simulink model "KUKA_LBR_Simulink_model_flatness_based_control"  (R2017a)
settings: Solver=VariableStepAuto  StartTime=0.0  StopTime=T  RelTol=1e-3
InitFcn:
  | main
values from neighbouring files (symbols this model uses):
  elbowAngle = elbowAngle * pi/180    (= 0)    [KUKA_LBR_init.m]    (also in Untitled2.m)
  KAnaJacNum = [k_ind 0 0 0 0 0 ;                 0  k_ind 0 0 0 0 ;                    0 0 k_ind 0 0 0 ;                      0 0 0 k_ind 0 0 ;                        0 0 0 0 k_ind 0 ;                          0 0 0 0 0 k_ind ;                            ]    [KUKA_LBR_init.m]
  Kuka_LBR_param_simu = Simulink.Parameter(Kuka_LBR_param_simu)    [KUKA_LBR_init.m]
  KUKA_LBR_x0 = [x1_0 x2_0 x3_0 x4_0 x5_0 x6_0 x7_0 x8_0 x9_0 x10_0 x11_0 x12_0 x13_0 x14_0]    [KUKA_LBR_init.m]
  rpyDes = rpyDes * pi/180    [KUKA_LBR_init.m]    (also in Untitled2.m)
  T = 0.5    [KUKA_LBR_init.m]
  vecGlobalConfig = [1; 1; 1]    [KUKA_LBR_init.m]    (also in Untitled2.m = [1, 1, 1])
undefined symbols (not defined in the file or in its folder): Kuka_LBR_param
(part 2 of 19)

== matlab function KUKA_LBR_Simulink_model_flatness_based_control/KUKUA_LBR_inverse_differentiell_kinematic ==
  data: vecJointPosDes_ input; rpyDes_ input; vecPosDes_ input; vecVelDes_ input; vecAccDes_ input; vecJointVelReal_ input; vecPosReal_ input; Kuka_LBR_param_ input; vecJointPos output; vecJointVel output; vecJointAcc output; KAnaJacP_ input; KAnaJacD_ input
function [vecJointPos,vecJointVel,vecJointAcc] = KUKUA_LBR_inverse_differentiell_kinematic(vecJointPosDes_,rpyDes_,vecPosDes_, vecVelDes_, vecAccDes_,vecJointVelReal_,vecPosReal_,Kuka_LBR_param_,KAnaJacP_,KAnaJacD_)

 
q1 = vecJointPosDes_(1,1) * pi/180;
q2 = vecJointPosDes_(1,2) * pi/180;
q3 = vecJointPosDes_(1,3) * pi/180;
q4 = vecJointPosDes_(1,4) * pi/180;
q5 = vecJointPosDes_(1,5) * pi/180;
q6 = vecJointPosDes_(1,6) * pi/180;
q7 = vecJointPosDes_(1,7) * pi/180;


Jxe11 = (-1).*Kuka_LBR_param_.dblLink23Len.*sin(q1).*sin(q2)+Kuka_LBR_param_.dblLink45Len.*((-1).*cos(q4).*sin(q1).*sin(q2)+(-1) ...
  .*((-1).*cos(q2).*cos(q3).*sin(q1)+(-1).*cos(q1).*sin(q3)).*sin(q4))+ ...
  Kuka_LBR_param_.dblLink67Len.*((-1).*cos(q6).*(cos(q4).*sin(q1).*sin(q2)+((-1).*cos(q2).*cos(q3) ...
  .*sin(q1)+(-1).*cos(q1).*sin(q3)).*sin(q4))+(cos(q5).*(cos(q4).*((-1).* ...
  cos(q2).*cos(q3).*sin(q1)+(-1).*cos(q1).*sin(q3))+(-1).*sin(q1).*sin(q2) ...
  .*sin(q4))+((-1).*cos(q1).*cos(q3)+cos(q2).*sin(q1).*sin(q3)).*sin(q5)) ...
  .*sin(q6));
  
Jxe12 =  Kuka_LBR_param_.dblLink23Len.*cos(q1).*cos(q2)+Kuka_LBR_param_.dblLink45Len.*(cos(q1).*cos(q2).*cos(q4)+cos(q1) ...
  .*cos(q3).*sin(q2).*sin(q4))+Kuka_LBR_param_.dblLink67Len.*((-1).*cos(q6).*((-1).*cos(q1).*cos( ...
  q2).*cos(q4)+(-1).*cos(q1).*cos(q3).*sin(q2).*sin(q4))+(cos(q5).*((-1).* ...
  cos(q1).*cos(q3).*cos(q4).*sin(q2)+cos(q1).*cos(q2).*sin(q4))+cos(q1).* ...
  sin(q2).*sin(q3).*sin(q5)).*sin(q6));
  
Jxe13 = (-1).*Kuka_LBR_param_.dblLink45Len.*((-1).*cos(q3).*sin(q1)+ ...
  (-1).*cos(q1).*cos(q2).*sin(q3)).*sin(q4)+Kuka_LBR_param_.dblLink67Len.*((-1).*cos(q6).*((-1).* ...
  cos(q3).*sin(q1)+(-1).*cos(q1).*cos(q2).*sin(q3)).*sin(q4)+(cos(q4).* ...
  cos(q5).*((-1).*cos(q3).*sin(q1)+(-1).*cos(q1).*cos(q2).*sin(q3))+((-1) ...
  .*cos(q1).*cos(q2).*cos(q3)+sin(q1).*sin(q3)).*sin(q5)).*sin(q6));
  
Jxe14 = Kuka_LBR_param_.dblLink45Len.*( ...
  (-1).*cos(q4).*(cos(q1).*cos(q2).*cos(q3)+(-1).*sin(q1).*sin(q3))+(-1).* ...
  cos(q1).*sin(q2).*sin(q4))+Kuka_LBR_param_.dblLink67Len.*((-1).*cos(q6).*(cos(q4).*(cos(q1).*cos( ...
  q2).*cos(q3)+(-1).*sin(q1).*sin(q3))+cos(q1).*sin(q2).*sin(q4))+cos(q5) ...
  .*(cos(q1).*cos(q4).*sin(q2)+(-1).*(cos(q1).*cos(q2).*cos(q3)+(-1).*sin( ...
  q1).*sin(q3)).*sin(q4)).*sin(q6));
  
Jxe15 = Kuka_LBR_param_.dblLink67Len.*(cos(q5).*((-1).*cos(q3).*sin(q1) ...
  +(-1).*cos(q1).*cos(q2).*sin(q3))+(-1).*(cos(q4).*(cos(q1).*cos(q2).* ...
  cos(q3)+(-1).*sin(q1).*sin(q3))+cos(q1).*sin(q2).*sin(q4)).*sin(q5)).* ...
  sin(q6);
  
Jxe16 = Kuka_LBR_param_.dblLink67Len.*(cos(q6).*(cos(q5).*(cos(q4).*(cos(q1).*cos(q2).*cos(q3)+( ...
  -1).*sin(q1).*sin(q3))+cos(q1).*sin(q2).*sin(q4))+((-1).*cos(q3).*sin( ...
  q1)+(-1).*cos(q1).*cos(q2).*sin(q3)).*sin(q5))+((-1).*cos(q1).*cos(q4).* ...
  sin(q2)+(cos(q1).*cos(q2).*cos(q3)+(-1).*sin(q1).*sin(q3)).*sin(q4)).* ...
  sin(q6));
  
 Jxe17= 0;
  
 Jxe21 = Kuka_LBR_param_.dblLink23Len.*cos(q1).*sin(q2)+Kuka_LBR_param_.dblLink45Len.*(cos(q1).*cos(q4).*sin(q2)+(-1).*( ...
  cos(q1).*cos(q2).*cos(q3)+(-1).*sin(q1).*sin(q3)).*sin(q4))+Kuka_LBR_param_.dblLink67Len.*((-1).* ...
  cos(q6).*((-1).*cos(q1).*cos(q4).*sin(q2)+(cos(q1).*cos(q2).*cos(q3)+( ...
  -1).*sin(q1).*sin(q3)).*sin(q4))+(cos(q5).*(cos(q4).*(cos(q1).*cos(q2).* ...
  cos(q3)+(-1).*sin(q1).*sin(q3))+cos(q1).*sin(q2).*sin(q4))+((-1).*cos( ...
  q3).*sin(q1)+(-1).*cos(q1).*cos(q2).*sin(q3)).*sin(q5)).*sin(q6));
  
  Jxe22 = Kuka_LBR_param_.dblLink23Len.* ...
  cos(q2).*sin(q1)+Kuka_LBR_param_.dblLink45Len.*(cos(q2).*cos(q4).*sin(q1)+cos(q3).*sin(q1).*sin( ...
  q2).*sin(q4))+Kuka_LBR_param_.dblLink67Len.*((-1).*cos(q6).*((-1).*cos(q2).*cos(q4).*sin(q1)+(-1) ...
  .*cos(q3).*sin(q1).*sin(q2).*sin(q4))+(cos(q5).*((-1).*cos(q3).*cos(q4) ...
  .*sin(q1).*sin(q2)+cos(q2).*sin(q1).*sin(q4))+sin(q1).*sin(q2).*sin(q3) ...
  .*sin(q5)).*sin(q6));
  
  Jxe23 = (-1).*Kuka_LBR_param_.dblLink45Len.*(cos(q1).*cos(q3)+(-1).*cos(q2).*sin(q1) ...
  .*sin(q3)).*sin(q4)+Kuka_LBR_param_.dblLink67Len.*((-1).*cos(q6).*(cos(q1).*cos(q3)+(-1).*cos(q2) ...
  .*sin(q1).*sin(q3)).*sin(q4)+(cos(q4).*cos(q5).*(cos(q1).*cos(q3)+(-1).* ...
  cos(q2).*sin(q1).*sin(q3))+((-1).*cos(q2).*cos(q3).*sin(q1)+(-1).*cos( ...
  q1).*sin(q3)).*sin(q5)).*sin(q6));
  
  Jxe24 = Kuka_LBR_param_.dblLink45Len.*((-1).*cos(q4).*(cos(q2).*cos(q3) ...
  .*sin(q1)+cos(q1).*sin(q3))+(-1).*sin(q1).*sin(q2).*sin(q4))+Kuka_LBR_param_.dblLink67Len.*((-1) ...
  .*cos(q6).*(cos(q4).*(cos(q2).*cos(q3).*sin(q1)+cos(q1).*sin(q3))+sin( ...
  q1).*sin(q2).*sin(q4))+cos(q5).*(cos(q4).*sin(q1).*sin(q2)+(-1).*(cos( ...
  q2).*cos(q3).*sin(q1)+cos(q1).*sin(q3)).*sin(q4)).*sin(q6));
  
  Jxe25 = Kuka_LBR_param_.dblLink67Len.*(cos( ...
  q5).*(cos(q1).*cos(q3)+(-1).*cos(q2).*sin(q1).*sin(q3))+(-1).*(cos(q4).* ...
  (cos(q2).*cos(q3).*sin(q1)+cos(q1).*sin(q3))+sin(q1).*sin(q2).*sin(q4)) ...
  .*sin(q5)).*sin(q6);
  
  Jxe26 = Kuka_LBR_param_.dblLink67Len.*(cos(q6).*(cos(q5).*(cos(q4).*(cos(q2).*cos(q3) ...
  .*sin(q1)+cos(q1).*sin(q3))+sin(q1).*sin(q2).*sin(q4))+(cos(q1).*cos(q3) ...
  +(-1).*cos(q2).*sin(q1).*sin(q3)).*sin(q5))+((-1).*cos(q4).*sin(q1).* ...
  sin(q2)+(cos(q2).*cos(q3).*sin(q1)+cos(q1).*sin(q3)).*sin(q4)).*sin(q6)); ...
  
  Jxe27 = 0;
  
  Jxe31 = 0;
  
  Jxe32 = (-1).*Kuka_LBR_param_.dblLink23Len.*sin(q2)+Kuka_LBR_param_.dblLink45Len.*((-1).*cos(q4).*sin(q2)+cos(q2).*cos(q3).* ...
  sin(q4))+Kuka_LBR_param_.dblLink67Len.*((-1).*cos(q6).*(cos(q4).*sin(q2)+(-1).*cos(q2).*cos(q3).* ...
  sin(q4))+(cos(q5).*((-1).*cos(q2).*cos(q3).*cos(q4)+(-1).*sin(q2).*sin( ...
  q4))+cos(q2).*sin(q3).*sin(q5)).*sin(q6));
  
  Jxe33 = (-1).*Kuka_LBR_param_.dblLink45Len.*sin(q2).*sin(q3).* ...
  sin(q4)+Kuka_LBR_param_.dblLink67Len.*((-1).*cos(q6).*sin(q2).*sin(q3).*sin(q4)+(cos(q4).*cos(q5) ...
  .*sin(q2).*sin(q3)+cos(q3).*sin(q2).*sin(q5)).*sin(q6));
  
  Jxe34 = Kuka_LBR_param_.dblLink45Len.*(cos(q3).* ...
  cos(q4).*sin(q2)+(-1).*cos(q2).*sin(q4))+Kuka_LBR_param_.dblLink67Len.*((-1).*cos(q6).*((-1).* ...
  cos(q3).*cos(q4).*sin(q2)+cos(q2).*sin(q4))+cos(q5).*(cos(q2).*cos(q4)+ ...
  cos(q3).*sin(q2).*sin(q4)).*sin(q6));
  
  Jxe35 = Kuka_LBR_param_.dblLink67Len.*(cos(q5).*sin(q2).*sin(q3)+( ...
  -1).*((-1).*cos(q3).*cos(q4).*sin(q2)+cos(q2).*sin(q4)).*sin(q5)).*sin( ...
  q6);
  
  Jxe36 = Kuka_LBR_param_.dblLink67Len.*(cos(q6).*(cos(q5).*((-1).*cos(q3).*cos(q4).*sin(q2)+cos(q2).* ...
  sin(q4))+sin(q2).*sin(q3).*sin(q5))+((-1).*cos(q2).*cos(q4)+(-1).*cos( ...
  q3).*sin(q2).*sin(q4)).*sin(q6));
  
  Jxe37 = 0;
  
  Jxe41 = (1+(-1).*(cos(q7).*(cos(q6).*(cos(q5) ...
  .*(cos(q4).*(cos(q1).*cos(q2).*cos(q3)+(-1).*sin(q1).*sin(q3))+cos(q1).* ...
  sin(q2).*sin(q4))+((-1).*cos(q3).*sin(q1)+(-1).*cos(q1).*cos(q2).*sin( ...
  q3)).*sin(q5))+((-1).*cos(q1).*cos(q4).*sin(q2)+(cos(q1).*cos(q2).*cos( ...
  q3)+(-1).*sin(q1).*sin(q3)).*sin(q4)).*sin(q6))+(cos(q5).*((-1).*cos(q3) ...
  .*sin(q1)+(-1).*cos(q1).*cos(q2).*sin(q3))+(-1).*(cos(q4).*(cos(q1).* ...
  cos(q2).*cos(q3)+(-1).*sin(q1).*sin(q3))+cos(q1).*sin(q2).*sin(q4)).* ...
  sin(q5)).*sin(q7)).^(-2).*(cos(q7).*(cos(q6).*(cos(q5).*(cos(q4).*((-1) ...
  .*cos(q2).*cos(q3).*sin(q1)+(-1).*cos(q1).*sin(q3))+(-1).*sin(q1).*sin( ...
  q2).*sin(q4))+((-1).*cos(q1).*cos(q3)+cos(q2).*sin(q1).*sin(q3)).*sin( ...
  q5))+(cos(q4).*sin(q1).*sin(q2)+((-1).*cos(q2).*cos(q3).*sin(q1)+(-1).* ...
  cos(q1).*sin(q3)).*sin(q4)).*sin(q6))+(cos(q5).*((-1).*cos(q1).*cos(q3)+ ...
  cos(q2).*sin(q1).*sin(q3))+(-1).*(cos(q4).*((-1).*cos(q2).*cos(q3).*sin( ...
  q1)+(-1).*cos(q1).*sin(q3))+(-1).*sin(q1).*sin(q2).*sin(q4)).*sin(q5)).* ...
  sin(q7)).*(cos(q7).*(cos(q6).*(cos(q5).*(cos(q4).*(cos(q2).*cos(q3).* ...
  sin(q1)+cos(q1).*sin(q3))+sin(q1).*sin(q2).*sin(q4))+(cos(q1).*cos(q3)+( ...
  -1).*cos(q2).*sin(q1).*sin(q3)).*sin(q5))+((-1).*cos(q4).*sin(q1).*sin( ...
  q2)+(cos(q2).*cos(q3).*sin(q1)+cos(q1).*sin(q3)).*sin(q4)).*sin(q6))+( ...
  cos(q5).*(cos(q1).*cos(q3)+(-1).*cos(q2).*sin(q1).*sin(q3))+(-1).*(cos( ...
  q4).*(cos(q2).*cos(q3).*sin(q1)+cos(q1).*sin(q3))+sin(q1).*sin(q2).*sin( ...
  q4)).*sin(q5)).*sin(q7)))*(1+(cos(q7).*(cos(q6).*(cos(q5).*(cos(q4).*( ...
  cos(q1).*cos(q2).*cos(q3)+(-1).*sin(q1).*sin(q3))+cos(q1).*sin(q2).*sin( ...
  q4))+((-1).*cos(q3).*sin(q1)+(-1).*cos(q1).*cos(q2).*sin(q3)).*sin(q5))+ ...
  ((-1).*cos(q1).*cos(q4).*sin(q2)+(cos(q1).*cos(q2).*cos(q3)+(-1).*sin( ...
  q1).*sin(q3)).*sin(q4)).*sin(q6))+(cos(q5).*((-1).*cos(q3).*sin(q1)+(-1) ...
  .*cos(q1).*cos(q2).*sin(q3))+(-1).*(cos(q4).*(cos(q1).*cos(q2).*cos(q3)+ ...
  (-1).*sin(q1).*sin(q3))+cos(q1).*sin(q2).*sin(q4)).*sin(q5)).*sin(q7)) ...
  .^(-2).*(cos(q7).*(cos(q6).*(cos(q5).*(cos(q4).*(cos(q2).*cos(q3).*sin( ...
  q1)+cos(q1).*sin(q3))+sin(q1).*sin(q2).*sin(q4))+(cos(q1).*cos(q3)+(-1) ...
  .*cos(q2).*sin(q1).*sin(q3)).*sin(q5))+((-1).*cos(q4).*sin(q1).*sin(q2)+ ...
  (cos(q2).*cos(q3).*sin(q1)+cos(q1).*sin(q3)).*sin(q4)).*sin(q6))+(cos( ...
  q5).*(cos(q1).*cos(q3)+(-1).*cos(q2).*sin(q1).*sin(q3))+(-1).*(cos(q4).* ...
  (cos(q2).*cos(q3).*sin(q1)+cos(q1).*sin(q3))+sin(q1).*sin(q2).*sin(q4)) ...
  .*sin(q5)).*sin(q7)).^2).^(-1);
  
  Jxe42 = ((cos(q7).*(cos(q6).*(cos(q5).*((-1).* ...
  cos(q3).*cos(q4).*sin(q1).*sin(q2)+cos(q2).*sin(q1).*sin(q4))+sin(q1).* ...
  sin(q2).*sin(q3).*sin(q5))+((-1).*cos(q2).*cos(q4).*sin(q1)+(-1).*cos( ...
  q3).*sin(q1).*sin(q2).*sin(q4)).*sin(q6))+(cos(q5).*sin(q1).*sin(q2).* ...
  sin(q3)+(-1).*((-1).*cos(q3).*cos(q4).*sin(q1).*sin(q2)+cos(q2).*sin(q1) ...
  .*sin(q4)).*sin(q5)).*sin(q7)).*(cos(q7).*(cos(q6).*(cos(q5).*(cos(q4).* ...
  (cos(q1).*cos(q2).*cos(q3)+(-1).*sin(q1).*sin(q3))+cos(q1).*sin(q2).* ...
  sin(q4))+((-1).*cos(q3).*sin(q1)+(-1).*cos(q1).*cos(q2).*sin(q3)).*sin( ...
  q5))+((-1).*cos(q1).*cos(q4).*sin(q2)+(cos(q1).*cos(q2).*cos(q3)+(-1).* ...
  sin(q1).*sin(q3)).*sin(q4)).*sin(q6))+(cos(q5).*((-1).*cos(q3).*sin(q1)+ ...
  (-1).*cos(q1).*cos(q2).*sin(q3))+(-1).*(cos(q4).*(cos(q1).*cos(q2).*cos( ...
  q3)+(-1).*sin(q1).*sin(q3))+cos(q1).*sin(q2).*sin(q4)).*sin(q5)).*sin( ...
  q7)).^(-1)+(-1).*(cos(q7).*(cos(q6).*(cos(q5).*((-1).*cos(q1).*cos(q3).* ...
  cos(q4).*sin(q2)+cos(q1).*cos(q2).*sin(q4))+cos(q1).*sin(q2).*sin(q3).* ...
  sin(q5))+((-1).*cos(q1).*cos(q2).*cos(q4)+(-1).*cos(q1).*cos(q3).*sin( ...
  q2).*sin(q4)).*sin(q6))+(cos(q1).*cos(q5).*sin(q2).*sin(q3)+(-1).*((-1) ...
  .*cos(q1).*cos(q3).*cos(q4).*sin(q2)+cos(q1).*cos(q2).*sin(q4)).*sin(q5) ...
  ).*sin(q7)).*(cos(q7).*(cos(q6).*(cos(q5).*(cos(q4).*(cos(q1).*cos(q2).* ...
  cos(q3)+(-1).*sin(q1).*sin(q3))+cos(q1).*sin(q2).*sin(q4))+((-1).*cos( ...
  q3).*sin(q1)+(-1).*cos(q1).*cos(q2).*sin(q3)).*sin(q5))+((-1).*cos(q1).* ...
  cos(q4).*sin(q2)+(cos(q1).*cos(q2).*cos(q3)+(-1).*sin(q1).*sin(q3)).* ...
  sin(q4)).*sin(q6))+(cos(q5).*((-1).*cos(q3).*sin(q1)+(-1).*cos(q1).*cos( ...
  q2).*sin(q3))+(-1).*(cos(q4).*(cos(q1).*cos(q2).*cos(q3)+(-1).*sin(q1).* ...
  sin(q3))+cos(q1).*sin(q2).*sin(q4)).*sin(q5)).*sin(q7)).^(-2).*(cos(q7) ...
  .*(cos(q6).*(cos(q5).*(cos(q4).*(cos(q2).*cos(q3).*sin(q1)+cos(q1).*sin( ...
  q3))+sin(q1).*sin(q2).*sin(q4))+(cos(q1).*cos(q3)+(-1).*cos(q2).*sin(q1) ...
  .*sin(q3)).*sin(q5))+((-1).*cos(q4).*sin(q1).*sin(q2)+(cos(q2).*cos(q3) ...
  .*sin(q1)+cos(q1).*sin(q3)).*sin(q4)).*sin(q6))+(cos(q5).*(cos(q1).*cos( ...
  q3)+(-1).*cos(q2).*sin(q1).*sin(q3))+(-1).*(cos(q4).*(cos(q2).*cos(q3).* ...
  sin(q1)+cos(q1).*sin(q3))+sin(q1).*sin(q2).*sin(q4)).*sin(q5)).*sin(q7)) ...
  ).*(1+(cos(q7).*(cos(q6).*(cos(q5).*(cos(q4).*(cos(q1).*cos(q2).*cos(q3) ...
  +(-1).*sin(q1).*sin(q3))+cos(q1).*sin(q2).*sin(q4))+((-1).*cos(q3).*sin( ...
  q1)+(-1).*cos(q1).*cos(q2).*sin(q3)).*sin(q5))+((-1).*cos(q1).*cos(q4).* ...
  sin(q2)+(cos(q1).*cos(q2).*cos(q3)+(-1).*sin(q1).*sin(q3)).*sin(q4)).* ...
  sin(q6))+(cos(q5).*((-1).*cos(q3).*sin(q1)+(-1).*cos(q1).*cos(q2).*sin( ...
  q3))+(-1).*(cos(q4).*(cos(q1).*cos(q2).*cos(q3)+(-1).*sin(q1).*sin(q3))+ ...
  cos(q1).*sin(q2).*sin(q4)).*sin(q5)).*sin(q7)).^(-2).*(cos(q7).*(cos(q6) ...
  .*(cos(q5).*(cos(q4).*(cos(q2).*cos(q3).*sin(q1)+cos(q1).*sin(q3))+sin( ...
  q1).*sin(q2).*sin(q4))+(cos(q1).*cos(q3)+(-1).*cos(q2).*sin(q1).*sin(q3) ...
  ).*sin(q5))+((-1).*cos(q4).*sin(q1).*sin(q2)+(cos(q2).*cos(q3).*sin(q1)+ ...
  cos(q1).*sin(q3)).*sin(q4)).*sin(q6))+(cos(q5).*(cos(q1).*cos(q3)+(-1).* ...
  cos(q2).*sin(q1).*sin(q3))+(-1).*(cos(q4).*(cos(q2).*cos(q3).*sin(q1)+ ...
  cos(q1).*sin(q3))+sin(q1).*sin(q2).*sin(q4)).*sin(q5)).*sin(q7)).^2).^( ...
  -1);
  
  Jxe43 = ((cos(q7).*(cos(q6).*(cos(q4).*cos(q5).*(cos(q1).*cos(q3)+(-1).*cos( ...
  q2).*sin(q1).*sin(q3))+((-1).*cos(q2).*cos(q3).*sin(q1)+(-1).*cos(q1).* ...
  sin(q3)).*sin(q5))+(cos(q1).*cos(q3)+(-1).*cos(q2).*sin(q1).*sin(q3)).* ...
  sin(q4).*sin(q6))+(cos(q5).*((-1).*cos(q2).*cos(q3).*sin(q1)+(-1).*cos( ...
  q1).*sin(q3))+(-1).*cos(q4).*(cos(q1).*cos(q3)+(-1).*cos(q2).*sin(q1).* ...
  sin(q3)).*sin(q5)).*sin(q7)).*(cos(q7).*(cos(q6).*(cos(q5).*(cos(q4).*( ...
  cos(q1).*cos(q2).*cos(q3)+(-1).*sin(q1).*sin(q3))+cos(q1).*sin(q2).*sin( ...
  q4))+((-1).*cos(q3).*sin(q1)+(-1).*cos(q1).*cos(q2).*sin(q3)).*sin(q5))+ ...
  ((-1).*cos(q1).*cos(q4).*sin(q2)+(cos(q1).*cos(q2).*cos(q3)+(-1).*sin( ...
  q1).*sin(q3)).*sin(q4)).*sin(q6))+(cos(q5).*((-1).*cos(q3).*sin(q1)+(-1) ...
  .*cos(q1).*cos(q2).*sin(q3))+(-1).*(cos(q4).*(cos(q1).*cos(q2).*cos(q3)+ ...
  (-1).*sin(q1).*sin(q3))+cos(q1).*sin(q2).*sin(q4)).*sin(q5)).*sin(q7)) ...
  .^(-1)+(-1).*(cos(q7).*(cos(q6).*(cos(q4).*cos(q5).*((-1).*cos(q3).*sin( ...
  q1)+(-1).*cos(q1).*cos(q2).*sin(q3))+((-1).*cos(q1).*cos(q2).*cos(q3)+ ...
  sin(q1).*sin(q3)).*sin(q5))+((-1).*cos(q3).*sin(q1)+(-1).*cos(q1).*cos( ...
  q2).*sin(q3)).*sin(q4).*sin(q6))+(cos(q5).*((-1).*cos(q1).*cos(q2).*cos( ...
  q3)+sin(q1).*sin(q3))+(-1).*cos(q4).*((-1).*cos(q3).*sin(q1)+(-1).*cos( ...
  q1).*cos(q2).*sin(q3)).*sin(q5)).*sin(q7)).*(cos(q7).*(cos(q6).*(cos(q5) ...
  .*(cos(q4).*(cos(q1).*cos(q2).*cos(q3)+(-1).*sin(q1).*sin(q3))+cos(q1).* ...
  sin(q2).*sin(q4))+((-1).*cos(q3).*sin(q1)+(-1).*cos(q1).*cos(q2).*sin( ...
  q3)).*sin(q5))+((-1).*cos(q1).*cos(q4).*sin(q2)+(cos(q1).*cos(q2).*cos( ...
  q3)+(-1).*sin(q1).*sin(q3)).*sin(q4)).*sin(q6))+(cos(q5).*((-1).*cos(q3) ...
  .*sin(q1)+(-1).*cos(q1).*cos(q2).*sin(q3))+(-1).*(cos(q4).*(cos(q1).* ...
  cos(q2).*cos(q3)+(-1).*sin(q1).*sin(q3))+cos(q1).*sin(q2).*sin(q4)).* ...
  sin(q5)).*sin(q7)).^(-2).*(cos(q7).*(cos(q6).*(cos(q5).*(cos(q4).*(cos( ...
  q2).*cos(q3).*sin(q1)+cos(q1).*sin(q3))+sin(q1).*sin(q2).*sin(q4))+(cos( ...
  q1).*cos(q3)+(-1).*cos(q2).*sin(q1).*sin(q3)).*sin(q5))+((-1).*cos(q4).* ...
  sin(q1).*sin(q2)+(cos(q2).*cos(q3).*sin(q1)+cos(q1).*sin(q3)).*sin(q4)) ...
  .*sin(q6))+(cos(q5).*(cos(q1).*cos(q3)+(-1).*cos(q2).*sin(q1).*sin(q3))+ ...
  (-1).*(cos(q4).*(cos(q2).*cos(q3).*sin(q1)+cos(q1).*sin(q3))+sin(q1).* ...
  sin(q2).*sin(q4)).*sin(q5)).*sin(q7))).*(1+(cos(q7).*(cos(q6).*(cos(q5) ...
  .*(cos(q4).*(cos(q1).*cos(q2).*cos(q3)+(-1).*sin(q1).*sin(q3))+cos(q1).* ...
  sin(q2).*sin(q4))+((-1).*cos(q3).*sin(q1)+(-1).*cos(q1).*cos(q2).*sin( ...
  q3)).*sin(q5))+((-1).*cos(q1).*cos(q4).*sin(q2)+(cos(q1).*cos(q2).*cos( ...
  q3)+(-1).*sin(q1).*sin(q3)).*sin(q4)).*sin(q6))+(cos(q5).*((-1).*cos(q3) ...
  .*sin(q1)+(-1).*cos(q1).*cos(q2).*sin(q3))+(-1).*(cos(q4).*(cos(q1).* ...
  cos(q2).*cos(q3)+(-1).*sin(q1).*sin(q3))+cos(q1).*sin(q2).*sin(q4)).* ...
  sin(q5)).*sin(q7)).^(-2).*(cos(q7).*(cos(q6).*(cos(q5).*(cos(q4).*(cos( ...
  q2).*cos(q3).*sin(q1)+cos(q1).*sin(q3))+sin(q1).*sin(q2).*sin(q4))+(cos( ...
  q1).*cos(q3)+(-1).*cos(q2).*sin(q1).*sin(q3)).*sin(q5))+((-1).*cos(q4).* ...
  sin(q1).*sin(q2)+(cos(q2).*cos(q3).*sin(q1)+cos(q1).*sin(q3)).*sin(q4)) ...
  .*sin(q6))+(cos(q5).*(cos(q1).*cos(q3)+(-1).*cos(q2).*sin(q1).*sin(q3))+ ...
  (-1).*(cos(q4).*(cos(q2).*cos(q3).*sin(q1)+cos(q1).*sin(q3))+sin(q1).* ...
  sin(q2).*sin(q4)).*sin(q5)).*sin(q7)).^2).^(-1);
  
  Jxe44 = ((cos(q7).*(cos(q5).* ...
  cos(q6).*(cos(q4).*sin(q1).*sin(q2)+(-1).*(cos(q2).*cos(q3).*sin(q1)+ ...
  cos(q1).*sin(q3)).*sin(q4))+(cos(q4).*(cos(q2).*cos(q3).*sin(q1)+cos(q1) ...
  .*sin(q3))+sin(q1).*sin(q2).*sin(q4)).*sin(q6))+(-1).*(cos(q4).*sin(q1) ...
  .*sin(q2)+(-1).*(cos(q2).*cos(q3).*sin(q1)+cos(q1).*sin(q3)).*sin(q4)).* ...
  sin(q5).*sin(q7)).*(cos(q7).*(cos(q6).*(cos(q5).*(cos(q4).*(cos(q1).* ...
  cos(q2).*cos(q3)+(-1).*sin(q1).*sin(q3))+cos(q1).*sin(q2).*sin(q4))+(( ...
  -1).*cos(q3).*sin(q1)+(-1).*cos(q1).*cos(q2).*sin(q3)).*sin(q5))+((-1).* ...
  cos(q1).*cos(q4).*sin(q2)+(cos(q1).*cos(q2).*cos(q3)+(-1).*sin(q1).*sin( ...
  q3)).*sin(q4)).*sin(q6))+(cos(q5).*((-1).*cos(q3).*sin(q1)+(-1).*cos(q1) ...
  .*cos(q2).*sin(q3))+(-1).*(cos(q4).*(cos(q1).*cos(q2).*cos(q3)+(-1).* ...
  sin(q1).*sin(q3))+cos(q1).*sin(q2).*sin(q4)).*sin(q5)).*sin(q7)).^(-1)+( ...
  -1).*(cos(q7).*(cos(q5).*cos(q6).*(cos(q1).*cos(q4).*sin(q2)+(-1).*(cos( ...
  q1).*cos(q2).*cos(q3)+(-1).*sin(q1).*sin(q3)).*sin(q4))+(cos(q4).*(cos( ...
  q1).*cos(q2).*cos(q3)+(-1).*sin(q1).*sin(q3))+cos(q1).*sin(q2).*sin(q4)) ...
  .*sin(q6))+(-1).*(cos(q1).*cos(q4).*sin(q2)+(-1).*(cos(q1).*cos(q2).* ...
  cos(q3)+(-1).*sin(q1).*sin(q3)).*sin(q4)).*sin(q5).*sin(q7)).*(cos(q7).* ...
  (cos(q6).*(cos(q5).*(cos(q4).*(cos(q1).*cos(q2).*cos(q3)+(-1).*sin(q1).* ...
  sin(q3))+cos(q1).*sin(q2).*sin(q4))+((-1).*cos(q3).*sin(q1)+(-1).*cos( ...
  q1).*cos(q2).*sin(q3)).*sin(q5))+((-1).*cos(q1).*cos(q4).*sin(q2)+(cos( ...
  q1).*cos(q2).*cos(q3)+(-1).*sin(q1).*sin(q3)).*sin(q4)).*sin(q6))+(cos( ...
  q5).*((-1).*cos(q3).*sin(q1)+(-1).*cos(q1).*cos(q2).*sin(q3))+(-1).*( ...
  cos(q4).*(cos(q1).*cos(q2).*cos(q3)+(-1).*sin(q1).*sin(q3))+cos(q1).* ...
  sin(q2).*sin(q4)).*sin(q5)).*sin(q7)).^(-2).*(cos(q7).*(cos(q6).*(cos( ...
  q5).*(cos(q4).*(cos(q2).*cos(q3).*sin(q1)+cos(q1).*sin(q3))+sin(q1).* ...
  sin(q2).*sin(q4))+(cos(q1).*cos(q3)+(-1).*cos(q2).*sin(q1).*sin(q3)).* ...
  sin(q5))+((-1).*cos(q4).*sin(q1).*sin(q2)+(cos(q2).*cos(q3).*sin(q1)+ ...
  cos(q1).*sin(q3)).*sin(q4)).*sin(q6))+(cos(q5).*(cos(q1).*cos(q3)+(-1).* ...
  cos(q2).*sin(q1).*sin(q3))+(-1).*(cos(q4).*(cos(q2).*cos(q3).*sin(q1)+ ...
  cos(q1).*sin(q3))+sin(q1).*sin(q2).*sin(q4)).*sin(q5)).*sin(q7))).*(1+( ...
  cos(q7).*(cos(q6).*(cos(q5).*(cos(q4).*(cos(q1).*cos(q2).*cos(q3)+(-1).* ...
  sin(q1).*sin(q3))+cos(q1).*sin(q2).*sin(q4))+((-1).*cos(q3).*sin(q1)+( ...
  -1).*cos(q1).*cos(q2).*sin(q3)).*sin(q5))+((-1).*cos(q1).*cos(q4).*sin( ...
  q2)+(cos(q1).*cos(q2).*cos(q3)+(-1).*sin(q1).*sin(q3)).*sin(q4)).*sin( ...
  q6))+(cos(q5).*((-1).*cos(q3).*sin(q1)+(-1).*cos(q1).*cos(q2).*sin(q3))+ ...
  (-1).*(cos(q4).*(cos(q1).*cos(q2).*cos(q3)+(-1).*sin(q1).*sin(q3))+cos( ...
  q1).*sin(q2).*sin(q4)).*sin(q5)).*sin(q7)).^(-2).*(cos(q7).*(cos(q6).*( ...
  cos(q5).*(cos(q4).*(cos(q2).*cos(q3).*sin(q1)+cos(q1).*sin(q3))+sin(q1) ...
  .*sin(q2).*sin(q4))+(cos(q1).*cos(q3)+(-1).*cos(q2).*sin(q1).*sin(q3)).* ...
  sin(q5))+((-1).*cos(q4).*sin(q1).*sin(q2)+(cos(q2).*cos(q3).*sin(q1)+ ...
  cos(q1).*sin(q3)).*sin(q4)).*sin(q6))+(cos(q5).*(cos(q1).*cos(q3)+(-1).* ...
  cos(q2).*sin(q1).*sin(q3))+(-1).*(cos(q4).*(cos(q2).*cos(q3).*sin(q1)+ ...
  cos(q1).*sin(q3))+sin(q1).*sin(q2).*sin(q4)).*sin(q5)).*sin(q7)).^2).^( ...
  -1);
  
  Jxe45 = ((cos(q6).*cos(q7).*(cos(q5).*(cos(q1).*cos(q3)+(-1).*cos(q2).*sin( ...
  q1).*sin(q3))+(-1).*(cos(q4).*(cos(q2).*cos(q3).*sin(q1)+cos(q1).*sin( ...
  q3))+sin(q1).*sin(q2).*sin(q4)).*sin(q5))+((-1).*cos(q5).*(cos(q4).*( ...
  cos(q2).*cos(q3).*sin(q1)+cos(q1).*sin(q3))+sin(q1).*sin(q2).*sin(q4))+( ...
  -1).*(cos(q1).*cos(q3)+(-1).*cos(q2).*sin(q1).*sin(q3)).*sin(q5)).*sin( ...
  q7)).*(cos(q7).*(cos(q6).*(cos(q5).*(cos(q4).*(cos(q1).*cos(q2).*cos(q3) ...
  +(-1).*sin(q1).*sin(q3))+cos(q1).*sin(q2).*sin(q4))+((-1).*cos(q3).*sin( ...
  q1)+(-1).*cos(q1).*cos(q2).*sin(q3)).*sin(q5))+((-1).*cos(q1).*cos(q4).* ...
  sin(q2)+(cos(q1).*cos(q2).*cos(q3)+(-1).*sin(q1).*sin(q3)).*sin(q4)).* ...
  sin(q6))+(cos(q5).*((-1).*cos(q3).*sin(q1)+(-1).*cos(q1).*cos(q2).*sin( ...
  q3))+(-1).*(cos(q4).*(cos(q1).*cos(q2).*cos(q3)+(-1).*sin(q1).*sin(q3))+ ...
  cos(q1).*sin(q2).*sin(q4)).*sin(q5)).*sin(q7)).^(-1)+(-1).*(cos(q6).* ...
  cos(q7).*(cos(q5).*((-1).*cos(q3).*sin(q1)+(-1).*cos(q1).*cos(q2).*sin( ...
  q3))+(-1).*(cos(q4).*(cos(q1).*cos(q2).*cos(q3)+(-1).*sin(q1).*sin(q3))+ ...
  cos(q1).*sin(q2).*sin(q4)).*sin(q5))+((-1).*cos(q5).*(cos(q4).*(cos(q1) ...
  .*cos(q2).*cos(q3)+(-1).*sin(q1).*sin(q3))+cos(q1).*sin(q2).*sin(q4))+( ...
  -1).*((-1).*cos(q3).*sin(q1)+(-1).*cos(q1).*cos(q2).*sin(q3)).*sin(q5)) ...
  .*sin(q7)).*(cos(q7).*(cos(q6).*(cos(q5).*(cos(q4).*(cos(q1).*cos(q2).* ...
  cos(q3)+(-1).*sin(q1).*sin(q3))+cos(q1).*sin(q2).*sin(q4))+((-1).*cos( ...
  q3).*sin(q1)+(-1).*cos(q1).*cos(q2).*sin(q3)).*sin(q5))+((-1).*cos(q1).* ...
  cos(q4).*sin(q2)+(cos(q1).*cos(q2).*cos(q3)+(-1).*sin(q1).*sin(q3)).* ...
  sin(q4)).*sin(q6))+(cos(q5).*((-1).*cos(q3).*sin(q1)+(-1).*cos(q1).*cos( ...
  q2).*sin(q3))+(-1).*(cos(q4).*(cos(q1).*cos(q2).*cos(q3)+(-1).*sin(q1).* ...
  sin(q3))+cos(q1).*sin(q2).*sin(q4)).*sin(q5)).*sin(q7)).^(-2).*(cos(q7) ...
  .*(cos(q6).*(cos(q5).*(cos(q4).*(cos(q2).*cos(q3).*sin(q1)+cos(q1).*sin( ...
  q3))+sin(q1).*sin(q2).*sin(q4))+(cos(q1).*cos(q3)+(-1).*cos(q2).*sin(q1) ...
  .*sin(q3)).*sin(q5))+((-1).*cos(q4).*sin(q1).*sin(q2)+(cos(q2).*cos(q3) ...
  .*sin(q1)+cos(q1).*sin(q3)).*sin(q4)).*sin(q6))+(cos(q5).*(cos(q1).*cos( ...
  q3)+(-1).*cos(q2).*sin(q1).*sin(q3))+(-1).*(cos(q4).*(cos(q2).*cos(q3).* ...
  sin(q1)+cos(q1).*sin(q3))+sin(q1).*sin(q2).*sin(q4)).*sin(q5)).*sin(q7)) ...
  )*(1+(cos(q7).*(cos(q6).*(cos(q5).*(cos(q4).*(cos(q1).*cos(q2).*cos(q3) ...
  +(-1).*sin(q1).*sin(q3))+cos(q1).*sin(q2).*sin(q4))+((-1).*cos(q3).*sin( ...
  q1)+(-1).*cos(q1).*cos(q2).*sin(q3)).*sin(q5))+((-1).*cos(q1).*cos(q4).* ...
  sin(q2)+(cos(q1).*cos(q2).*cos(q3)+(-1).*sin(q1).*sin(q3)).*sin(q4)).* ...
  sin(q6))+(cos(q5).*((-1).*cos(q3).*sin(q1)+(-1).*cos(q1).*cos(q2).*sin( ...
  q3))+(-1).*(cos(q4).*(cos(q1).*cos(q2).*cos(q3)+(-1).*sin(q1).*sin(q3))+ ...
  cos(q1).*sin(q2).*sin(q4)).*sin(q5)).*sin(q7)).^(-2).*(cos(q7).*(cos(q6) ...
  .*(cos(q5).*(cos(q4).*(cos(q2).*cos(q3).*sin(q1)+cos(q1).*sin(q3))+sin( ...
  q1).*sin(q2).*sin(q4))+(cos(q1).*cos(q3)+(-1).*cos(q2).*sin(q1).*sin(q3) ...
  ).*sin(q5))+((-1).*cos(q4).*sin(q1).*sin(q2)+(cos(q2).*cos(q3).*sin(q1)+ ...
  cos(q1).*sin(q3)).*sin(q4)).*sin(q6))+(cos(q5).*(cos(q1).*cos(q3)+(-1).* ...
  cos(q2).*sin(q1).*sin(q3))+(-1).*(cos(q4).*(cos(q2).*cos(q3).*sin(q1)+ ...
  cos(q1).*sin(q3))+sin(q1).*sin(q2).*sin(q4)).*sin(q5)).*sin(q7)).^2).^( ...
  -1);
  
  Jxe46 = (cos(q7).*(cos(q6).*((-1).*cos(q4).*sin(q1).*sin(q2)+(cos(q2).*cos( ...
  q3).*sin(q1)+cos(q1).*sin(q3)).*sin(q4))+(-1).*(cos(q5).*(cos(q4).*(cos( ...
  q2).*cos(q3).*sin(q1)+cos(q1).*sin(q3))+sin(q1).*sin(q2).*sin(q4))+(cos( ...
  q1).*cos(q3)+(-1).*cos(q2).*sin(q1).*sin(q3)).*sin(q5)).*sin(q6)).*(cos( ...
  q7).*(cos(q6).*(cos(q5).*(cos(q4).*(cos(q1).*cos(q2).*cos(q3)+(-1).*sin( ...
  q1).*sin(q3))+cos(q1).*sin(q2).*sin(q4))+((-1).*cos(q3).*sin(q1)+(-1).* ...
  cos(q1).*cos(q2).*sin(q3)).*sin(q5))+((-1).*cos(q1).*cos(q4).*sin(q2)+( ...
  cos(q1).*cos(q2).*cos(q3)+(-1).*sin(q1).*sin(q3)).*sin(q4)).*sin(q6))+( ...
  cos(q5).*((-1).*cos(q3).*sin(q1)+(-1).*cos(q1).*cos(q2).*sin(q3))+(-1).* ...
  (cos(q4).*(cos(q1).*cos(q2).*cos(q3)+(-1).*sin(q1).*sin(q3))+cos(q1).* ...
  sin(q2).*sin(q4)).*sin(q5)).*sin(q7)).^(-1)+(-1).*cos(q7).*(cos(q6).*(( ...
  -1).*cos(q1).*cos(q4).*sin(q2)+(cos(q1).*cos(q2).*cos(q3)+(-1).*sin(q1) ...
  .*sin(q3)).*sin(q4))+(-1).*(cos(q5).*(cos(q4).*(cos(q1).*cos(q2).*cos( ...
  q3)+(-1).*sin(q1).*sin(q3))+cos(q1).*sin(q2).*sin(q4))+((-1).*cos(q3).* ...
  sin(q1)+(-1).*cos(q1).*cos(q2).*sin(q3)).*sin(q5)).*sin(q6)).*(cos(q7).* ...
  (cos(q6).*(cos(q5).*(cos(q4).*(cos(q1).*cos(q2).*cos(q3)+(-1).*sin(q1).* ...
  sin(q3))+cos(q1).*sin(q2).*sin(q4))+((-1).*cos(q3).*sin(q1)+(-1).*cos( ...
  q1).*cos(q2).*sin(q3)).*sin(q5))+((-1).*cos(q1).*cos(q4).*sin(q2)+(cos( ...
  q1).*cos(q2).*cos(q3)+(-1).*sin(q1).*sin(q3)).*sin(q4)).*sin(q6))+(cos( ...
  q5).*((-1).*cos(q3).*sin(q1)+(-1).*cos(q1).*cos(q2).*sin(q3))+(-1).*( ...
  cos(q4).*(cos(q1).*cos(q2).*cos(q3)+(-1).*sin(q1).*sin(q3))+cos(q1).* ...
  sin(q2).*sin(q4)).*sin(q5)).*sin(q7)).^(-2).*(cos(q7).*(cos(q6).*(cos( ...
  q5).*(cos(q4).*(cos(q2).*cos(q3).*sin(q1)+cos(q1).*sin(q3))+sin(q1).* ...
  sin(q2).*sin(q4))+(cos(q1).*cos(q3)+(-1).*cos(q2).*sin(q1).*sin(q3)).* ...
  sin(q5))+((-1).*cos(q4).*sin(q1).*sin(q2)+(cos(q2).*cos(q3).*sin(q1)+ ...
  cos(q1).*sin(q3)).*sin(q4)).*sin(q6))+(cos(q5).*(cos(q1).*cos(q3)+(-1).* ...
  cos(q2).*sin(q1).*sin(q3))+(-1).*(cos(q4).*(cos(q2).*cos(q3).*sin(q1)+ ...
  cos(q1).*sin(q3))+sin(q1).*sin(q2).*sin(q4)).*sin(q5)).*sin(q7))).*(1+( ...
  cos(q7).*(cos(q6).*(cos(q5).*(cos(q4).*(cos(q1).*cos(q2).*cos(q3)+(-1).* ...
  sin(q1).*sin(q3))+cos(q1).*sin(q2).*sin(q4))+((-1).*cos(q3).*sin(q1)+( ...
  -1).*cos(q1).*cos(q2).*sin(q3)).*sin(q5))+((-1).*cos(q1).*cos(q4).*sin( ...
  q2)+(cos(q1).*cos(q2).*cos(q3)+(-1).*sin(q1).*sin(q3)).*sin(q4)).*sin( ...
  q6))+(cos(q5).*((-1).*cos(q3).*sin(q1)+(-1).*cos(q1).*cos(q2).*sin(q3))+ ...
  (-1).*(cos(q4).*(cos(q1).*cos(q2).*cos(q3)+(-1).*sin(q1).*sin(q3))+cos( ...
  q1).*sin(q2).*sin(q4)).*sin(q5)).*sin(q7)).^(-2).*(cos(q7).*(cos(q6).*( ...
  cos(q5).*(cos(q4).*(cos(q2).*cos(q3).*sin(q1)+cos(q1).*sin(q3))+sin(q1) ...
  .*sin(q2).*sin(q4))+(cos(q1).*cos(q3)+(-1).*cos(q2).*sin(q1).*sin(q3)).* ...
  sin(q5))+((-1).*cos(q4).*sin(q1).*sin(q2)+(cos(q2).*cos(q3).*sin(q1)+ ...
  cos(q1).*sin(q3)).*sin(q4)).*sin(q6))+(cos(q5).*(cos(q1).*cos(q3)+(-1).* ...
  cos(q2).*sin(q1).*sin(q3))+(-1).*(cos(q4).*(cos(q2).*cos(q3).*sin(q1)+ ...
  cos(q1).*sin(q3))+sin(q1).*sin(q2).*sin(q4)).*sin(q5)).*sin(q7)).^2).^( ...
  -1);
  
  Jxe47 = (1+(cos(q7).*(cos(q6).*(cos(q5).*(cos(q4).*(cos(q1).*cos(q2).*cos( ...
  q3)+(-1).*sin(q1).*sin(q3))+cos(q1).*sin(q2).*sin(q4))+((-1).*cos(q3).* ...
  sin(q1)+(-1).*cos(q1).*cos(q2).*sin(q3)).*sin(q5))+((-1).*cos(q1).*cos( ...
  q4).*sin(q2)+(cos(q1).*cos(q2).*cos(q3)+(-1).*sin(q1).*sin(q3)).*sin(q4) ...
  ).*sin(q6))+(cos(q5).*((-1).*cos(q3).*sin(q1)+(-1).*cos(q1).*cos(q2).* ...
  sin(q3))+(-1).*(cos(q4).*(cos(q1).*cos(q2).*cos(q3)+(-1).*sin(q1).*sin( ...
  q3))+cos(q1).*sin(q2).*sin(q4)).*sin(q5)).*sin(q7)).^(-2).*(cos(q7).*( ...
  cos(q6).*(cos(q5).*(cos(q4).*(cos(q2).*cos(q3).*sin(q1)+cos(q1).*sin(q3) ...
  )+sin(q1).*sin(q2).*sin(q4))+(cos(q1).*cos(q3)+(-1).*cos(q2).*sin(q1).* ...
  sin(q3)).*sin(q5))+((-1).*cos(q4).*sin(q1).*sin(q2)+(cos(q2).*cos(q3).* ...
  sin(q1)+cos(q1).*sin(q3)).*sin(q4)).*sin(q6))+(cos(q5).*(cos(q1).*cos( ...
  q3)+(-1).*cos(q2).*sin(q1).*sin(q3))+(-1).*(cos(q4).*(cos(q2).*cos(q3).* ...
  sin(q1)+cos(q1).*sin(q3))+sin(q1).*sin(q2).*sin(q4)).*sin(q5)).*sin(q7)) ...
  .^2).^(-1).*((cos(q7).*(cos(q6).*(cos(q5).*(cos(q4).*(cos(q1).*cos(q2).* ...
  cos(q3)+(-1).*sin(q1).*sin(q3))+cos(q1).*sin(q2).*sin(q4))+((-1).*cos( ...
  q3).*sin(q1)+(-1).*cos(q1).*cos(q2).*sin(q3)).*sin(q5))+((-1).*cos(q1).* ...
  cos(q4).*sin(q2)+(cos(q1).*cos(q2).*cos(q3)+(-1).*sin(q1).*sin(q3)).* ...
  sin(q4)).*sin(q6))+(cos(q5).*((-1).*cos(q3).*sin(q1)+(-1).*cos(q1).*cos( ...
  q2).*sin(q3))+(-1).*(cos(q4).*(cos(q1).*cos(q2).*cos(q3)+(-1).*sin(q1).* ...
  sin(q3))+cos(q1).*sin(q2).*sin(q4)).*sin(q5)).*sin(q7)).^(-1).*(cos(q7) ...
  .*(cos(q5).*(cos(q1).*cos(q3)+(-1).*cos(q2).*sin(q1).*sin(q3))+(-1).*( ...
  cos(q4).*(cos(q2).*cos(q3).*sin(q1)+cos(q1).*sin(q3))+sin(q1).*sin(q2).* ...
  sin(q4)).*sin(q5))+(-1).*(cos(q6).*(cos(q5).*(cos(q4).*(cos(q2).*cos(q3) ...
  .*sin(q1)+cos(q1).*sin(q3))+sin(q1).*sin(q2).*sin(q4))+(cos(q1).*cos(q3) ...
  +(-1).*cos(q2).*sin(q1).*sin(q3)).*sin(q5))+((-1).*cos(q4).*sin(q1).* ...
  sin(q2)+(cos(q2).*cos(q3).*sin(q1)+cos(q1).*sin(q3)).*sin(q4)).*sin(q6)) ...
  .*sin(q7))+(-1).*(cos(q7).*(cos(q6).*(cos(q5).*(cos(q4).*(cos(q1).*cos( ...
  q2).*cos(q3)+(-1).*sin(q1).*sin(q3))+cos(q1).*sin(q2).*sin(q4))+((-1).* ...
  cos(q3).*sin(q1)+(-1).*cos(q1).*cos(q2).*sin(q3)).*sin(q5))+((-1).*cos( ...
  q1).*cos(q4).*sin(q2)+(cos(q1).*cos(q2).*cos(q3)+(-1).*sin(q1).*sin(q3)) ...
  .*sin(q4)).*sin(q6))+(cos(q5).*((-1).*cos(q3).*sin(q1)+(-1).*cos(q1).* ...
  cos(q2).*sin(q3))+(-1).*(cos(q4).*(cos(q1).*cos(q2).*cos(q3)+(-1).*sin( ...
  q1).*sin(q3))+cos(q1).*sin(q2).*sin(q4)).*sin(q5)).*sin(q7)).^(-2).*( ...
  cos(q7).*(cos(q6).*(cos(q5).*(cos(q4).*(cos(q2).*cos(q3).*sin(q1)+cos( ...
  q1).*sin(q3))+sin(q1).*sin(q2).*sin(q4))+(cos(q1).*cos(q3)+(-1).*cos(q2) ...
  .*sin(q1).*sin(q3)).*sin(q5))+((-1).*cos(q4).*sin(q1).*sin(q2)+(cos(q2) ...
  .*cos(q3).*sin(q1)+cos(q1).*sin(q3)).*sin(q4)).*sin(q6))+(cos(q5).*(cos( ...
  q1).*cos(q3)+(-1).*cos(q2).*sin(q1).*sin(q3))+(-1).*(cos(q4).*(cos(q2).* ...
  cos(q3).*sin(q1)+cos(q1).*sin(q3))+sin(q1).*sin(q2).*sin(q4)).*sin(q5)) ...
  .*sin(q7)).*(cos(q7).*(cos(q5).*((-1).*cos(q3).*sin(q1)+(-1).*cos(q1).* ...
  cos(q2).*sin(q3))+(-1).*(cos(q4).*(cos(q1).*cos(q2).*cos(q3)+(-1).*sin( ...
  q1).*sin(q3))+cos(q1).*sin(q2).*sin(q4)).*sin(q5))+(-1).*(cos(q6).*(cos( ...
  q5).*(cos(q4).*(cos(q1).*cos(q2).*cos(q3)+(-1).*sin(q1).*sin(q3))+cos( ...
  q1).*sin(q2).*sin(q4))+((-1).*cos(q3).*sin(q1)+(-1).*cos(q1).*cos(q2).* ...
  sin(q3)).*sin(q5))+((-1).*cos(q1).*cos(q4).*sin(q2)+(cos(q1).*cos(q2).* ...
  cos(q3)+(-1).*sin(q1).*sin(q3)).*sin(q4)).*sin(q6)).*sin(q7)));
  
  Jxe51 = 0;
  
 Jxe52 = (1+( ...
  cos(q7).*(cos(q6).*(cos(q5).*((-1).*cos(q3).*cos(q4).*sin(q2)+cos(q2).* ...
  sin(q4))+sin(q2).*sin(q3).*sin(q5))+((-1).*cos(q2).*cos(q4)+(-1).*cos( ...
  q3).*sin(q2).*sin(q4)).*sin(q6))+(cos(q5).*sin(q2).*sin(q3)+(-1).*((-1) ...
  .*cos(q3).*cos(q4).*sin(q2)+cos(q2).*sin(q4)).*sin(q5)).*sin(q7)).^2.*(( ...
  (-1).*cos(q6).*((-1).*cos(q2).*cos(q4)+(-1).*cos(q3).*sin(q2).*sin(q4))+ ...
  (cos(q5).*((-1).*cos(q3).*cos(q4).*sin(q2)+cos(q2).*sin(q4))+sin(q2).* ...
  sin(q3).*sin(q5)).*sin(q6)).^2+(cos(q7).*(cos(q5).*sin(q2).*sin(q3)+(-1) ...
  .*((-1).*cos(q3).*cos(q4).*sin(q2)+cos(q2).*sin(q4)).*sin(q5))+(-1).*( ...
  cos(q6).*(cos(q5).*((-1).*cos(q3).*cos(q4).*sin(q2)+cos(q2).*sin(q4))+ ...
  sin(q2).*sin(q3).*sin(q5))+((-1).*cos(q2).*cos(q4)+(-1).*cos(q3).*sin( ...
  q2).*sin(q4)).*sin(q6)).*sin(q7)).^2).^(-1)).^(-1).*((-1/2).*(cos(q7).*( ...
  cos(q6).*(cos(q5).*((-1).*cos(q3).*cos(q4).*sin(q2)+cos(q2).*sin(q4))+ ...
  sin(q2).*sin(q3).*sin(q5))+((-1).*cos(q2).*cos(q4)+(-1).*cos(q3).*sin( ...
  q2).*sin(q4)).*sin(q6))+(cos(q5).*sin(q2).*sin(q3)+(-1).*((-1).*cos(q3) ...
  .*cos(q4).*sin(q2)+cos(q2).*sin(q4)).*sin(q5)).*sin(q7)).*(2.*((-1).* ...
  cos(q6).*(cos(q4).*sin(q2)+(-1).*cos(q2).*cos(q3).*sin(q4))+(cos(q5).*(( ...
  -1).*cos(q2).*cos(q3).*cos(q4)+(-1).*sin(q2).*sin(q4))+cos(q2).*sin(q3) ...
  .*sin(q5)).*sin(q6)).*((-1).*cos(q6).*((-1).*cos(q2).*cos(q4)+(-1).*cos( ...
  q3).*sin(q2).*sin(q4))+(cos(q5).*((-1).*cos(q3).*cos(q4).*sin(q2)+cos( ...
  q2).*sin(q4))+sin(q2).*sin(q3).*sin(q5)).*sin(q6))+2.*(cos(q7).*(cos(q2) ...
  .*cos(q5).*sin(q3)+(-1).*((-1).*cos(q2).*cos(q3).*cos(q4)+(-1).*sin(q2) ...
  .*sin(q4)).*sin(q5))+(-1).*(cos(q6).*(cos(q5).*((-1).*cos(q2).*cos(q3).* ...
  cos(q4)+(-1).*sin(q2).*sin(q4))+cos(q2).*sin(q3).*sin(q5))+(cos(q4).* ...
  sin(q2)+(-1).*cos(q2).*cos(q3).*sin(q4)).*sin(q6)).*sin(q7)).*(cos(q7).* ...
  (cos(q5).*sin(q2).*sin(q3)+(-1).*((-1).*cos(q3).*cos(q4).*sin(q2)+cos( ...
  q2).*sin(q4)).*sin(q5))+(-1).*(cos(q6).*(cos(q5).*((-1).*cos(q3).*cos( ...
  q4).*sin(q2)+cos(q2).*sin(q4))+sin(q2).*sin(q3).*sin(q5))+((-1).*cos(q2) ...
  .*cos(q4)+(-1).*cos(q3).*sin(q2).*sin(q4)).*sin(q6)).*sin(q7))).*(((-1) ...
  .*cos(q6).*((-1).*cos(q2).*cos(q4)+(-1).*cos(q3).*sin(q2).*sin(q4))+( ...
  cos(q5).*((-1).*cos(q3).*cos(q4).*sin(q2)+cos(q2).*sin(q4))+sin(q2).* ...
  sin(q3).*sin(q5)).*sin(q6)).^2+(cos(q7).*(cos(q5).*sin(q2).*sin(q3)+(-1) ...
  .*((-1).*cos(q3).*cos(q4).*sin(q2)+cos(q2).*sin(q4)).*sin(q5))+(-1).*( ...
  cos(q6).*(cos(q5).*((-1).*cos(q3).*cos(q4).*sin(q2)+cos(q2).*sin(q4))+ ...
  sin(q2).*sin(q3).*sin(q5))+((-1).*cos(q2).*cos(q4)+(-1).*cos(q3).*sin( ...
  q2).*sin(q4)).*sin(q6)).*sin(q7)).^2).^(-3/2)+(cos(q7).*(cos(q6).*(cos( ...
  q5).*((-1).*cos(q2).*cos(q3).*cos(q4)+(-1).*sin(q2).*sin(q4))+cos(q2).* ...
  sin(q3).*sin(q5))+(cos(q4).*sin(q2)+(-1).*cos(q2).*cos(q3).*sin(q4)).* ...
  sin(q6))+(cos(q2).*cos(q5).*sin(q3)+(-1).*((-1).*cos(q2).*cos(q3).*cos( ...
  q4)+(-1).*sin(q2).*sin(q4)).*sin(q5)).*sin(q7)).*(((-1).*cos(q6).*((-1) ...
  .*cos(q2).*cos(q4)+(-1).*cos(q3).*sin(q2).*sin(q4))+(cos(q5).*((-1).* ...
  cos(q3).*cos(q4).*sin(q2)+cos(q2).*sin(q4))+sin(q2).*sin(q3).*sin(q5)).* ...
  sin(q6)).^2+(cos(q7).*(cos(q5).*sin(q2).*sin(q3)+(-1).*((-1).*cos(q3).* ...
  cos(q4).*sin(q2)+cos(q2).*sin(q4)).*sin(q5))+(-1).*(cos(q6).*(cos(q5).*( ...
  (-1).*cos(q3).*cos(q4).*sin(q2)+cos(q2).*sin(q4))+sin(q2).*sin(q3).*sin( ...
  q5))+((-1).*cos(q2).*cos(q4)+(-1).*cos(q3).*sin(q2).*sin(q4)).*sin(q6)) ...
  .*sin(q7)).^2).^(-1/2));
  
  Jxe53 = (1+(cos(q7).*(cos(q6).*(cos(q5).*((-1).*cos(q3) ...
  .*cos(q4).*sin(q2)+cos(q2).*sin(q4))+sin(q2).*sin(q3).*sin(q5))+((-1).* ...
  cos(q2).*cos(q4)+(-1).*cos(q3).*sin(q2).*sin(q4)).*sin(q6))+(cos(q5).* ...
  sin(q2).*sin(q3)+(-1).*((-1).*cos(q3).*cos(q4).*sin(q2)+cos(q2).*sin(q4) ...
  ).*sin(q5)).*sin(q7)).^2.*(((-1).*cos(q6).*((-1).*cos(q2).*cos(q4)+(-1) ...
  .*cos(q3).*sin(q2).*sin(q4))+(cos(q5).*((-1).*cos(q3).*cos(q4).*sin(q2)+ ...
  cos(q2).*sin(q4))+sin(q2).*sin(q3).*sin(q5)).*sin(q6)).^2+(cos(q7).*( ...
  cos(q5).*sin(q2).*sin(q3)+(-1).*((-1).*cos(q3).*cos(q4).*sin(q2)+cos(q2) ...
  .*sin(q4)).*sin(q5))+(-1).*(cos(q6).*(cos(q5).*((-1).*cos(q3).*cos(q4).* ...
  sin(q2)+cos(q2).*sin(q4))+sin(q2).*sin(q3).*sin(q5))+((-1).*cos(q2).* ...
  cos(q4)+(-1).*cos(q3).*sin(q2).*sin(q4)).*sin(q6)).*sin(q7)).^2).^(-1)) ...
  .^(-1).*((-1/2).*(cos(q7).*(cos(q6).*(cos(q5).*((-1).*cos(q3).*cos(q4).* ...
  sin(q2)+cos(q2).*sin(q4))+sin(q2).*sin(q3).*sin(q5))+((-1).*cos(q2).* ...
  cos(q4)+(-1).*cos(q3).*sin(q2).*sin(q4)).*sin(q6))+(cos(q5).*sin(q2).* ...
  sin(q3)+(-1).*((-1).*cos(q3).*cos(q4).*sin(q2)+cos(q2).*sin(q4)).*sin( ...
  q5)).*sin(q7)).*(2.*((-1).*cos(q6).*sin(q2).*sin(q3).*sin(q4)+(cos(q4).* ...
  cos(q5).*sin(q2).*sin(q3)+cos(q3).*sin(q2).*sin(q5)).*sin(q6)).*((-1).* ...
  cos(q6).*((-1).*cos(q2).*cos(q4)+(-1).*cos(q3).*sin(q2).*sin(q4))+(cos( ...
  q5).*((-1).*cos(q3).*cos(q4).*sin(q2)+cos(q2).*sin(q4))+sin(q2).*sin(q3) ...
  .*sin(q5)).*sin(q6))+2.*(cos(q7).*(cos(q3).*cos(q5).*sin(q2)+(-1).*cos( ...
  q4).*sin(q2).*sin(q3).*sin(q5))+(-1).*(cos(q6).*(cos(q4).*cos(q5).*sin( ...
  q2).*sin(q3)+cos(q3).*sin(q2).*sin(q5))+sin(q2).*sin(q3).*sin(q4).*sin( ...
  q6)).*sin(q7)).*(cos(q7).*(cos(q5).*sin(q2).*sin(q3)+(-1).*((-1).*cos( ...
  q3).*cos(q4).*sin(q2)+cos(q2).*sin(q4)).*sin(q5))+(-1).*(cos(q6).*(cos( ...
  q5).*((-1).*cos(q3).*cos(q4).*sin(q2)+cos(q2).*sin(q4))+sin(q2).*sin(q3) ...
  .*sin(q5))+((-1).*cos(q2).*cos(q4)+(-1).*cos(q3).*sin(q2).*sin(q4)).* ...
  sin(q6)).*sin(q7))).*(((-1).*cos(q6).*((-1).*cos(q2).*cos(q4)+(-1).*cos( ...
  q3).*sin(q2).*sin(q4))+(cos(q5).*((-1).*cos(q3).*cos(q4).*sin(q2)+cos( ...
  q2).*sin(q4))+sin(q2).*sin(q3).*sin(q5)).*sin(q6)).^2+(cos(q7).*(cos(q5) ...
  .*sin(q2).*sin(q3)+(-1).*((-1).*cos(q3).*cos(q4).*sin(q2)+cos(q2).*sin( ...
  q4)).*sin(q5))+(-1).*(cos(q6).*(cos(q5).*((-1).*cos(q3).*cos(q4).*sin( ...
  q2)+cos(q2).*sin(q4))+sin(q2).*sin(q3).*sin(q5))+((-1).*cos(q2).*cos(q4) ...
  +(-1).*cos(q3).*sin(q2).*sin(q4)).*sin(q6)).*sin(q7)).^2).^(-3/2)+(cos( ...
  q7).*(cos(q6).*(cos(q4).*cos(q5).*sin(q2).*sin(q3)+cos(q3).*sin(q2).* ...
  sin(q5))+sin(q2).*sin(q3).*sin(q4).*sin(q6))+(cos(q3).*cos(q5).*sin(q2)+ ...
  (-1).*cos(q4).*sin(q2).*sin(q3).*sin(q5)).*sin(q7)).*(((-1).*cos(q6).*(( ...
  -1).*cos(q2).*cos(q4)+(-1).*cos(q3).*sin(q2).*sin(q4))+(cos(q5).*((-1).* ...
  cos(q3).*cos(q4).*sin(q2)+cos(q2).*sin(q4))+sin(q2).*sin(q3).*sin(q5)).* ...
  sin(q6)).^2+(cos(q7).*(cos(q5).*sin(q2).*sin(q3)+(-1).*((-1).*cos(q3).* ...
  cos(q4).*sin(q2)+cos(q2).*sin(q4)).*sin(q5))+(-1).*(cos(q6).*(cos(q5).*( ...
  (-1).*cos(q3).*cos(q4).*sin(q2)+cos(q2).*sin(q4))+sin(q2).*sin(q3).*sin( ...
  q5))+((-1).*cos(q2).*cos(q4)+(-1).*cos(q3).*sin(q2).*sin(q4)).*sin(q6)) ...
  .*sin(q7)).^2).^(-1/2));
  
  Jxe54 = (1+(cos(q7).*(cos(q6).*(cos(q5).*((-1).*cos(q3) ...
  .*cos(q4).*sin(q2)+cos(q2).*sin(q4))+sin(q2).*sin(q3).*sin(q5))+((-1).* ...
  cos(q2).*cos(q4)+(-1).*cos(q3).*sin(q2).*sin(q4)).*sin(q6))+(cos(q5).* ...
  sin(q2).*sin(q3)+(-1).*((-1).*cos(q3).*cos(q4).*sin(q2)+cos(q2).*sin(q4) ...
  ).*sin(q5)).*sin(q7)).^2.*(((-1).*cos(q6).*((-1).*cos(q2).*cos(q4)+(-1) ...
  .*cos(q3).*sin(q2).*sin(q4))+(cos(q5).*((-1).*cos(q3).*cos(q4).*sin(q2)+ ...
  cos(q2).*sin(q4))+sin(q2).*sin(q3).*sin(q5)).*sin(q6)).^2+(cos(q7).*( ...
  cos(q5).*sin(q2).*sin(q3)+(-1).*((-1).*cos(q3).*cos(q4).*sin(q2)+cos(q2) ...
  .*sin(q4)).*sin(q5))+(-1).*(cos(q6).*(cos(q5).*((-1).*cos(q3).*cos(q4).* ...
  sin(q2)+cos(q2).*sin(q4))+sin(q2).*sin(q3).*sin(q5))+((-1).*cos(q2).* ...
  cos(q4)+(-1).*cos(q3).*sin(q2).*sin(q4)).*sin(q6)).*sin(q7)).^2).^(-1)) ...
  .^(-1).*((-1/2).*(cos(q7).*(cos(q6).*(cos(q5).*((-1).*cos(q3).*cos(q4).* ...
  sin(q2)+cos(q2).*sin(q4))+sin(q2).*sin(q3).*sin(q5))+((-1).*cos(q2).* ...
  cos(q4)+(-1).*cos(q3).*sin(q2).*sin(q4)).*sin(q6))+(cos(q5).*sin(q2).* ...
  sin(q3)+(-1).*((-1).*cos(q3).*cos(q4).*sin(q2)+cos(q2).*sin(q4)).*sin( ...
  q5)).*sin(q7)).*(2.*((-1).*cos(q6).*((-1).*cos(q3).*cos(q4).*sin(q2)+ ...
  cos(q2).*sin(q4))+cos(q5).*(cos(q2).*cos(q4)+cos(q3).*sin(q2).*sin(q4)) ...
  .*sin(q6)).*((-1).*cos(q6).*((-1).*cos(q2).*cos(q4)+(-1).*cos(q3).*sin( ...
  q2).*sin(q4))+(cos(q5).*((-1).*cos(q3).*cos(q4).*sin(q2)+cos(q2).*sin( ...
  q4))+sin(q2).*sin(q3).*sin(q5)).*sin(q6))+2.*((-1).*cos(q7).*(cos(q2).* ...
  cos(q4)+cos(q3).*sin(q2).*sin(q4)).*sin(q5)+(-1).*(cos(q5).*cos(q6).*( ...
  cos(q2).*cos(q4)+cos(q3).*sin(q2).*sin(q4))+((-1).*cos(q3).*cos(q4).* ...
  sin(q2)+cos(q2).*sin(q4)).*sin(q6)).*sin(q7)).*(cos(q7).*(cos(q5).*sin( ...
  q2).*sin(q3)+(-1).*((-1).*cos(q3).*cos(q4).*sin(q2)+cos(q2).*sin(q4)).* ...
  sin(q5))+(-1).*(cos(q6).*(cos(q5).*((-1).*cos(q3).*cos(q4).*sin(q2)+cos( ...
  q2).*sin(q4))+sin(q2).*sin(q3).*sin(q5))+((-1).*cos(q2).*cos(q4)+(-1).* ...
  cos(q3).*sin(q2).*sin(q4)).*sin(q6)).*sin(q7))).*(((-1).*cos(q6).*((-1) ...
  .*cos(q2).*cos(q4)+(-1).*cos(q3).*sin(q2).*sin(q4))+(cos(q5).*((-1).* ...
  cos(q3).*cos(q4).*sin(q2)+cos(q2).*sin(q4))+sin(q2).*sin(q3).*sin(q5)).* ...
  sin(q6)).^2+(cos(q7).*(cos(q5).*sin(q2).*sin(q3)+(-1).*((-1).*cos(q3).* ...
  cos(q4).*sin(q2)+cos(q2).*sin(q4)).*sin(q5))+(-1).*(cos(q6).*(cos(q5).*( ...
  (-1).*cos(q3).*cos(q4).*sin(q2)+cos(q2).*sin(q4))+sin(q2).*sin(q3).*sin( ...
  q5))+((-1).*cos(q2).*cos(q4)+(-1).*cos(q3).*sin(q2).*sin(q4)).*sin(q6)) ...
  .*sin(q7)).^2).^(-3/2)+(cos(q7).*(cos(q5).*cos(q6).*(cos(q2).*cos(q4)+ ...
  cos(q3).*sin(q2).*sin(q4))+((-1).*cos(q3).*cos(q4).*sin(q2)+cos(q2).* ...
  sin(q4)).*sin(q6))+(-1).*(cos(q2).*cos(q4)+cos(q3).*sin(q2).*sin(q4)).* ...
  sin(q5).*sin(q7)).*(((-1).*cos(q6).*((-1).*cos(q2).*cos(q4)+(-1).*cos( ...
  q3).*sin(q2).*sin(q4))+(cos(q5).*((-1).*cos(q3).*cos(q4).*sin(q2)+cos( ...
  q2).*sin(q4))+sin(q2).*sin(q3).*sin(q5)).*sin(q6)).^2+(cos(q7).*(cos(q5) ...
  .*sin(q2).*sin(q3)+(-1).*((-1).*cos(q3).*cos(q4).*sin(q2)+cos(q2).*sin( ...
  q4)).*sin(q5))+(-1).*(cos(q6).*(cos(q5).*((-1).*cos(q3).*cos(q4).*sin( ...
  q2)+cos(q2).*sin(q4))+sin(q2).*sin(q3).*sin(q5))+((-1).*cos(q2).*cos(q4) ...
  +(-1).*cos(q3).*sin(q2).*sin(q4)).*sin(q6)).*sin(q7)).^2).^(-1/2));
  
  Jxe55 = (1+( ...
  cos(q7).*(cos(q6).*(cos(q5).*((-1).*cos(q3).*cos(q4).*sin(q2)+cos(q2).* ...
  sin(q4))+sin(q2).*sin(q3).*sin(q5))+((-1).*cos(q2).*cos(q4)+(-1).*cos( ...
  q3).*sin(q2).*sin(q4)).*sin(q6))+(cos(q5).*sin(q2).*sin(q3)+(-1).*((-1) ...
  .*cos(q3).*cos(q4).*sin(q2)+cos(q2).*sin(q4)).*sin(q5)).*sin(q7)).^2.*(( ...
  (-1).*cos(q6).*((-1).*cos(q2).*cos(q4)+(-1).*cos(q3).*sin(q2).*sin(q4))+ ...
  (cos(q5).*((-1).*cos(q3).*cos(q4).*sin(q2)+cos(q2).*sin(q4))+sin(q2).* ...
  sin(q3).*sin(q5)).*sin(q6)).^2+(cos(q7).*(cos(q5).*sin(q2).*sin(q3)+(-1) ...
  .*((-1).*cos(q3).*cos(q4).*sin(q2)+cos(q2).*sin(q4)).*sin(q5))+(-1).*( ...
  cos(q6).*(cos(q5).*((-1).*cos(q3).*cos(q4).*sin(q2)+cos(q2).*sin(q4))+ ...
  sin(q2).*sin(q3).*sin(q5))+((-1).*cos(q2).*cos(q4)+(-1).*cos(q3).*sin( ...
  q2).*sin(q4)).*sin(q6)).*sin(q7)).^2).^(-1)).^(-1).*((-1/2).*(cos(q7).*( ...
  cos(q6).*(cos(q5).*((-1).*cos(q3).*cos(q4).*sin(q2)+cos(q2).*sin(q4))+ ...
  sin(q2).*sin(q3).*sin(q5))+((-1).*cos(q2).*cos(q4)+(-1).*cos(q3).*sin( ...
  q2).*sin(q4)).*sin(q6))+(cos(q5).*sin(q2).*sin(q3)+(-1).*((-1).*cos(q3) ...
  .*cos(q4).*sin(q2)+cos(q2).*sin(q4)).*sin(q5)).*sin(q7)).*(2.*(cos(q5).* ...
  sin(q2).*sin(q3)+(-1).*((-1).*cos(q3).*cos(q4).*sin(q2)+cos(q2).*sin(q4) ...
  ).*sin(q5)).*sin(q6).*((-1).*cos(q6).*((-1).*cos(q2).*cos(q4)+(-1).*cos( ...
  q3).*sin(q2).*sin(q4))+(cos(q5).*((-1).*cos(q3).*cos(q4).*sin(q2)+cos( ...
  q2).*sin(q4))+sin(q2).*sin(q3).*sin(q5)).*sin(q6))+2.*(cos(q7).*((-1).* ...
  cos(q5).*((-1).*cos(q3).*cos(q4).*sin(q2)+cos(q2).*sin(q4))+(-1).*sin( ...
  q2).*sin(q3).*sin(q5))+(-1).*cos(q6).*(cos(q5).*sin(q2).*sin(q3)+(-1).*( ...
  (-1).*cos(q3).*cos(q4).*sin(q2)+cos(q2).*sin(q4)).*sin(q5)).*sin(q7)).*( ...
  cos(q7).*(cos(q5).*sin(q2).*sin(q3)+(-1).*((-1).*cos(q3).*cos(q4).*sin( ...
  q2)+cos(q2).*sin(q4)).*sin(q5))+(-1).*(cos(q6).*(cos(q5).*((-1).*cos(q3) ...
  .*cos(q4).*sin(q2)+cos(q2).*sin(q4))+sin(q2).*sin(q3).*sin(q5))+((-1).* ...
  cos(q2).*cos(q4)+(-1).*cos(q3).*sin(q2).*sin(q4)).*sin(q6)).*sin(q7))).* ...
  (((-1).*cos(q6).*((-1).*cos(q2).*cos(q4)+(-1).*cos(q3).*sin(q2).*sin(q4) ...
  )+(cos(q5).*((-1).*cos(q3).*cos(q4).*sin(q2)+cos(q2).*sin(q4))+sin(q2).* ...
  sin(q3).*sin(q5)).*sin(q6)).^2+(cos(q7).*(cos(q5).*sin(q2).*sin(q3)+(-1) ...
  .*((-1).*cos(q3).*cos(q4).*sin(q2)+cos(q2).*sin(q4)).*sin(q5))+(-1).*( ...
  cos(q6).*(cos(q5).*((-1).*cos(q3).*cos(q4).*sin(q2)+cos(q2).*sin(q4))+ ...
  sin(q2).*sin(q3).*sin(q5))+((-1).*cos(q2).*cos(q4)+(-1).*cos(q3).*sin( ...
  q2).*sin(q4)).*sin(q6)).*sin(q7)).^2).^(-3/2)+(cos(q6).*cos(q7).*(cos( ...
  q5).*sin(q2).*sin(q3)+(-1).*((-1).*cos(q3).*cos(q4).*sin(q2)+cos(q2).* ...
  sin(q4)).*sin(q5))+((-1).*cos(q5).*((-1).*cos(q3).*cos(q4).*sin(q2)+cos( ...
  q2).*sin(q4))+(-1).*sin(q2).*sin(q3).*sin(q5)).*sin(q7)).*(((-1).*cos( ...
  q6).*((-1).*cos(q2).*cos(q4)+(-1).*cos(q3).*sin(q2).*sin(q4))+(cos(q5).* ...
  ((-1).*cos(q3).*cos(q4).*sin(q2)+cos(q2).*sin(q4))+sin(q2).*sin(q3).* ...
  sin(q5)).*sin(q6)).^2+(cos(q7).*(cos(q5).*sin(q2).*sin(q3)+(-1).*((-1).* ...
  cos(q3).*cos(q4).*sin(q2)+cos(q2).*sin(q4)).*sin(q5))+(-1).*(cos(q6).*( ...
  cos(q5).*((-1).*cos(q3).*cos(q4).*sin(q2)+cos(q2).*sin(q4))+sin(q2).* ...
  sin(q3).*sin(q5))+((-1).*cos(q2).*cos(q4)+(-1).*cos(q3).*sin(q2).*sin( ...
  q4)).*sin(q6)).*sin(q7)).^2).^(-1/2));
  
  Jxe56 = (1+(cos(q7).*(cos(q6).*(cos(q5).*( ...
  (-1).*cos(q3).*cos(q4).*sin(q2)+cos(q2).*sin(q4))+sin(q2).*sin(q3).*sin( ...
  q5))+((-1).*cos(q2).*cos(q4)+(-1).*cos(q3).*sin(q2).*sin(q4)).*sin(q6))+ ...
  (cos(q5).*sin(q2).*sin(q3)+(-1).*((-1).*cos(q3).*cos(q4).*sin(q2)+cos( ...
  q2).*sin(q4)).*sin(q5)).*sin(q7)).^2.*(((-1).*cos(q6).*((-1).*cos(q2).* ...
  cos(q4)+(-1).*cos(q3).*sin(q2).*sin(q4))+(cos(q5).*((-1).*cos(q3).*cos( ...
  q4).*sin(q2)+cos(q2).*sin(q4))+sin(q2).*sin(q3).*sin(q5)).*sin(q6)).^2+( ...
  cos(q7).*(cos(q5).*sin(q2).*sin(q3)+(-1).*((-1).*cos(q3).*cos(q4).*sin( ...
  q2)+cos(q2).*sin(q4)).*sin(q5))+(-1).*(cos(q6).*(cos(q5).*((-1).*cos(q3) ...
  .*cos(q4).*sin(q2)+cos(q2).*sin(q4))+sin(q2).*sin(q3).*sin(q5))+((-1).* ...
  cos(q2).*cos(q4)+(-1).*cos(q3).*sin(q2).*sin(q4)).*sin(q6)).*sin(q7)) ...
  .^2).^(-1)).^(-1).*((-1/2).*(cos(q7).*(cos(q6).*(cos(q5).*((-1).*cos(q3) ...
  .*cos(q4).*sin(q2)+cos(q2).*sin(q4))+sin(q2).*sin(q3).*sin(q5))+((-1).* ...
  cos(q2).*cos(q4)+(-1).*cos(q3).*sin(q2).*sin(q4)).*sin(q6))+(cos(q5).* ...
  sin(q2).*sin(q3)+(-1).*((-1).*cos(q3).*cos(q4).*sin(q2)+cos(q2).*sin(q4) ...
  ).*sin(q5)).*sin(q7)).*(2.*(cos(q6).*(cos(q5).*((-1).*cos(q3).*cos(q4).* ...
  sin(q2)+cos(q2).*sin(q4))+sin(q2).*sin(q3).*sin(q5))+((-1).*cos(q2).* ...
  cos(q4)+(-1).*cos(q3).*sin(q2).*sin(q4)).*sin(q6)).*((-1).*cos(q6).*(( ...
  -1).*cos(q2).*cos(q4)+(-1).*cos(q3).*sin(q2).*sin(q4))+(cos(q5).*((-1).* ...
  cos(q3).*cos(q4).*sin(q2)+cos(q2).*sin(q4))+sin(q2).*sin(q3).*sin(q5)).* ...
  sin(q6))+(-2).*(cos(q6).*((-1).*cos(q2).*cos(q4)+(-1).*cos(q3).*sin(q2) ...
  .*sin(q4))+(-1).*(cos(q5).*((-1).*cos(q3).*cos(q4).*sin(q2)+cos(q2).* ...
  sin(q4))+sin(q2).*sin(q3).*sin(q5)).*sin(q6)).*sin(q7).*(cos(q7).*(cos( ...
  q5).*sin(q2).*sin(q3)+(-1).*((-1).*cos(q3).*cos(q4).*sin(q2)+cos(q2).* ...
  sin(q4)).*sin(q5))+(-1).*(cos(q6).*(cos(q5).*((-1).*cos(q3).*cos(q4).* ...
  sin(q2)+cos(q2).*sin(q4))+sin(q2).*sin(q3).*sin(q5))+((-1).*cos(q2).* ...
  cos(q4)+(-1).*cos(q3).*sin(q2).*sin(q4)).*sin(q6)).*sin(q7))).*(((-1).* ...
  cos(q6).*((-1).*cos(q2).*cos(q4)+(-1).*cos(q3).*sin(q2).*sin(q4))+(cos( ...
  q5).*((-1).*cos(q3).*cos(q4).*sin(q2)+cos(q2).*sin(q4))+sin(q2).*sin(q3) ...
  .*sin(q5)).*sin(q6)).^2+(cos(q7).*(cos(q5).*sin(q2).*sin(q3)+(-1).*((-1) ...
  .*cos(q3).*cos(q4).*sin(q2)+cos(q2).*sin(q4)).*sin(q5))+(-1).*(cos(q6).* ...
  (cos(q5).*((-1).*cos(q3).*cos(q4).*sin(q2)+cos(q2).*sin(q4))+sin(q2).* ...
  sin(q3).*sin(q5))+((-1).*cos(q2).*cos(q4)+(-1).*cos(q3).*sin(q2).*sin( ...
  q4)).*sin(q6)).*sin(q7)).^2).^(-3/2)+cos(q7).*(cos(q6).*((-1).*cos(q2).* ...
  cos(q4)+(-1).*cos(q3).*sin(q2).*sin(q4))+(-1).*(cos(q5).*((-1).*cos(q3) ...
  .*cos(q4).*sin(q2)+cos(q2).*sin(q4))+sin(q2).*sin(q3).*sin(q5)).*sin(q6) ...
  ).*(((-1).*cos(q6).*((-1).*cos(q2).*cos(q4)+(-1).*cos(q3).*sin(q2).*sin( ...
  q4))+(cos(q5).*((-1).*cos(q3).*cos(q4).*sin(q2)+cos(q2).*sin(q4))+sin( ...
  q2).*sin(q3).*sin(q5)).*sin(q6)).^2+(cos(q7).*(cos(q5).*sin(q2).*sin(q3) ...
  +(-1).*((-1).*cos(q3).*cos(q4).*sin(q2)+cos(q2).*sin(q4)).*sin(q5))+(-1) ...
  .*(cos(q6).*(cos(q5).*((-1).*cos(q3).*cos(q4).*sin(q2)+cos(q2).*sin(q4)) ...
  +sin(q2).*sin(q3).*sin(q5))+((-1).*cos(q2).*cos(q4)+(-1).*cos(q3).*sin( ...
  q2).*sin(q4)).*sin(q6)).*sin(q7)).^2).^(-1/2));
  
  Jxe57 = (1+(cos(q7).*(cos(q6).*( ...
  cos(q5).*((-1).*cos(q3).*cos(q4).*sin(q2)+cos(q2).*sin(q4))+sin(q2).* ...
  sin(q3).*sin(q5))+((-1).*cos(q2).*cos(q4)+(-1).*cos(q3).*sin(q2).*sin( ...
  q4)).*sin(q6))+(cos(q5).*sin(q2).*sin(q3)+(-1).*((-1).*cos(q3).*cos(q4) ...
  .*sin(q2)+cos(q2).*sin(q4)).*sin(q5)).*sin(q7)).^2.*(((-1).*cos(q6).*(( ...
  -1).*cos(q2).*cos(q4)+(-1).*cos(q3).*sin(q2).*sin(q4))+(cos(q5).*((-1).* ...
  cos(q3).*cos(q4).*sin(q2)+cos(q2).*sin(q4))+sin(q2).*sin(q3).*sin(q5)).* ...
  sin(q6)).^2+(cos(q7).*(cos(q5).*sin(q2).*sin(q3)+(-1).*((-1).*cos(q3).* ...
  cos(q4).*sin(q2)+cos(q2).*sin(q4)).*sin(q5))+(-1).*(cos(q6).*(cos(q5).*( ...
  (-1).*cos(q3).*cos(q4).*sin(q2)+cos(q2).*sin(q4))+sin(q2).*sin(q3).*sin( ...
  q5))+((-1).*cos(q2).*cos(q4)+(-1).*cos(q3).*sin(q2).*sin(q4)).*sin(q6)) ...
  .*sin(q7)).^2).^(-1)).^(-1).*((-1).*((-1).*cos(q7).*(cos(q6).*(cos(q5).* ...
  ((-1).*cos(q3).*cos(q4).*sin(q2)+cos(q2).*sin(q4))+sin(q2).*sin(q3).* ...
  sin(q5))+((-1).*cos(q2).*cos(q4)+(-1).*cos(q3).*sin(q2).*sin(q4)).*sin( ...
  q6))+(-1).*(cos(q5).*sin(q2).*sin(q3)+(-1).*((-1).*cos(q3).*cos(q4).* ...
  sin(q2)+cos(q2).*sin(q4)).*sin(q5)).*sin(q7)).*(cos(q7).*(cos(q6).*(cos( ...
  q5).*((-1).*cos(q3).*cos(q4).*sin(q2)+cos(q2).*sin(q4))+sin(q2).*sin(q3) ...
  .*sin(q5))+((-1).*cos(q2).*cos(q4)+(-1).*cos(q3).*sin(q2).*sin(q4)).* ...
  sin(q6))+(cos(q5).*sin(q2).*sin(q3)+(-1).*((-1).*cos(q3).*cos(q4).*sin( ...
  q2)+cos(q2).*sin(q4)).*sin(q5)).*sin(q7)).*(cos(q7).*(cos(q5).*sin(q2).* ...
  sin(q3)+(-1).*((-1).*cos(q3).*cos(q4).*sin(q2)+cos(q2).*sin(q4)).*sin( ...
  q5))+(-1).*(cos(q6).*(cos(q5).*((-1).*cos(q3).*cos(q4).*sin(q2)+cos(q2) ...
  .*sin(q4))+sin(q2).*sin(q3).*sin(q5))+((-1).*cos(q2).*cos(q4)+(-1).*cos( ...
  q3).*sin(q2).*sin(q4)).*sin(q6)).*sin(q7)).*(((-1).*cos(q6).*((-1).*cos( ...
  q2).*cos(q4)+(-1).*cos(q3).*sin(q2).*sin(q4))+(cos(q5).*((-1).*cos(q3).* ...
  cos(q4).*sin(q2)+cos(q2).*sin(q4))+sin(q2).*sin(q3).*sin(q5)).*sin(q6)) ...
  .^2+(cos(q7).*(cos(q5).*sin(q2).*sin(q3)+(-1).*((-1).*cos(q3).*cos(q4).* ...
  sin(q2)+cos(q2).*sin(q4)).*sin(q5))+(-1).*(cos(q6).*(cos(q5).*((-1).* ...
  cos(q3).*cos(q4).*sin(q2)+cos(q2).*sin(q4))+sin(q2).*sin(q3).*sin(q5))+( ...
  (-1).*cos(q2).*cos(q4)+(-1).*cos(q3).*sin(q2).*sin(q4)).*sin(q6)).*sin( ...
  q7)).^2).^(-3/2)+(cos(q7).*(cos(q5).*sin(q2).*sin(q3)+(-1).*((-1).*cos( ...
  q3).*cos(q4).*sin(q2)+cos(q2).*sin(q4)).*sin(q5))+(-1).*(cos(q6).*(cos( ...
  q5).*((-1).*cos(q3).*cos(q4).*sin(q2)+cos(q2).*sin(q4))+sin(q2).*sin(q3) ...
  .*sin(q5))+((-1).*cos(q2).*cos(q4)+(-1).*cos(q3).*sin(q2).*sin(q4)).* ...
  sin(q6)).*sin(q7)).*(((-1).*cos(q6).*((-1).*cos(q2).*cos(q4)+(-1).*cos( ...
  q3).*sin(q2).*sin(q4))+(cos(q5).*((-1).*cos(q3).*cos(q4).*sin(q2)+cos( ...
  q2).*sin(q4))+sin(q2).*sin(q3).*sin(q5)).*sin(q6)).^2+(cos(q7).*(cos(q5) ...
  .*sin(q2).*sin(q3)+(-1).*((-1).*cos(q3).*cos(q4).*sin(q2)+cos(q2).*sin( ...
  q4)).*sin(q5))+(-1).*(cos(q6).*(cos(q5).*((-1).*cos(q3).*cos(q4).*sin( ...
  q2)+cos(q2).*sin(q4))+sin(q2).*sin(q3).*sin(q5))+((-1).*cos(q2).*cos(q4) ...
  +(-1).*cos(q3).*sin(q2).*sin(q4)).*sin(q6)).*sin(q7)).^2).^(-1/2));
  
  
  Jxe61 = 0;
  
  Jxe62 = (( ...
  -1).*cos(q6).*((-1).*cos(q2).*cos(q4)+(-1).*cos(q3).*sin(q2).*sin(q4))+( ...
  cos(q5).*((-1).*cos(q3).*cos(q4).*sin(q2)+cos(q2).*sin(q4))+sin(q2).* ...
  sin(q3).*sin(q5)).*sin(q6)).^(-1).*(cos(q7).*(cos(q2).*cos(q5).*sin(q3)+ ...
  (-1).*((-1).*cos(q2).*cos(q3).*cos(q4)+(-1).*sin(q2).*sin(q4)).*sin(q5)) ...
  +(-1).*(cos(q6).*(cos(q5).*((-1).*cos(q2).*cos(q3).*cos(q4)+(-1).*sin( ...
  q2).*sin(q4))+cos(q2).*sin(q3).*sin(q5))+(cos(q4).*sin(q2)+(-1).*cos(q2) ...
  .*cos(q3).*sin(q4)).*sin(q6)).*sin(q7))+(-1).*((-1).*cos(q6).*(cos(q4).* ...
  sin(q2)+(-1).*cos(q2).*cos(q3).*sin(q4))+(cos(q5).*((-1).*cos(q2).*cos( ...
  q3).*cos(q4)+(-1).*sin(q2).*sin(q4))+cos(q2).*sin(q3).*sin(q5)).*sin(q6) ...
  ).*((-1).*cos(q6).*((-1).*cos(q2).*cos(q4)+(-1).*cos(q3).*sin(q2).*sin( ...
  q4))+(cos(q5).*((-1).*cos(q3).*cos(q4).*sin(q2)+cos(q2).*sin(q4))+sin( ...
  q2).*sin(q3).*sin(q5)).*sin(q6)).^(-2).*(cos(q7).*(cos(q5).*sin(q2).* ...
  sin(q3)+(-1).*((-1).*cos(q3).*cos(q4).*sin(q2)+cos(q2).*sin(q4)).*sin( ...
  q5))+(-1).*(cos(q6).*(cos(q5).*((-1).*cos(q3).*cos(q4).*sin(q2)+cos(q2) ...
  .*sin(q4))+sin(q2).*sin(q3).*sin(q5))+((-1).*cos(q2).*cos(q4)+(-1).*cos( ...
  q3).*sin(q2).*sin(q4)).*sin(q6)).*sin(q7));
  
  Jxe63 = ((-1).*cos(q6).*((-1).*cos( ...
  q2).*cos(q4)+(-1).*cos(q3).*sin(q2).*sin(q4))+(cos(q5).*((-1).*cos(q3).* ...
  cos(q4).*sin(q2)+cos(q2).*sin(q4))+sin(q2).*sin(q3).*sin(q5)).*sin(q6)) ...
  .^(-1).*(cos(q7).*(cos(q3).*cos(q5).*sin(q2)+(-1).*cos(q4).*sin(q2).* ...
  sin(q3).*sin(q5))+(-1).*(cos(q6).*(cos(q4).*cos(q5).*sin(q2).*sin(q3)+ ...
  cos(q3).*sin(q2).*sin(q5))+sin(q2).*sin(q3).*sin(q4).*sin(q6)).*sin(q7)) ...
  +(-1).*((-1).*cos(q6).*sin(q2).*sin(q3).*sin(q4)+(cos(q4).*cos(q5).*sin( ...
  q2).*sin(q3)+cos(q3).*sin(q2).*sin(q5)).*sin(q6)).*((-1).*cos(q6).*((-1) ...
  .*cos(q2).*cos(q4)+(-1).*cos(q3).*sin(q2).*sin(q4))+(cos(q5).*((-1).* ...
  cos(q3).*cos(q4).*sin(q2)+cos(q2).*sin(q4))+sin(q2).*sin(q3).*sin(q5)).* ...
  sin(q6)).^(-2).*(cos(q7).*(cos(q5).*sin(q2).*sin(q3)+(-1).*((-1).*cos( ...
  q3).*cos(q4).*sin(q2)+cos(q2).*sin(q4)).*sin(q5))+(-1).*(cos(q6).*(cos( ...
  q5).*((-1).*cos(q3).*cos(q4).*sin(q2)+cos(q2).*sin(q4))+sin(q2).*sin(q3) ...
  .*sin(q5))+((-1).*cos(q2).*cos(q4)+(-1).*cos(q3).*sin(q2).*sin(q4)).* ...
  sin(q6)).*sin(q7));
  
  Jxe64 = ((-1).*cos(q6).*((-1).*cos(q2).*cos(q4)+(-1).*cos(q3) ...
  .*sin(q2).*sin(q4))+(cos(q5).*((-1).*cos(q3).*cos(q4).*sin(q2)+cos(q2).* ...
  sin(q4))+sin(q2).*sin(q3).*sin(q5)).*sin(q6)).^(-1).*((-1).*cos(q7).*( ...
  cos(q2).*cos(q4)+cos(q3).*sin(q2).*sin(q4)).*sin(q5)+(-1).*(cos(q5).* ...
  cos(q6).*(cos(q2).*cos(q4)+cos(q3).*sin(q2).*sin(q4))+((-1).*cos(q3).* ...
  cos(q4).*sin(q2)+cos(q2).*sin(q4)).*sin(q6)).*sin(q7))+(-1).*((-1).*cos( ...
  q6).*((-1).*cos(q3).*cos(q4).*sin(q2)+cos(q2).*sin(q4))+cos(q5).*(cos( ...
  q2).*cos(q4)+cos(q3).*sin(q2).*sin(q4)).*sin(q6)).*((-1).*cos(q6).*((-1) ...
  .*cos(q2).*cos(q4)+(-1).*cos(q3).*sin(q2).*sin(q4))+(cos(q5).*((-1).* ...
  cos(q3).*cos(q4).*sin(q2)+cos(q2).*sin(q4))+sin(q2).*sin(q3).*sin(q5)).* ...
  sin(q6)).^(-2).*(cos(q7).*(cos(q5).*sin(q2).*sin(q3)+(-1).*((-1).*cos( ...
  q3).*cos(q4).*sin(q2)+cos(q2).*sin(q4)).*sin(q5))+(-1).*(cos(q6).*(cos( ...
  q5).*((-1).*cos(q3).*cos(q4).*sin(q2)+cos(q2).*sin(q4))+sin(q2).*sin(q3) ...
  .*sin(q5))+((-1).*cos(q2).*cos(q4)+(-1).*cos(q3).*sin(q2).*sin(q4)).* ...
  sin(q6)).*sin(q7));
  
  Jxe65 = ((-1).*cos(q6).*((-1).*cos(q2).*cos(q4)+(-1).*cos(q3) ...
  .*sin(q2).*sin(q4))+(cos(q5).*((-1).*cos(q3).*cos(q4).*sin(q2)+cos(q2).* ...
  sin(q4))+sin(q2).*sin(q3).*sin(q5)).*sin(q6)).^(-1).*(cos(q7).*((-1).* ...
  cos(q5).*((-1).*cos(q3).*cos(q4).*sin(q2)+cos(q2).*sin(q4))+(-1).*sin( ...
  q2).*sin(q3).*sin(q5))+(-1).*cos(q6).*(cos(q5).*sin(q2).*sin(q3)+(-1).*( ...
  (-1).*cos(q3).*cos(q4).*sin(q2)+cos(q2).*sin(q4)).*sin(q5)).*sin(q7))+( ...
  -1).*(cos(q5).*sin(q2).*sin(q3)+(-1).*((-1).*cos(q3).*cos(q4).*sin(q2)+ ...
  cos(q2).*sin(q4)).*sin(q5)).*sin(q6).*((-1).*cos(q6).*((-1).*cos(q2).* ...
  cos(q4)+(-1).*cos(q3).*sin(q2).*sin(q4))+(cos(q5).*((-1).*cos(q3).*cos( ...
  q4).*sin(q2)+cos(q2).*sin(q4))+sin(q2).*sin(q3).*sin(q5)).*sin(q6)).^( ...
  -2).*(cos(q7).*(cos(q5).*sin(q2).*sin(q3)+(-1).*((-1).*cos(q3).*cos(q4) ...
  .*sin(q2)+cos(q2).*sin(q4)).*sin(q5))+(-1).*(cos(q6).*(cos(q5).*((-1).* ...
  cos(q3).*cos(q4).*sin(q2)+cos(q2).*sin(q4))+sin(q2).*sin(q3).*sin(q5))+( ...
  (-1).*cos(q2).*cos(q4)+(-1).*cos(q3).*sin(q2).*sin(q4)).*sin(q6)).*sin( ...
  q7));
  
  Jxe66 = (-1).*(cos(q6).*((-1).*cos(q2).*cos(q4)+(-1).*cos(q3).*sin(q2).* ...
  sin(q4))+(-1).*(cos(q5).*((-1).*cos(q3).*cos(q4).*sin(q2)+cos(q2).*sin( ...
  q4))+sin(q2).*sin(q3).*sin(q5)).*sin(q6)).*((-1).*cos(q6).*((-1).*cos( ...
  q2).*cos(q4)+(-1).*cos(q3).*sin(q2).*sin(q4))+(cos(q5).*((-1).*cos(q3).* ...
  cos(q4).*sin(q2)+cos(q2).*sin(q4))+sin(q2).*sin(q3).*sin(q5)).*sin(q6)) ...
  .^(-1).*sin(q7)+(-1).*(cos(q6).*(cos(q5).*((-1).*cos(q3).*cos(q4).*sin( ...
  q2)+cos(q2).*sin(q4))+sin(q2).*sin(q3).*sin(q5))+((-1).*cos(q2).*cos(q4) ...
  +(-1).*cos(q3).*sin(q2).*sin(q4)).*sin(q6)).*((-1).*cos(q6).*((-1).*cos( ...
  q2).*cos(q4)+(-1).*cos(q3).*sin(q2).*sin(q4))+(cos(q5).*((-1).*cos(q3).* ...
  cos(q4).*sin(q2)+cos(q2).*sin(q4))+sin(q2).*sin(q3).*sin(q5)).*sin(q6)) ...
  .^(-2).*(cos(q7).*(cos(q5).*sin(q2).*sin(q3)+(-1).*((-1).*cos(q3).*cos( ...
  q4).*sin(q2)+cos(q2).*sin(q4)).*sin(q5))+(-1).*(cos(q6).*(cos(q5).*((-1) ...
  .*cos(q3).*cos(q4).*sin(q2)+cos(q2).*sin(q4))+sin(q2).*sin(q3).*sin(q5)) ...
  +((-1).*cos(q2).*cos(q4)+(-1).*cos(q3).*sin(q2).*sin(q4)).*sin(q6)).* ...
  sin(q7));
  
  Jxe67 = ((-1).*cos(q6).*((-1).*cos(q2).*cos(q4)+(-1).*cos(q3).*sin(q2) ...
  .*sin(q4))+(cos(q5).*((-1).*cos(q3).*cos(q4).*sin(q2)+cos(q2).*sin(q4))+ ...
  sin(q2).*sin(q3).*sin(q5)).*sin(q6)).^(-1).*((-1).*cos(q7).*(cos(q6).*( ...
  cos(q5).*((-1).*cos(q3).*cos(q4).*sin(q2)+cos(q2).*sin(q4))+sin(q2).* ...
  sin(q3).*sin(q5))+((-1).*cos(q2).*cos(q4)+(-1).*cos(q3).*sin(q2).*sin( ...
  q4)).*sin(q6))+(-1).*(cos(q5).*sin(q2).*sin(q3)+(-1).*((-1).*cos(q3).* ...
  cos(q4).*sin(q2)+cos(q2).*sin(q4)).*sin(q5)).*sin(q7));




Jxe = [Jxe11, Jxe12, Jxe13, Jxe14, Jxe15, Jxe16, Jxe17;
       Jxe21, Jxe22, Jxe23, Jxe24, Jxe25, Jxe26, Jxe27;
       Jxe31, Jxe32, Jxe33, Jxe34, Jxe35, Jxe36, Jxe37;
       Jxe41, Jxe42, Jxe43, Jxe44, Jxe45, Jxe46, Jxe47;
       Jxe51, Jxe52, Jxe53, Jxe54, Jxe55, Jxe56, Jxe57;
       Jxe61, Jxe62, Jxe63, Jxe64, Jxe65, Jxe66, Jxe67];



   
   
   
   

Jxe211 = (-1).*Kuka_LBR_param_.dblLink23Len.*cos(q1).*sin(q2)+Kuka_LBR_param_.dblLink45Len.*((-1).*cos(q1).*cos(q4).*sin(q2)+(cos( ...
  q1).*cos(q2).*cos(q3)+(-1).*sin(q1).*sin(q3)).*sin(q4))+Kuka_LBR_param_.dblLink67Len.*((-1).*cos( ...
  q6).*(cos(q1).*cos(q4).*sin(q2)+((-1).*cos(q1).*cos(q2).*cos(q3)+sin(q1) ...
  .*sin(q3)).*sin(q4))+(cos(q5).*(cos(q4).*((-1).*cos(q1).*cos(q2).*cos( ...
  q3)+sin(q1).*sin(q3))+(-1).*cos(q1).*sin(q2).*sin(q4))+(cos(q3).*sin(q1) ...
  +cos(q1).*cos(q2).*sin(q3)).*sin(q5)).*sin(q6));

Jxe212 = (-1).*Kuka_LBR_param_.dblLink23Len.*cos(q1).*sin( ...
  q2)+Kuka_LBR_param_.dblLink45Len.*((-1).*cos(q1).*cos(q4).*sin(q2)+cos(q1).*cos(q2).*cos(q3).* ...
  sin(q4))+Kuka_LBR_param_.dblLink67Len.*((-1).*cos(q6).*(cos(q1).*cos(q4).*sin(q2)+(-1).*cos(q1).* ...
  cos(q2).*cos(q3).*sin(q4))+(cos(q5).*((-1).*cos(q1).*cos(q2).*cos(q3).* ...
  cos(q4)+(-1).*cos(q1).*sin(q2).*sin(q4))+cos(q1).*cos(q2).*sin(q3).*sin( ...
  q5)).*sin(q6));

Jxe213 = Kuka_LBR_param_.dblLink45Len.*(cos(q1).*cos(q2).*cos(q3)+(-1).*sin(q1).*sin(q3)).* ...
  sin(q4)+Kuka_LBR_param_.dblLink67Len.*((-1).*cos(q6).*((-1).*cos(q1).*cos(q2).*cos(q3)+sin(q1).* ...
  sin(q3)).*sin(q4)+(cos(q4).*cos(q5).*((-1).*cos(q1).*cos(q2).*cos(q3)+ ...
  sin(q1).*sin(q3))+(cos(q3).*sin(q1)+cos(q1).*cos(q2).*sin(q3)).*sin(q5)) ...
  .*sin(q6));

Jxe214 = Kuka_LBR_param_.dblLink45Len.*((-1).*cos(q1).*cos(q4).*sin(q2)+(cos(q1).*cos(q2).*cos( ...
  q3)+(-1).*sin(q1).*sin(q3)).*sin(q4))+Kuka_LBR_param_.dblLink67Len.*((-1).*cos(q6).*(cos(q1).* ...
  cos(q4).*sin(q2)+(-1).*(cos(q1).*cos(q2).*cos(q3)+(-1).*sin(q1).*sin(q3) ...
  ).*sin(q4))+cos(q5).*((-1).*cos(q4).*(cos(q1).*cos(q2).*cos(q3)+(-1).* ...
  sin(q1).*sin(q3))+(-1).*cos(q1).*sin(q2).*sin(q4)).*sin(q6));

Jxe215 = Kuka_LBR_param_.dblLink67Len.*((-1) ...
  .*cos(q5).*(cos(q4).*(cos(q1).*cos(q2).*cos(q3)+(-1).*sin(q1).*sin(q3))+ ...
  cos(q1).*sin(q2).*sin(q4))+(-1).*((-1).*cos(q3).*sin(q1)+(-1).*cos(q1).* ...
  cos(q2).*sin(q3)).*sin(q5)).*sin(q6);

Jxe216 = Kuka_LBR_param_.dblLink67Len.*(cos(q6).*((-1).*cos(q1).*cos( ...
  q4).*sin(q2)+(cos(q1).*cos(q2).*cos(q3)+(-1).*sin(q1).*sin(q3)).*sin(q4) ...
  )+(-1).*(cos(q5).*(cos(q4).*(cos(q1).*cos(q2).*cos(q3)+(-1).*sin(q1).* ...
  sin(q3))+cos(q1).*sin(q2).*sin(q4))+((-1).*cos(q3).*sin(q1)+(-1).*cos( ...
  q1).*cos(q2).*sin(q3)).*sin(q5)).*sin(q6));

Jxe217 = 0;

Jxe221 = (-1).*Kuka_LBR_param_.dblLink23Len.*sin(q1).*sin(q2) ...
  +Kuka_LBR_param_.dblLink45Len.*((-1).*cos(q4).*sin(q1).*sin(q2)+(cos(q2).*cos(q3).*sin(q1)+cos( ...
  q1).*sin(q3)).*sin(q4))+Kuka_LBR_param_.dblLink67Len.*((-1).*cos(q6).*(cos(q4).*sin(q1).*sin(q2)+ ...
  ((-1).*cos(q2).*cos(q3).*sin(q1)+(-1).*cos(q1).*sin(q3)).*sin(q4))+(cos( ...
  q5).*(cos(q4).*((-1).*cos(q2).*cos(q3).*sin(q1)+(-1).*cos(q1).*sin(q3))+ ...
  (-1).*sin(q1).*sin(q2).*sin(q4))+((-1).*cos(q1).*cos(q3)+cos(q2).*sin( ...
  q1).*sin(q3)).*sin(q5)).*sin(q6));

Jxe222 = (-1).*Kuka_LBR_param_.dblLink23Len.*sin(q1).*sin(q2)+Kuka_LBR_param_.dblLink45Len.*((-1) ...
  .*cos(q4).*sin(q1).*sin(q2)+cos(q2).*cos(q3).*sin(q1).*sin(q4))+Kuka_LBR_param_.dblLink67Len.*(( ...
  -1).*cos(q6).*(cos(q4).*sin(q1).*sin(q2)+(-1).*cos(q2).*cos(q3).*sin(q1) ...
  .*sin(q4))+(cos(q5).*((-1).*cos(q2).*cos(q3).*cos(q4).*sin(q1)+(-1).* ...
  sin(q1).*sin(q2).*sin(q4))+cos(q2).*sin(q1).*sin(q3).*sin(q5)).*sin(q6)) ...
  ;

Jxe223 = Kuka_LBR_param_.dblLink45Len.*(cos(q2).*cos(q3).*sin(q1)+cos(q1).*sin(q3)).*sin(q4)+Kuka_LBR_param_.dblLink67Len.*((-1).* ...
  cos(q6).*((-1).*cos(q2).*cos(q3).*sin(q1)+(-1).*cos(q1).*sin(q3)).*sin( ...
  q4)+(cos(q4).*cos(q5).*((-1).*cos(q2).*cos(q3).*sin(q1)+(-1).*cos(q1).* ...
  sin(q3))+((-1).*cos(q1).*cos(q3)+cos(q2).*sin(q1).*sin(q3)).*sin(q5)).* ...
  sin(q6));

Jxe224 = Kuka_LBR_param_.dblLink45Len.*((-1).*cos(q4).*sin(q1).*sin(q2)+(cos(q2).*cos(q3).*sin( ...
  q1)+cos(q1).*sin(q3)).*sin(q4))+Kuka_LBR_param_.dblLink67Len.*((-1).*cos(q6).*(cos(q4).*sin(q1).* ...
  sin(q2)+(-1).*(cos(q2).*cos(q3).*sin(q1)+cos(q1).*sin(q3)).*sin(q4))+ ...
  cos(q5).*((-1).*cos(q4).*(cos(q2).*cos(q3).*sin(q1)+cos(q1).*sin(q3))+( ...
  -1).*sin(q1).*sin(q2).*sin(q4)).*sin(q6));

Jxe225 = Kuka_LBR_param_.dblLink67Len.*((-1).*cos(q5).*(cos(q4) ...
  .*(cos(q2).*cos(q3).*sin(q1)+cos(q1).*sin(q3))+sin(q1).*sin(q2).*sin(q4) ...
  )+(-1).*(cos(q1).*cos(q3)+(-1).*cos(q2).*sin(q1).*sin(q3)).*sin(q5)).* ...
  sin(q6);

Jxe226 = Kuka_LBR_param_.dblLink67Len.*(cos(q6).*((-1).*cos(q4).*sin(q1).*sin(q2)+(cos(q2).*cos( ...
  q3).*sin(q1)+cos(q1).*sin(q3)).*sin(q4))+(-1).*(cos(q5).*(cos(q4).*(cos( ...
  q2).*cos(q3).*sin(q1)+cos(q1).*sin(q3))+sin(q1).*sin(q2).*sin(q4))+(cos( ...
  q1).*cos(q3)+(-1).*cos(q2).*sin(q1).*sin(q3)).*sin(q5)).*sin(q6));

Jxe227 = 0;

Jxe231 = 0;

Jxe232 = ( ...
  -1).*Kuka_LBR_param_.dblLink23Len.*cos(q2)+Kuka_LBR_param_.dblLink45Len.*((-1).*cos(q2).*cos(q4)+(-1).*cos(q3).*sin(q2).* ...
  sin(q4))+Kuka_LBR_param_.dblLink67Len.*((-1).*cos(q6).*(cos(q2).*cos(q4)+cos(q3).*sin(q2).*sin( ...
  q4))+(cos(q5).*(cos(q3).*cos(q4).*sin(q2)+(-1).*cos(q2).*sin(q4))+(-1).* ...
  sin(q2).*sin(q3).*sin(q5)).*sin(q6));

Jxe233 = (-1).*Kuka_LBR_param_.dblLink45Len.*cos(q3).*sin(q2).*sin( ...
  q4)+Kuka_LBR_param_.dblLink67Len.*((-1).*cos(q3).*cos(q6).*sin(q2).*sin(q4)+(cos(q3).*cos(q4).* ...
  cos(q5).*sin(q2)+(-1).*sin(q2).*sin(q3).*sin(q5)).*sin(q6));

Jxe234 = Kuka_LBR_param_.dblLink45Len.*((-1).* ...
  cos(q2).*cos(q4)+(-1).*cos(q3).*sin(q2).*sin(q4))+Kuka_LBR_param_.dblLink67Len.*((-1).*cos(q6).*( ...
  cos(q2).*cos(q4)+cos(q3).*sin(q2).*sin(q4))+cos(q5).*(cos(q3).*cos(q4).* ...
  sin(q2)+(-1).*cos(q2).*sin(q4)).*sin(q6));

Jxe235 = Kuka_LBR_param_.dblLink67Len.*((-1).*cos(q5).*((-1).* ...
  cos(q3).*cos(q4).*sin(q2)+cos(q2).*sin(q4))+(-1).*sin(q2).*sin(q3).*sin( ...
  q5)).*sin(q6);

Jxe236 = Kuka_LBR_param_.dblLink67Len.*(cos(q6).*((-1).*cos(q2).*cos(q4)+(-1).*cos(q3).*sin( ...
  q2).*sin(q4))+(-1).*(cos(q5).*((-1).*cos(q3).*cos(q4).*sin(q2)+cos(q2).* ...
  sin(q4))+sin(q2).*sin(q3).*sin(q5)).*sin(q6));

Jxe237 = 0;

Jxe241 = ((-1).*(cos(q7).*(cos( ...
  q6).*(cos(q5).*(cos(q4).*(cos(q1).*cos(q2).*cos(q3)+(-1).*sin(q1).*sin( ...
  q3))+cos(q1).*sin(q2).*sin(q4))+((-1).*cos(q3).*sin(q1)+(-1).*cos(q1).* ...
  cos(q2).*sin(q3)).*sin(q5))+((-1).*cos(q1).*cos(q4).*sin(q2)+(cos(q1).* ...
  cos(q2).*cos(q3)+(-1).*sin(q1).*sin(q3)).*sin(q4)).*sin(q6))+(cos(q5).*( ...
  (-1).*cos(q3).*sin(q1)+(-1).*cos(q1).*cos(q2).*sin(q3))+(-1).*(cos(q4).* ...
  (cos(q1).*cos(q2).*cos(q3)+(-1).*sin(q1).*sin(q3))+cos(q1).*sin(q2).* ...
  sin(q4)).*sin(q5)).*sin(q7)).^(-1).*(cos(q7).*(cos(q6).*(cos(q5).*(cos( ...
  q4).*((-1).*cos(q2).*cos(q3).*sin(q1)+(-1).*cos(q1).*sin(q3))+(-1).*sin( ...
  q1).*sin(q2).*sin(q4))+((-1).*cos(q1).*cos(q3)+cos(q2).*sin(q1).*sin(q3) ...
  ).*sin(q5))+(cos(q4).*sin(q1).*sin(q2)+((-1).*cos(q2).*cos(q3).*sin(q1)+ ...
  (-1).*cos(q1).*sin(q3)).*sin(q4)).*sin(q6))+(cos(q5).*((-1).*cos(q1).* ...
  cos(q3)+cos(q2).*sin(q1).*sin(q3))+(-1).*(cos(q4).*((-1).*cos(q2).*cos( ...
  q3).*sin(q1)+(-1).*cos(q1).*sin(q3))+(-1).*sin(q1).*sin(q2).*sin(q4)).* ...
  sin(q5)).*sin(q7))+(-1).*(cos(q7).*(cos(q6).*(cos(q5).*(cos(q4).*((-1).* ...
  cos(q1).*cos(q2).*cos(q3)+sin(q1).*sin(q3))+(-1).*cos(q1).*sin(q2).*sin( ...
  q4))+(cos(q3).*sin(q1)+cos(q1).*cos(q2).*sin(q3)).*sin(q5))+(cos(q1).* ...
  cos(q4).*sin(q2)+((-1).*cos(q1).*cos(q2).*cos(q3)+sin(q1).*sin(q3)).* ...
  sin(q4)).*sin(q6))+(cos(q5).*(cos(q3).*sin(q1)+cos(q1).*cos(q2).*sin(q3) ...
  )+(-1).*(cos(q4).*((-1).*cos(q1).*cos(q2).*cos(q3)+sin(q1).*sin(q3))+( ...
  -1).*cos(q1).*sin(q2).*sin(q4)).*sin(q5)).*sin(q7)).*(cos(q7).*(cos(q6) ...
  .*(cos(q5).*(cos(q4).*(cos(q1).*cos(q2).*cos(q3)+(-1).*sin(q1).*sin(q3)) ...
  +cos(q1).*sin(q2).*sin(q4))+((-1).*cos(q3).*sin(q1)+(-1).*cos(q1).*cos( ...
  q2).*sin(q3)).*sin(q5))+((-1).*cos(q1).*cos(q4).*sin(q2)+(cos(q1).*cos( ...
  q2).*cos(q3)+(-1).*sin(q1).*sin(q3)).*sin(q4)).*sin(q6))+(cos(q5).*((-1) ...
  .*cos(q3).*sin(q1)+(-1).*cos(q1).*cos(q2).*sin(q3))+(-1).*(cos(q4).*( ...
  cos(q1).*cos(q2).*cos(q3)+(-1).*sin(q1).*sin(q3))+cos(q1).*sin(q2).*sin( ...
  q4)).*sin(q5)).*sin(q7)).^(-2).*(cos(q7).*(cos(q6).*(cos(q5).*(cos(q4).* ...
  (cos(q2).*cos(q3).*sin(q1)+cos(q1).*sin(q3))+sin(q1).*sin(q2).*sin(q4))+ ...
  (cos(q1).*cos(q3)+(-1).*cos(q2).*sin(q1).*sin(q3)).*sin(q5))+((-1).*cos( ...
  q4).*sin(q1).*sin(q2)+(cos(q2).*cos(q3).*sin(q1)+cos(q1).*sin(q3)).*sin( ...
  q4)).*sin(q6))+(cos(q5).*(cos(q1).*cos(q3)+(-1).*cos(q2).*sin(q1).*sin( ...
  q3))+(-1).*(cos(q4).*(cos(q2).*cos(q3).*sin(q1)+cos(q1).*sin(q3))+sin( ...
  q1).*sin(q2).*sin(q4)).*sin(q5)).*sin(q7))+2.*(cos(q7).*(cos(q6).*(cos( ...
  q5).*(cos(q4).*(cos(q1).*cos(q2).*cos(q3)+(-1).*sin(q1).*sin(q3))+cos( ...
  q1).*sin(q2).*sin(q4))+((-1).*cos(q3).*sin(q1)+(-1).*cos(q1).*cos(q2).* ...
  sin(q3)).*sin(q5))+((-1).*cos(q1).*cos(q4).*sin(q2)+(cos(q1).*cos(q2).* ...
  cos(q3)+(-1).*sin(q1).*sin(q3)).*sin(q4)).*sin(q6))+(cos(q5).*((-1).* ...
  cos(q3).*sin(q1)+(-1).*cos(q1).*cos(q2).*sin(q3))+(-1).*(cos(q4).*(cos( ...
  q1).*cos(q2).*cos(q3)+(-1).*sin(q1).*sin(q3))+cos(q1).*sin(q2).*sin(q4)) ...
  .*sin(q5)).*sin(q7)).^(-3).*(cos(q7).*(cos(q6).*(cos(q5).*(cos(q4).*(( ...
  -1).*cos(q2).*cos(q3).*sin(q1)+(-1).*cos(q1).*sin(q3))+(-1).*sin(q1).* ...
  sin(q2).*sin(q4))+((-1).*cos(q1).*cos(q3)+cos(q2).*sin(q1).*sin(q3)).* ...
  sin(q5))+(cos(q4).*sin(q1).*sin(q2)+((-1).*cos(q2).*cos(q3).*sin(q1)+( ...
  -1).*cos(q1).*sin(q3)).*sin(q4)).*sin(q6))+(cos(q5).*((-1).*cos(q1).* ...
  cos(q3)+cos(q2).*sin(q1).*sin(q3))+(-1).*(cos(q4).*((-1).*cos(q2).*cos( ...
  q3).*sin(q1)+(-1).*cos(q1).*sin(q3))+(-1).*sin(q1).*sin(q2).*sin(q4)).* ...
  sin(q5)).*sin(q7)).^2.*(cos(q7).*(cos(q6).*(cos(q5).*(cos(q4).*(cos(q2) ...
  .*cos(q3).*sin(q1)+cos(q1).*sin(q3))+sin(q1).*sin(q2).*sin(q4))+(cos(q1) ...
  .*cos(q3)+(-1).*cos(q2).*sin(q1).*sin(q3)).*sin(q5))+((-1).*cos(q4).* ...
  sin(q1).*sin(q2)+(cos(q2).*cos(q3).*sin(q1)+cos(q1).*sin(q3)).*sin(q4)) ...
  .*sin(q6))+(cos(q5).*(cos(q1).*cos(q3)+(-1).*cos(q2).*sin(q1).*sin(q3))+ ...
  (-1).*(cos(q4).*(cos(q2).*cos(q3).*sin(q1)+cos(q1).*sin(q3))+sin(q1).* ...
  sin(q2).*sin(q4)).*sin(q5)).*sin(q7))).*(1+(cos(q7).*(cos(q6).*(cos(q5) ...
  .*(cos(q4).*(cos(q1).*cos(q2).*cos(q3)+(-1).*sin(q1).*sin(q3))+cos(q1).* ...
  sin(q2).*sin(q4))+((-1).*cos(q3).*sin(q1)+(-1).*cos(q1).*cos(q2).*sin( ...
  q3)).*sin(q5))+((-1).*cos(q1).*cos(q4).*sin(q2)+(cos(q1).*cos(q2).*cos( ...
  q3)+(-1).*sin(q1).*sin(q3)).*sin(q4)).*sin(q6))+(cos(q5).*((-1).*cos(q3) ...
  .*sin(q1)+(-1).*cos(q1).*cos(q2).*sin(q3))+(-1).*(cos(q4).*(cos(q1).* ...
  cos(q2).*cos(q3)+(-1).*sin(q1).*sin(q3))+cos(q1).*sin(q2).*sin(q4)).* ...
  sin(q5)).*sin(q7)).^(-2).*(cos(q7).*(cos(q6).*(cos(q5).*(cos(q4).*(cos( ...
  q2).*cos(q3).*sin(q1)+cos(q1).*sin(q3))+sin(q1).*sin(q2).*sin(q4))+(cos( ...
  q1).*cos(q3)+(-1).*cos(q2).*sin(q1).*sin(q3)).*sin(q5))+((-1).*cos(q4).* ...
  sin(q1).*sin(q2)+(cos(q2).*cos(q3).*sin(q1)+cos(q1).*sin(q3)).*sin(q4)) ...
  .*sin(q6))+(cos(q5).*(cos(q1).*cos(q3)+(-1).*cos(q2).*sin(q1).*sin(q3))+ ...
  (-1).*(cos(q4).*(cos(q2).*cos(q3).*sin(q1)+cos(q1).*sin(q3))+sin(q1).* ...
  sin(q2).*sin(q4)).*sin(q5)).*sin(q7)).^2).^(-1)+(-1).*(1+(-1).*(cos(q7) ...
  .*(cos(q6).*(cos(q5).*(cos(q4).*(cos(q1).*cos(q2).*cos(q3)+(-1).*sin(q1) ...
  .*sin(q3))+cos(q1).*sin(q2).*sin(q4))+((-1).*cos(q3).*sin(q1)+(-1).*cos( ...
  q1).*cos(q2).*sin(q3)).*sin(q5))+((-1).*cos(q1).*cos(q4).*sin(q2)+(cos( ...
  q1).*cos(q2).*cos(q3)+(-1).*sin(q1).*sin(q3)).*sin(q4)).*sin(q6))+(cos( ...
  q5).*((-1).*cos(q3).*sin(q1)+(-1).*cos(q1).*cos(q2).*sin(q3))+(-1).*( ...
  cos(q4).*(cos(q1).*cos(q2).*cos(q3)+(-1).*sin(q1).*sin(q3))+cos(q1).* ...
  sin(q2).*sin(q4)).*sin(q5)).*sin(q7)).^(-2).*(cos(q7).*(cos(q6).*(cos( ...
  q5).*(cos(q4).*((-1).*cos(q2).*cos(q3).*sin(q1)+(-1).*cos(q1).*sin(q3))+ ...
  (-1).*sin(q1).*sin(q2).*sin(q4))+((-1).*cos(q1).*cos(q3)+cos(q2).*sin( ...
  q1).*sin(q3)).*sin(q5))+(cos(q4).*sin(q1).*sin(q2)+((-1).*cos(q2).*cos( ...
  q3).*sin(q1)+(-1).*cos(q1).*sin(q3)).*sin(q4)).*sin(q6))+(cos(q5).*((-1) ...
  .*cos(q1).*cos(q3)+cos(q2).*sin(q1).*sin(q3))+(-1).*(cos(q4).*((-1).* ...
  cos(q2).*cos(q3).*sin(q1)+(-1).*cos(q1).*sin(q3))+(-1).*sin(q1).*sin(q2) ...
  .*sin(q4)).*sin(q5)).*sin(q7)).*(cos(q7).*(cos(q6).*(cos(q5).*(cos(q4).* ...
  (cos(q2).*cos(q3).*sin(q1)+cos(q1).*sin(q3))+sin(q1).*sin(q2).*sin(q4))+ ...
  (cos(q1).*cos(q3)+(-1).*cos(q2).*sin(q1).*sin(q3)).*sin(q5))+((-1).*cos( ...
  q4).*sin(q1).*sin(q2)+(cos(q2).*cos(q3).*sin(q1)+cos(q1).*sin(q3)).*sin( ...
  q4)).*sin(q6))+(cos(q5).*(cos(q1).*cos(q3)+(-1).*cos(q2).*sin(q1).*sin( ...
  q3))+(-1).*(cos(q4).*(cos(q2).*cos(q3).*sin(q1)+cos(q1).*sin(q3))+sin( ...
  q1).*sin(q2).*sin(q4)).*sin(q5)).*sin(q7))).*(1+(cos(q7).*(cos(q6).*( ...
  cos(q5).*(cos(q4).*(cos(q1).*cos(q2).*cos(q3)+(-1).*sin(q1).*sin(q3))+ ...
  cos(q1).*sin(q2).*sin(q4))+((-1).*cos(q3).*sin(q1)+(-1).*cos(q1).*cos( ...
  q2).*sin(q3)).*sin(q5))+((-1).*cos(q1).*cos(q4).*sin(q2)+(cos(q1).*cos( ...
  q2).*cos(q3)+(-1).*sin(q1).*sin(q3)).*sin(q4)).*sin(q6))+(cos(q5).*((-1) ...
  .*cos(q3).*sin(q1)+(-1).*cos(q1).*cos(q2).*sin(q3))+(-1).*(cos(q4).*( ...
  cos(q1).*cos(q2).*cos(q3)+(-1).*sin(q1).*sin(q3))+cos(q1).*sin(q2).*sin( ...
  q4)).*sin(q5)).*sin(q7)).^(-2).*(cos(q7).*(cos(q6).*(cos(q5).*(cos(q4).* ...
  (cos(q2).*cos(q3).*sin(q1)+cos(q1).*sin(q3))+sin(q1).*sin(q2).*sin(q4))+ ...
  (cos(q1).*cos(q3)+(-1).*cos(q2).*sin(q1).*sin(q3)).*sin(q5))+((-1).*cos( ...
  q4).*sin(q1).*sin(q2)+(cos(q2).*cos(q3).*sin(q1)+cos(q1).*sin(q3)).*sin( ...
  q4)).*sin(q6))+(cos(q5).*(cos(q1).*cos(q3)+(-1).*cos(q2).*sin(q1).*sin( ...
  q3))+(-1).*(cos(q4).*(cos(q2).*cos(q3).*sin(q1)+cos(q1).*sin(q3))+sin( ...
  q1).*sin(q2).*sin(q4)).*sin(q5)).*sin(q7)).^2).^(-2).*(2.*(cos(q7).*( ...
  cos(q6).*(cos(q5).*(cos(q4).*(cos(q1).*cos(q2).*cos(q3)+(-1).*sin(q1).* ...
  sin(q3))+cos(q1).*sin(q2).*sin(q4))+((-1).*cos(q3).*sin(q1)+(-1).*cos( ...
  q1).*cos(q2).*sin(q3)).*sin(q5))+((-1).*cos(q1).*cos(q4).*sin(q2)+(cos( ...
  q1).*cos(q2).*cos(q3)+(-1).*sin(q1).*sin(q3)).*sin(q4)).*sin(q6))+(cos( ...
  q5).*((-1).*cos(q3).*sin(q1)+(-1).*cos(q1).*cos(q2).*sin(q3))+(-1).*( ...
  cos(q4).*(cos(q1).*cos(q2).*cos(q3)+(-1).*sin(q1).*sin(q3))+cos(q1).* ...
  sin(q2).*sin(q4)).*sin(q5)).*sin(q7)).^(-1).*(cos(q7).*(cos(q6).*(cos( ...
  q5).*(cos(q4).*(cos(q2).*cos(q3).*sin(q1)+cos(q1).*sin(q3))+sin(q1).* ...
  sin(q2).*sin(q4))+(cos(q1).*cos(q3)+(-1).*cos(q2).*sin(q1).*sin(q3)).* ...
  sin(q5))+((-1).*cos(q4).*sin(q1).*sin(q2)+(cos(q2).*cos(q3).*sin(q1)+ ...
  cos(q1).*sin(q3)).*sin(q4)).*sin(q6))+(cos(q5).*(cos(q1).*cos(q3)+(-1).* ...
  cos(q2).*sin(q1).*sin(q3))+(-1).*(cos(q4).*(cos(q2).*cos(q3).*sin(q1)+ ...
  cos(q1).*sin(q3))+sin(q1).*sin(q2).*sin(q4)).*sin(q5)).*sin(q7))+(-2).*( ...
  cos(q7).*(cos(q6).*(cos(q5).*(cos(q4).*(cos(q1).*cos(q2).*cos(q3)+(-1).* ...
  sin(q1).*sin(q3))+cos(q1).*sin(q2).*sin(q4))+((-1).*cos(q3).*sin(q1)+( ...
  -1).*cos(q1).*cos(q2).*sin(q3)).*sin(q5))+((-1).*cos(q1).*cos(q4).*sin( ...
  q2)+(cos(q1).*cos(q2).*cos(q3)+(-1).*sin(q1).*sin(q3)).*sin(q4)).*sin( ...
  q6))+(cos(q5).*((-1).*cos(q3).*sin(q1)+(-1).*cos(q1).*cos(q2).*sin(q3))+ ...
  (-1).*(cos(q4).*(cos(q1).*cos(q2).*cos(q3)+(-1).*sin(q1).*sin(q3))+cos( ...
  q1).*sin(q2).*sin(q4)).*sin(q5)).*sin(q7)).^(-3).*(cos(q7).*(cos(q6).*( ...
  cos(q5).*(cos(q4).*((-1).*cos(q2).*cos(q3).*sin(q1)+(-1).*cos(q1).*sin( ...
  q3))+(-1).*sin(q1).*sin(q2).*sin(q4))+((-1).*cos(q1).*cos(q3)+cos(q2).* ...
  sin(q1).*sin(q3)).*sin(q5))+(cos(q4).*sin(q1).*sin(q2)+((-1).*cos(q2).* ...
  cos(q3).*sin(q1)+(-1).*cos(q1).*sin(q3)).*sin(q4)).*sin(q6))+(cos(q5).*( ...
  (-1).*cos(q1).*cos(q3)+cos(q2).*sin(q1).*sin(q3))+(-1).*(cos(q4).*((-1) ...
  .*cos(q2).*cos(q3).*sin(q1)+(-1).*cos(q1).*sin(q3))+(-1).*sin(q1).*sin( ...
  q2).*sin(q4)).*sin(q5)).*sin(q7)).*(cos(q7).*(cos(q6).*(cos(q5).*(cos( ...
  q4).*(cos(q2).*cos(q3).*sin(q1)+cos(q1).*sin(q3))+sin(q1).*sin(q2).*sin( ...
  q4))+(cos(q1).*cos(q3)+(-1).*cos(q2).*sin(q1).*sin(q3)).*sin(q5))+((-1) ...
  .*cos(q4).*sin(q1).*sin(q2)+(cos(q2).*cos(q3).*sin(q1)+cos(q1).*sin(q3)) ...
  .*sin(q4)).*sin(q6))+(cos(q5).*(cos(q1).*cos(q3)+(-1).*cos(q2).*sin(q1) ...
  .*sin(q3))+(-1).*(cos(q4).*(cos(q2).*cos(q3).*sin(q1)+cos(q1).*sin(q3))+ ...
  sin(q1).*sin(q2).*sin(q4)).*sin(q5)).*sin(q7)).^2);

Jxe242 = (-1).*((cos(q7).*( ...
  cos(q6).*(cos(q5).*((-1).*cos(q3).*cos(q4).*sin(q1).*sin(q2)+cos(q2).* ...
  sin(q1).*sin(q4))+sin(q1).*sin(q2).*sin(q3).*sin(q5))+((-1).*cos(q2).* ...
  cos(q4).*sin(q1)+(-1).*cos(q3).*sin(q1).*sin(q2).*sin(q4)).*sin(q6))+( ...
  cos(q5).*sin(q1).*sin(q2).*sin(q3)+(-1).*((-1).*cos(q3).*cos(q4).*sin( ...
  q1).*sin(q2)+cos(q2).*sin(q1).*sin(q4)).*sin(q5)).*sin(q7)).*(cos(q7).*( ...
  cos(q6).*(cos(q5).*(cos(q4).*(cos(q1).*cos(q2).*cos(q3)+(-1).*sin(q1).* ...
  sin(q3))+cos(q1).*sin(q2).*sin(q4))+((-1).*cos(q3).*sin(q1)+(-1).*cos( ...
  q1).*cos(q2).*sin(q3)).*sin(q5))+((-1).*cos(q1).*cos(q4).*sin(q2)+(cos( ...
  q1).*cos(q2).*cos(q3)+(-1).*sin(q1).*sin(q3)).*sin(q4)).*sin(q6))+(cos( ...
  q5).*((-1).*cos(q3).*sin(q1)+(-1).*cos(q1).*cos(q2).*sin(q3))+(-1).*( ...
  cos(q4).*(cos(q1).*cos(q2).*cos(q3)+(-1).*sin(q1).*sin(q3))+cos(q1).* ...
  sin(q2).*sin(q4)).*sin(q5)).*sin(q7)).^(-1)+(-1).*(cos(q7).*(cos(q6).*( ...
  cos(q5).*((-1).*cos(q1).*cos(q3).*cos(q4).*sin(q2)+cos(q1).*cos(q2).* ...
  sin(q4))+cos(q1).*sin(q2).*sin(q3).*sin(q5))+((-1).*cos(q1).*cos(q2).* ...
  cos(q4)+(-1).*cos(q1).*cos(q3).*sin(q2).*sin(q4)).*sin(q6))+(cos(q1).* ...
  cos(q5).*sin(q2).*sin(q3)+(-1).*((-1).*cos(q1).*cos(q3).*cos(q4).*sin( ...
  q2)+cos(q1).*cos(q2).*sin(q4)).*sin(q5)).*sin(q7)).*(cos(q7).*(cos(q6).* ...
  (cos(q5).*(cos(q4).*(cos(q1).*cos(q2).*cos(q3)+(-1).*sin(q1).*sin(q3))+ ...
  cos(q1).*sin(q2).*sin(q4))+((-1).*cos(q3).*sin(q1)+(-1).*cos(q1).*cos( ...
  q2).*sin(q3)).*sin(q5))+((-1).*cos(q1).*cos(q4).*sin(q2)+(cos(q1).*cos( ...
  q2).*cos(q3)+(-1).*sin(q1).*sin(q3)).*sin(q4)).*sin(q6))+(cos(q5).*((-1) ...
  .*cos(q3).*sin(q1)+(-1).*cos(q1).*cos(q2).*sin(q3))+(-1).*(cos(q4).*( ...
  cos(q1).*cos(q2).*cos(q3)+(-1).*sin(q1).*sin(q3))+cos(q1).*sin(q2).*sin( ...
  q4)).*sin(q5)).*sin(q7)).^(-2).*(cos(q7).*(cos(q6).*(cos(q5).*(cos(q4).* ...
  (cos(q2).*cos(q3).*sin(q1)+cos(q1).*sin(q3))+sin(q1).*sin(q2).*sin(q4))+ ...
  (cos(q1).*cos(q3)+(-1).*cos(q2).*sin(q1).*sin(q3)).*sin(q5))+((-1).*cos( ...
  q4).*sin(q1).*sin(q2)+(cos(q2).*cos(q3).*sin(q1)+cos(q1).*sin(q3)).*sin( ...
  q4)).*sin(q6))+(cos(q5).*(cos(q1).*cos(q3)+(-1).*cos(q2).*sin(q1).*sin( ...
  q3))+(-1).*(cos(q4).*(cos(q2).*cos(q3).*sin(q1)+cos(q1).*sin(q3))+sin( ...
  q1).*sin(q2).*sin(q4)).*sin(q5)).*sin(q7))).*(2.*(cos(q7).*(cos(q6).*( ...
  cos(q5).*((-1).*cos(q3).*cos(q4).*sin(q1).*sin(q2)+cos(q2).*sin(q1).* ...
  sin(q4))+sin(q1).*sin(q2).*sin(q3).*sin(q5))+((-1).*cos(q2).*cos(q4).* ...
  sin(q1)+(-1).*cos(q3).*sin(q1).*sin(q2).*sin(q4)).*sin(q6))+(cos(q5).* ...
  sin(q1).*sin(q2).*sin(q3)+(-1).*((-1).*cos(q3).*cos(q4).*sin(q1).*sin( ...
  q2)+cos(q2).*sin(q1).*sin(q4)).*sin(q5)).*sin(q7)).*(cos(q7).*(cos(q6).* ...
  (cos(q5).*(cos(q4).*(cos(q1).*cos(q2).*cos(q3)+(-1).*sin(q1).*sin(q3))+ ...
  cos(q1).*sin(q2).*sin(q4))+((-1).*cos(q3).*sin(q1)+(-1).*cos(q1).*cos( ...
  q2).*sin(q3)).*sin(q5))+((-1).*cos(q1).*cos(q4).*sin(q2)+(cos(q1).*cos( ...
  q2).*cos(q3)+(-1).*sin(q1).*sin(q3)).*sin(q4)).*sin(q6))+(cos(q5).*((-1) ...
  .*cos(q3).*sin(q1)+(-1).*cos(q1).*cos(q2).*sin(q3))+(-1).*(cos(q4).*( ...
  cos(q1).*cos(q2).*cos(q3)+(-1).*sin(q1).*sin(q3))+cos(q1).*sin(q2).*sin( ...
  q4)).*sin(q5)).*sin(q7)).^(-2).*(cos(q7).*(cos(q6).*(cos(q5).*(cos(q4).* ...
  (cos(q2).*cos(q3).*sin(q1)+cos(q1).*sin(q3))+sin(q1).*sin(q2).*sin(q4))+ ...
  (cos(q1).*cos(q3)+(-1).*cos(q2).*sin(q1).*sin(q3)).*sin(q5))+((-1).*cos( ...
  q4).*sin(q1).*sin(q2)+(cos(q2).*cos(q3).*sin(q1)+cos(q1).*sin(q3)).*sin( ...
  q4)).*sin(q6))+(cos(q5).*(cos(q1).*cos(q3)+(-1).*cos(q2).*sin(q1).*sin( ...
  q3))+(-1).*(cos(q4).*(cos(q2).*cos(q3).*sin(q1)+cos(q1).*sin(q3))+sin( ...
  q1).*sin(q2).*sin(q4)).*sin(q5)).*sin(q7))+(-2).*(cos(q7).*(cos(q6).*( ...
  cos(q5).*((-1).*cos(q1).*cos(q3).*cos(q4).*sin(q2)+cos(q1).*cos(q2).* ...
  sin(q4))+cos(q1).*sin(q2).*sin(q3).*sin(q5))+((-1).*cos(q1).*cos(q2).* ...
  cos(q4)+(-1).*cos(q1).*cos(q3).*sin(q2).*sin(q4)).*sin(q6))+(cos(q1).* ...
  cos(q5).*sin(q2).*sin(q3)+(-1).*((-1).*cos(q1).*cos(q3).*cos(q4).*sin( ...
  q2)+cos(q1).*cos(q2).*sin(q4)).*sin(q5)).*sin(q7)).*(cos(q7).*(cos(q6).* ...
  (cos(q5).*(cos(q4).*(cos(q1).*cos(q2).*cos(q3)+(-1).*sin(q1).*sin(q3))+ ...
  cos(q1).*sin(q2).*sin(q4))+((-1).*cos(q3).*sin(q1)+(-1).*cos(q1).*cos( ...
  q2).*sin(q3)).*sin(q5))+((-1).*cos(q1).*cos(q4).*sin(q2)+(cos(q1).*cos( ...
  q2).*cos(q3)+(-1).*sin(q1).*sin(q3)).*sin(q4)).*sin(q6))+(cos(q5).*((-1) ...
  .*cos(q3).*sin(q1)+(-1).*cos(q1).*cos(q2).*sin(q3))+(-1).*(cos(q4).*( ...
  cos(q1).*cos(q2).*cos(q3)+(-1).*sin(q1).*sin(q3))+cos(q1).*sin(q2).*sin( ...
  q4)).*sin(q5)).*sin(q7)).^(-3).*(cos(q7).*(cos(q6).*(cos(q5).*(cos(q4).* ...
  (cos(q2).*cos(q3).*sin(q1)+cos(q1).*sin(q3))+sin(q1).*sin(q2).*sin(q4))+ ...
  (cos(q1).*cos(q3)+(-1).*cos(q2).*sin(q1).*sin(q3)).*sin(q5))+((-1).*cos( ...
  q4).*sin(q1).*sin(q2)+(cos(q2).*cos(q3).*sin(q1)+cos(q1).*sin(q3)).*sin( ...
  q4)).*sin(q6))+(cos(q5).*(cos(q1).*cos(q3)+(-1).*cos(q2).*sin(q1).*sin( ...
  q3))+(-1).*(cos(q4).*(cos(q2).*cos(q3).*sin(q1)+cos(q1).*sin(q3))+sin( ...
  q1).*sin(q2).*sin(q4)).*sin(q5)).*sin(q7)).^2).*(1+(cos(q7).*(cos(q6).*( ...
  cos(q5).*(cos(q4).*(cos(q1).*cos(q2).*cos(q3)+(-1).*sin(q1).*sin(q3))+ ...
  cos(q1).*sin(q2).*sin(q4))+((-1).*cos(q3).*sin(q1)+(-1).*cos(q1).*cos( ...
  q2).*sin(q3)).*sin(q5))+((-1).*cos(q1).*cos(q4).*sin(q2)+(cos(q1).*cos( ...
  q2).*cos(q3)+(-1).*sin(q1).*sin(q3)).*sin(q4)).*sin(q6))+(cos(q5).*((-1) ...
  .*cos(q3).*sin(q1)+(-1).*cos(q1).*cos(q2).*sin(q3))+(-1).*(cos(q4).*( ...
  cos(q1).*cos(q2).*cos(q3)+(-1).*sin(q1).*sin(q3))+cos(q1).*sin(q2).*sin( ...
  q4)).*sin(q5)).*sin(q7)).^(-2).*(cos(q7).*(cos(q6).*(cos(q5).*(cos(q4).* ...
  (cos(q2).*cos(q3).*sin(q1)+cos(q1).*sin(q3))+sin(q1).*sin(q2).*sin(q4))+ ...
  (cos(q1).*cos(q3)+(-1).*cos(q2).*sin(q1).*sin(q3)).*sin(q5))+((-1).*cos( ...
  q4).*sin(q1).*sin(q2)+(cos(q2).*cos(q3).*sin(q1)+cos(q1).*sin(q3)).*sin( ...
  q4)).*sin(q6))+(cos(q5).*(cos(q1).*cos(q3)+(-1).*cos(q2).*sin(q1).*sin( ...
  q3))+(-1).*(cos(q4).*(cos(q2).*cos(q3).*sin(q1)+cos(q1).*sin(q3))+sin( ...
  q1).*sin(q2).*sin(q4)).*sin(q5)).*sin(q7)).^2).^(-2)+((-2).*(cos(q7).*( ...
  cos(q6).*(cos(q5).*((-1).*cos(q1).*cos(q3).*cos(q4).*sin(q2)+cos(q1).* ...
  cos(q2).*sin(q4))+cos(q1).*sin(q2).*sin(q3).*sin(q5))+((-1).*cos(q1).* ...
  cos(q2).*cos(q4)+(-1).*cos(q1).*cos(q3).*sin(q2).*sin(q4)).*sin(q6))+( ...
  cos(q1).*cos(q5).*sin(q2).*sin(q3)+(-1).*((-1).*cos(q1).*cos(q3).*cos( ...
  q4).*sin(q2)+cos(q1).*cos(q2).*sin(q4)).*sin(q5)).*sin(q7)).*(cos(q7).*( ...
  cos(q6).*(cos(q5).*((-1).*cos(q3).*cos(q4).*sin(q1).*sin(q2)+cos(q2).* ...
  sin(q1).*sin(q4))+sin(q1).*sin(q2).*sin(q3).*sin(q5))+((-1).*cos(q2).* ...
  cos(q4).*sin(q1)+(-1).*cos(q3).*sin(q1).*sin(q2).*sin(q4)).*sin(q6))+( ...
  cos(q5).*sin(q1).*sin(q2).*sin(q3)+(-1).*((-1).*cos(q3).*cos(q4).*sin( ...
  q1).*sin(q2)+cos(q2).*sin(q1).*sin(q4)).*sin(q5)).*sin(q7)).*(cos(q7).*( ...
  cos(q6).*(cos(q5).*(cos(q4).*(cos(q1).*cos(q2).*cos(q3)+(-1).*sin(q1).* ...
  sin(q3))+cos(q1).*sin(q2).*sin(q4))+((-1).*cos(q3).*sin(q1)+(-1).*cos( ...
  q1).*cos(q2).*sin(q3)).*sin(q5))+((-1).*cos(q1).*cos(q4).*sin(q2)+(cos( ...
  q1).*cos(q2).*cos(q3)+(-1).*sin(q1).*sin(q3)).*sin(q4)).*sin(q6))+(cos( ...
  q5).*((-1).*cos(q3).*sin(q1)+(-1).*cos(q1).*cos(q2).*sin(q3))+(-1).*( ...
  cos(q4).*(cos(q1).*cos(q2).*cos(q3)+(-1).*sin(q1).*sin(q3))+cos(q1).* ...
  sin(q2).*sin(q4)).*sin(q5)).*sin(q7)).^(-2)+(cos(q7).*(cos(q6).*(cos(q5) ...
  .*(cos(q4).*(cos(q1).*cos(q2).*cos(q3)+(-1).*sin(q1).*sin(q3))+cos(q1).* ...
  sin(q2).*sin(q4))+((-1).*cos(q3).*sin(q1)+(-1).*cos(q1).*cos(q2).*sin( ...
  q3)).*sin(q5))+((-1).*cos(q1).*cos(q4).*sin(q2)+(cos(q1).*cos(q2).*cos( ...
  q3)+(-1).*sin(q1).*sin(q3)).*sin(q4)).*sin(q6))+(cos(q5).*((-1).*cos(q3) ...
  .*sin(q1)+(-1).*cos(q1).*cos(q2).*sin(q3))+(-1).*(cos(q4).*(cos(q1).* ...
  cos(q2).*cos(q3)+(-1).*sin(q1).*sin(q3))+cos(q1).*sin(q2).*sin(q4)).* ...
  sin(q5)).*sin(q7)).^(-1).*(cos(q7).*(cos(q6).*(cos(q5).*((-1).*cos(q2).* ...
  cos(q3).*cos(q4).*sin(q1)+(-1).*sin(q1).*sin(q2).*sin(q4))+cos(q2).*sin( ...
  q1).*sin(q3).*sin(q5))+(cos(q4).*sin(q1).*sin(q2)+(-1).*cos(q2).*cos(q3) ...
  .*sin(q1).*sin(q4)).*sin(q6))+(cos(q2).*cos(q5).*sin(q1).*sin(q3)+(-1).* ...
  ((-1).*cos(q2).*cos(q3).*cos(q4).*sin(q1)+(-1).*sin(q1).*sin(q2).*sin( ...
  q4)).*sin(q5)).*sin(q7))+2.*(cos(q7).*(cos(q6).*(cos(q5).*((-1).*cos(q1) ...
  .*cos(q3).*cos(q4).*sin(q2)+cos(q1).*cos(q2).*sin(q4))+cos(q1).*sin(q2) ...
  .*sin(q3).*sin(q5))+((-1).*cos(q1).*cos(q2).*cos(q4)+(-1).*cos(q1).*cos( ...
  q3).*sin(q2).*sin(q4)).*sin(q6))+(cos(q1).*cos(q5).*sin(q2).*sin(q3)+( ...
  -1).*((-1).*cos(q1).*cos(q3).*cos(q4).*sin(q2)+cos(q1).*cos(q2).*sin(q4) ...
  ).*sin(q5)).*sin(q7)).^2.*(cos(q7).*(cos(q6).*(cos(q5).*(cos(q4).*(cos( ...
  q1).*cos(q2).*cos(q3)+(-1).*sin(q1).*sin(q3))+cos(q1).*sin(q2).*sin(q4)) ...
  +((-1).*cos(q3).*sin(q1)+(-1).*cos(q1).*cos(q2).*sin(q3)).*sin(q5))+(( ...
  -1).*cos(q1).*cos(q4).*sin(q2)+(cos(q1).*cos(q2).*cos(q3)+(-1).*sin(q1) ...
  .*sin(q3)).*sin(q4)).*sin(q6))+(cos(q5).*((-1).*cos(q3).*sin(q1)+(-1).* ...
  cos(q1).*cos(q2).*sin(q3))+(-1).*(cos(q4).*(cos(q1).*cos(q2).*cos(q3)+( ...
  -1).*sin(q1).*sin(q3))+cos(q1).*sin(q2).*sin(q4)).*sin(q5)).*sin(q7)).^( ...
  -3).*(cos(q7).*(cos(q6).*(cos(q5).*(cos(q4).*(cos(q2).*cos(q3).*sin(q1)+ ...
  cos(q1).*sin(q3))+sin(q1).*sin(q2).*sin(q4))+(cos(q1).*cos(q3)+(-1).* ...
  cos(q2).*sin(q1).*sin(q3)).*sin(q5))+((-1).*cos(q4).*sin(q1).*sin(q2)+( ...
  cos(q2).*cos(q3).*sin(q1)+cos(q1).*sin(q3)).*sin(q4)).*sin(q6))+(cos(q5) ...
  .*(cos(q1).*cos(q3)+(-1).*cos(q2).*sin(q1).*sin(q3))+(-1).*(cos(q4).*( ...
  cos(q2).*cos(q3).*sin(q1)+cos(q1).*sin(q3))+sin(q1).*sin(q2).*sin(q4)).* ...
  sin(q5)).*sin(q7))+(-1).*(cos(q7).*(cos(q6).*(cos(q5).*((-1).*cos(q1).* ...
  cos(q2).*cos(q3).*cos(q4)+(-1).*cos(q1).*sin(q2).*sin(q4))+cos(q1).*cos( ...
  q2).*sin(q3).*sin(q5))+(cos(q1).*cos(q4).*sin(q2)+(-1).*cos(q1).*cos(q2) ...
  .*cos(q3).*sin(q4)).*sin(q6))+(cos(q1).*cos(q2).*cos(q5).*sin(q3)+(-1).* ...
  ((-1).*cos(q1).*cos(q2).*cos(q3).*cos(q4)+(-1).*cos(q1).*sin(q2).*sin( ...
  q4)).*sin(q5)).*sin(q7)).*(cos(q7).*(cos(q6).*(cos(q5).*(cos(q4).*(cos( ...
  q1).*cos(q2).*cos(q3)+(-1).*sin(q1).*sin(q3))+cos(q1).*sin(q2).*sin(q4)) ...
  +((-1).*cos(q3).*sin(q1)+(-1).*cos(q1).*cos(q2).*sin(q3)).*sin(q5))+(( ...
  -1).*cos(q1).*cos(q4).*sin(q2)+(cos(q1).*cos(q2).*cos(q3)+(-1).*sin(q1) ...
  .*sin(q3)).*sin(q4)).*sin(q6))+(cos(q5).*((-1).*cos(q3).*sin(q1)+(-1).* ...
  cos(q1).*cos(q2).*sin(q3))+(-1).*(cos(q4).*(cos(q1).*cos(q2).*cos(q3)+( ...
  -1).*sin(q1).*sin(q3))+cos(q1).*sin(q2).*sin(q4)).*sin(q5)).*sin(q7)).^( ...
  -2).*(cos(q7).*(cos(q6).*(cos(q5).*(cos(q4).*(cos(q2).*cos(q3).*sin(q1)+ ...
  cos(q1).*sin(q3))+sin(q1).*sin(q2).*sin(q4))+(cos(q1).*cos(q3)+(-1).* ...
  cos(q2).*sin(q1).*sin(q3)).*sin(q5))+((-1).*cos(q4).*sin(q1).*sin(q2)+( ...
  cos(q2).*cos(q3).*sin(q1)+cos(q1).*sin(q3)).*sin(q4)).*sin(q6))+(cos(q5) ...
  .*(cos(q1).*cos(q3)+(-1).*cos(q2).*sin(q1).*sin(q3))+(-1).*(cos(q4).*( ...
  cos(q2).*cos(q3).*sin(q1)+cos(q1).*sin(q3))+sin(q1).*sin(q2).*sin(q4)).* ...
  sin(q5)).*sin(q7))).*(1+(cos(q7).*(cos(q6).*(cos(q5).*(cos(q4).*(cos(q1) ...
  .*cos(q2).*cos(q3)+(-1).*sin(q1).*sin(q3))+cos(q1).*sin(q2).*sin(q4))+(( ...
  -1).*cos(q3).*sin(q1)+(-1).*cos(q1).*cos(q2).*sin(q3)).*sin(q5))+((-1).* ...
  cos(q1).*cos(q4).*sin(q2)+(cos(q1).*cos(q2).*cos(q3)+(-1).*sin(q1).*sin( ...
  q3)).*sin(q4)).*sin(q6))+(cos(q5).*((-1).*cos(q3).*sin(q1)+(-1).*cos(q1) ...
  .*cos(q2).*sin(q3))+(-1).*(cos(q4).*(cos(q1).*cos(q2).*cos(q3)+(-1).* ...
  sin(q1).*sin(q3))+cos(q1).*sin(q2).*sin(q4)).*sin(q5)).*sin(q7)).^(-2).* ...
  (cos(q7).*(cos(q6).*(cos(q5).*(cos(q4).*(cos(q2).*cos(q3).*sin(q1)+cos( ...
  q1).*sin(q3))+sin(q1).*sin(q2).*sin(q4))+(cos(q1).*cos(q3)+(-1).*cos(q2) ...
  .*sin(q1).*sin(q3)).*sin(q5))+((-1).*cos(q4).*sin(q1).*sin(q2)+(cos(q2) ...
  .*cos(q3).*sin(q1)+cos(q1).*sin(q3)).*sin(q4)).*sin(q6))+(cos(q5).*(cos( ...
  q1).*cos(q3)+(-1).*cos(q2).*sin(q1).*sin(q3))+(-1).*(cos(q4).*(cos(q2).* ...
  cos(q3).*sin(q1)+cos(q1).*sin(q3))+sin(q1).*sin(q2).*sin(q4)).*sin(q5)) ...
  .*sin(q7)).^2).^(-1);

Jxe243 = (-1).*((cos(q7).*(cos(q6).*(cos(q4).*cos(q5).*(cos( ...
  q1).*cos(q3)+(-1).*cos(q2).*sin(q1).*sin(q3))+((-1).*cos(q2).*cos(q3).* ...
  sin(q1)+(-1).*cos(q1).*sin(q3)).*sin(q5))+(cos(q1).*cos(q3)+(-1).*cos( ...
  q2).*sin(q1).*sin(q3)).*sin(q4).*sin(q6))+(cos(q5).*((-1).*cos(q2).*cos( ...
  q3).*sin(q1)+(-1).*cos(q1).*sin(q3))+(-1).*cos(q4).*(cos(q1).*cos(q3)+( ...
  -1).*cos(q2).*sin(q1).*sin(q3)).*sin(q5)).*sin(q7)).*(cos(q7).*(cos(q6) ...
  .*(cos(q5).*(cos(q4).*(cos(q1).*cos(q2).*cos(q3)+(-1).*sin(q1).*sin(q3)) ...
  +cos(q1).*sin(q2).*sin(q4))+((-1).*cos(q3).*sin(q1)+(-1).*cos(q1).*cos( ...
  q2).*sin(q3)).*sin(q5))+((-1).*cos(q1).*cos(q4).*sin(q2)+(cos(q1).*cos( ...
  q2).*cos(q3)+(-1).*sin(q1).*sin(q3)).*sin(q4)).*sin(q6))+(cos(q5).*((-1) ...
  .*cos(q3).*sin(q1)+(-1).*cos(q1).*cos(q2).*sin(q3))+(-1).*(cos(q4).*( ...
  cos(q1).*cos(q2).*cos(q3)+(-1).*sin(q1).*sin(q3))+cos(q1).*sin(q2).*sin( ...
  q4)).*sin(q5)).*sin(q7)).^(-1)+(-1).*(cos(q7).*(cos(q6).*(cos(q4).*cos( ...
  q5).*((-1).*cos(q3).*sin(q1)+(-1).*cos(q1).*cos(q2).*sin(q3))+((-1).* ...
  cos(q1).*cos(q2).*cos(q3)+sin(q1).*sin(q3)).*sin(q5))+((-1).*cos(q3).* ...
  sin(q1)+(-1).*cos(q1).*cos(q2).*sin(q3)).*sin(q4).*sin(q6))+(cos(q5).*(( ...
  -1).*cos(q1).*cos(q2).*cos(q3)+sin(q1).*sin(q3))+(-1).*cos(q4).*((-1).* ...
  cos(q3).*sin(q1)+(-1).*cos(q1).*cos(q2).*sin(q3)).*sin(q5)).*sin(q7)).*( ...
  cos(q7).*(cos(q6).*(cos(q5).*(cos(q4).*(cos(q1).*cos(q2).*cos(q3)+(-1).* ...
  sin(q1).*sin(q3))+cos(q1).*sin(q2).*sin(q4))+((-1).*cos(q3).*sin(q1)+( ...
  -1).*cos(q1).*cos(q2).*sin(q3)).*sin(q5))+((-1).*cos(q1).*cos(q4).*sin( ...
  q2)+(cos(q1).*cos(q2).*cos(q3)+(-1).*sin(q1).*sin(q3)).*sin(q4)).*sin( ...
  q6))+(cos(q5).*((-1).*cos(q3).*sin(q1)+(-1).*cos(q1).*cos(q2).*sin(q3))+ ...
  (-1).*(cos(q4).*(cos(q1).*cos(q2).*cos(q3)+(-1).*sin(q1).*sin(q3))+cos( ...
  q1).*sin(q2).*sin(q4)).*sin(q5)).*sin(q7)).^(-2).*(cos(q7).*(cos(q6).*( ...
  cos(q5).*(cos(q4).*(cos(q2).*cos(q3).*sin(q1)+cos(q1).*sin(q3))+sin(q1) ...
  .*sin(q2).*sin(q4))+(cos(q1).*cos(q3)+(-1).*cos(q2).*sin(q1).*sin(q3)).* ...
  sin(q5))+((-1).*cos(q4).*sin(q1).*sin(q2)+(cos(q2).*cos(q3).*sin(q1)+ ...
  cos(q1).*sin(q3)).*sin(q4)).*sin(q6))+(cos(q5).*(cos(q1).*cos(q3)+(-1).* ...
  cos(q2).*sin(q1).*sin(q3))+(-1).*(cos(q4).*(cos(q2).*cos(q3).*sin(q1)+ ...
  cos(q1).*sin(q3))+sin(q1).*sin(q2).*sin(q4)).*sin(q5)).*sin(q7))).*(2.*( ...
  cos(q7).*(cos(q6).*(cos(q4).*cos(q5).*(cos(q1).*cos(q3)+(-1).*cos(q2).* ...
  sin(q1).*sin(q3))+((-1).*cos(q2).*cos(q3).*sin(q1)+(-1).*cos(q1).*sin( ...
  q3)).*sin(q5))+(cos(q1).*cos(q3)+(-1).*cos(q2).*sin(q1).*sin(q3)).*sin( ...
  q4).*sin(q6))+(cos(q5).*((-1).*cos(q2).*cos(q3).*sin(q1)+(-1).*cos(q1).* ...
  sin(q3))+(-1).*cos(q4).*(cos(q1).*cos(q3)+(-1).*cos(q2).*sin(q1).*sin( ...
  q3)).*sin(q5)).*sin(q7)).*(cos(q7).*(cos(q6).*(cos(q5).*(cos(q4).*(cos( ...
  q1).*cos(q2).*cos(q3)+(-1).*sin(q1).*sin(q3))+cos(q1).*sin(q2).*sin(q4)) ...
  +((-1).*cos(q3).*sin(q1)+(-1).*cos(q1).*cos(q2).*sin(q3)).*sin(q5))+(( ...
  -1).*cos(q1).*cos(q4).*sin(q2)+(cos(q1).*cos(q2).*cos(q3)+(-1).*sin(q1) ...
  .*sin(q3)).*sin(q4)).*sin(q6))+(cos(q5).*((-1).*cos(q3).*sin(q1)+(-1).* ...
  cos(q1).*cos(q2).*sin(q3))+(-1).*(cos(q4).*(cos(q1).*cos(q2).*cos(q3)+( ...
  -1).*sin(q1).*sin(q3))+cos(q1).*sin(q2).*sin(q4)).*sin(q5)).*sin(q7)).^( ...
  -2).*(cos(q7).*(cos(q6).*(cos(q5).*(cos(q4).*(cos(q2).*cos(q3).*sin(q1)+ ...
  cos(q1).*sin(q3))+sin(q1).*sin(q2).*sin(q4))+(cos(q1).*cos(q3)+(-1).* ...
  cos(q2).*sin(q1).*sin(q3)).*sin(q5))+((-1).*cos(q4).*sin(q1).*sin(q2)+( ...
  cos(q2).*cos(q3).*sin(q1)+cos(q1).*sin(q3)).*sin(q4)).*sin(q6))+(cos(q5) ...
  .*(cos(q1).*cos(q3)+(-1).*cos(q2).*sin(q1).*sin(q3))+(-1).*(cos(q4).*( ...
  cos(q2).*cos(q3).*sin(q1)+cos(q1).*sin(q3))+sin(q1).*sin(q2).*sin(q4)).* ...
  sin(q5)).*sin(q7))+(-2).*(cos(q7).*(cos(q6).*(cos(q4).*cos(q5).*((-1).* ...
  cos(q3).*sin(q1)+(-1).*cos(q1).*cos(q2).*sin(q3))+((-1).*cos(q1).*cos( ...
  q2).*cos(q3)+sin(q1).*sin(q3)).*sin(q5))+((-1).*cos(q3).*sin(q1)+(-1).* ...
  cos(q1).*cos(q2).*sin(q3)).*sin(q4).*sin(q6))+(cos(q5).*((-1).*cos(q1).* ...
  cos(q2).*cos(q3)+sin(q1).*sin(q3))+(-1).*cos(q4).*((-1).*cos(q3).*sin( ...
  q1)+(-1).*cos(q1).*cos(q2).*sin(q3)).*sin(q5)).*sin(q7)).*(cos(q7).*( ...
  cos(q6).*(cos(q5).*(cos(q4).*(cos(q1).*cos(q2).*cos(q3)+(-1).*sin(q1).* ...
  sin(q3))+cos(q1).*sin(q2).*sin(q4))+((-1).*cos(q3).*sin(q1)+(-1).*cos( ...
  q1).*cos(q2).*sin(q3)).*sin(q5))+((-1).*cos(q1).*cos(q4).*sin(q2)+(cos( ...
  q1).*cos(q2).*cos(q3)+(-1).*sin(q1).*sin(q3)).*sin(q4)).*sin(q6))+(cos( ...
  q5).*((-1).*cos(q3).*sin(q1)+(-1).*cos(q1).*cos(q2).*sin(q3))+(-1).*( ...
  cos(q4).*(cos(q1).*cos(q2).*cos(q3)+(-1).*sin(q1).*sin(q3))+cos(q1).* ...
  sin(q2).*sin(q4)).*sin(q5)).*sin(q7)).^(-3).*(cos(q7).*(cos(q6).*(cos( ...
  q5).*(cos(q4).*(cos(q2).*cos(q3).*sin(q1)+cos(q1).*sin(q3))+sin(q1).* ...
  sin(q2).*sin(q4))+(cos(q1).*cos(q3)+(-1).*cos(q2).*sin(q1).*sin(q3)).* ...
  sin(q5))+((-1).*cos(q4).*sin(q1).*sin(q2)+(cos(q2).*cos(q3).*sin(q1)+ ...
  cos(q1).*sin(q3)).*sin(q4)).*sin(q6))+(cos(q5).*(cos(q1).*cos(q3)+(-1).* ...
  cos(q2).*sin(q1).*sin(q3))+(-1).*(cos(q4).*(cos(q2).*cos(q3).*sin(q1)+ ...
  cos(q1).*sin(q3))+sin(q1).*sin(q2).*sin(q4)).*sin(q5)).*sin(q7)).^2).*( ...
  1+(cos(q7).*(cos(q6).*(cos(q5).*(cos(q4).*(cos(q1).*cos(q2).*cos(q3)+( ...
  -1).*sin(q1).*sin(q3))+cos(q1).*sin(q2).*sin(q4))+((-1).*cos(q3).*sin( ...
  q1)+(-1).*cos(q1).*cos(q2).*sin(q3)).*sin(q5))+((-1).*cos(q1).*cos(q4).* ...
  sin(q2)+(cos(q1).*cos(q2).*cos(q3)+(-1).*sin(q1).*sin(q3)).*sin(q4)).* ...
  sin(q6))+(cos(q5).*((-1).*cos(q3).*sin(q1)+(-1).*cos(q1).*cos(q2).*sin( ...
  q3))+(-1).*(cos(q4).*(cos(q1).*cos(q2).*cos(q3)+(-1).*sin(q1).*sin(q3))+ ...
  cos(q1).*sin(q2).*sin(q4)).*sin(q5)).*sin(q7)).^(-2).*(cos(q7).*(cos(q6) ...
  .*(cos(q5).*(cos(q4).*(cos(q2).*cos(q3).*sin(q1)+cos(q1).*sin(q3))+sin( ...
  q1).*sin(q2).*sin(q4))+(cos(q1).*cos(q3)+(-1).*cos(q2).*sin(q1).*sin(q3) ...
  ).*sin(q5))+((-1).*cos(q4).*sin(q1).*sin(q2)+(cos(q2).*cos(q3).*sin(q1)+ ...
  cos(q1).*sin(q3)).*sin(q4)).*sin(q6))+(cos(q5).*(cos(q1).*cos(q3)+(-1).* ...
  cos(q2).*sin(q1).*sin(q3))+(-1).*(cos(q4).*(cos(q2).*cos(q3).*sin(q1)+ ...
  cos(q1).*sin(q3))+sin(q1).*sin(q2).*sin(q4)).*sin(q5)).*sin(q7)).^2).^( ...
  -2)+((-2).*(cos(q7).*(cos(q6).*(cos(q4).*cos(q5).*((-1).*cos(q3).*sin( ...
  q1)+(-1).*cos(q1).*cos(q2).*sin(q3))+((-1).*cos(q1).*cos(q2).*cos(q3)+ ...
  sin(q1).*sin(q3)).*sin(q5))+((-1).*cos(q3).*sin(q1)+(-1).*cos(q1).*cos( ...
  q2).*sin(q3)).*sin(q4).*sin(q6))+(cos(q5).*((-1).*cos(q1).*cos(q2).*cos( ...
  q3)+sin(q1).*sin(q3))+(-1).*cos(q4).*((-1).*cos(q3).*sin(q1)+(-1).*cos( ...
  q1).*cos(q2).*sin(q3)).*sin(q5)).*sin(q7)).*(cos(q7).*(cos(q6).*(cos(q4) ...
  .*cos(q5).*(cos(q1).*cos(q3)+(-1).*cos(q2).*sin(q1).*sin(q3))+((-1).* ...
  cos(q2).*cos(q3).*sin(q1)+(-1).*cos(q1).*sin(q3)).*sin(q5))+(cos(q1).* ...
  cos(q3)+(-1).*cos(q2).*sin(q1).*sin(q3)).*sin(q4).*sin(q6))+(cos(q5).*(( ...
  -1).*cos(q2).*cos(q3).*sin(q1)+(-1).*cos(q1).*sin(q3))+(-1).*cos(q4).*( ...
  cos(q1).*cos(q3)+(-1).*cos(q2).*sin(q1).*sin(q3)).*sin(q5)).*sin(q7)).*( ...
  cos(q7).*(cos(q6).*(cos(q5).*(cos(q4).*(cos(q1).*cos(q2).*cos(q3)+(-1).* ...
  sin(q1).*sin(q3))+cos(q1).*sin(q2).*sin(q4))+((-1).*cos(q3).*sin(q1)+( ...
  -1).*cos(q1).*cos(q2).*sin(q3)).*sin(q5))+((-1).*cos(q1).*cos(q4).*sin( ...
  q2)+(cos(q1).*cos(q2).*cos(q3)+(-1).*sin(q1).*sin(q3)).*sin(q4)).*sin( ...
  q6))+(cos(q5).*((-1).*cos(q3).*sin(q1)+(-1).*cos(q1).*cos(q2).*sin(q3))+ ...
  (-1).*(cos(q4).*(cos(q1).*cos(q2).*cos(q3)+(-1).*sin(q1).*sin(q3))+cos( ...
  q1).*sin(q2).*sin(q4)).*sin(q5)).*sin(q7)).^(-2)+(cos(q7).*(cos(q6).*( ...
  cos(q4).*cos(q5).*((-1).*cos(q2).*cos(q3).*sin(q1)+(-1).*cos(q1).*sin( ...
  q3))+((-1).*cos(q1).*cos(q3)+cos(q2).*sin(q1).*sin(q3)).*sin(q5))+((-1) ...
  .*cos(q2).*cos(q3).*sin(q1)+(-1).*cos(q1).*sin(q3)).*sin(q4).*sin(q6))+( ...
  cos(q5).*((-1).*cos(q1).*cos(q3)+cos(q2).*sin(q1).*sin(q3))+(-1).*cos( ...
  q4).*((-1).*cos(q2).*cos(q3).*sin(q1)+(-1).*cos(q1).*sin(q3)).*sin(q5)) ...
  .*sin(q7)).*(cos(q7).*(cos(q6).*(cos(q5).*(cos(q4).*(cos(q1).*cos(q2).* ...
  cos(q3)+(-1).*sin(q1).*sin(q3))+cos(q1).*sin(q2).*sin(q4))+((-1).*cos( ...
  q3).*sin(q1)+(-1).*cos(q1).*cos(q2).*sin(q3)).*sin(q5))+((-1).*cos(q1).* ...
  cos(q4).*sin(q2)+(cos(q1).*cos(q2).*cos(q3)+(-1).*sin(q1).*sin(q3)).* ...
  sin(q4)).*sin(q6))+(cos(q5).*((-1).*cos(q3).*sin(q1)+(-1).*cos(q1).*cos( ...
  q2).*sin(q3))+(-1).*(cos(q4).*(cos(q1).*cos(q2).*cos(q3)+(-1).*sin(q1).* ...
  sin(q3))+cos(q1).*sin(q2).*sin(q4)).*sin(q5)).*sin(q7)).^(-1)+2.*(cos( ...
  q7).*(cos(q6).*(cos(q4).*cos(q5).*((-1).*cos(q3).*sin(q1)+(-1).*cos(q1) ...
  .*cos(q2).*sin(q3))+((-1).*cos(q1).*cos(q2).*cos(q3)+sin(q1).*sin(q3)).* ...
  sin(q5))+((-1).*cos(q3).*sin(q1)+(-1).*cos(q1).*cos(q2).*sin(q3)).*sin( ...
  q4).*sin(q6))+(cos(q5).*((-1).*cos(q1).*cos(q2).*cos(q3)+sin(q1).*sin( ...
  q3))+(-1).*cos(q4).*((-1).*cos(q3).*sin(q1)+(-1).*cos(q1).*cos(q2).*sin( ...
  q3)).*sin(q5)).*sin(q7)).^2.*(cos(q7).*(cos(q6).*(cos(q5).*(cos(q4).*( ...
  cos(q1).*cos(q2).*cos(q3)+(-1).*sin(q1).*sin(q3))+cos(q1).*sin(q2).*sin( ...
  q4))+((-1).*cos(q3).*sin(q1)+(-1).*cos(q1).*cos(q2).*sin(q3)).*sin(q5))+ ...
  ((-1).*cos(q1).*cos(q4).*sin(q2)+(cos(q1).*cos(q2).*cos(q3)+(-1).*sin( ...
  q1).*sin(q3)).*sin(q4)).*sin(q6))+(cos(q5).*((-1).*cos(q3).*sin(q1)+(-1) ...
  .*cos(q1).*cos(q2).*sin(q3))+(-1).*(cos(q4).*(cos(q1).*cos(q2).*cos(q3)+ ...
  (-1).*sin(q1).*sin(q3))+cos(q1).*sin(q2).*sin(q4)).*sin(q5)).*sin(q7)) ...
  .^(-3).*(cos(q7).*(cos(q6).*(cos(q5).*(cos(q4).*(cos(q2).*cos(q3).*sin( ...
  q1)+cos(q1).*sin(q3))+sin(q1).*sin(q2).*sin(q4))+(cos(q1).*cos(q3)+(-1) ...
  .*cos(q2).*sin(q1).*sin(q3)).*sin(q5))+((-1).*cos(q4).*sin(q1).*sin(q2)+ ...
  (cos(q2).*cos(q3).*sin(q1)+cos(q1).*sin(q3)).*sin(q4)).*sin(q6))+(cos( ...
  q5).*(cos(q1).*cos(q3)+(-1).*cos(q2).*sin(q1).*sin(q3))+(-1).*(cos(q4).* ...
  (cos(q2).*cos(q3).*sin(q1)+cos(q1).*sin(q3))+sin(q1).*sin(q2).*sin(q4)) ...
  .*sin(q5)).*sin(q7))+(-1).*(cos(q7).*(cos(q6).*(cos(q4).*cos(q5).*((-1) ...
  .*cos(q1).*cos(q2).*cos(q3)+sin(q1).*sin(q3))+(cos(q3).*sin(q1)+cos(q1) ...
  .*cos(q2).*sin(q3)).*sin(q5))+((-1).*cos(q1).*cos(q2).*cos(q3)+sin(q1).* ...
  sin(q3)).*sin(q4).*sin(q6))+(cos(q5).*(cos(q3).*sin(q1)+cos(q1).*cos(q2) ...
  .*sin(q3))+(-1).*cos(q4).*((-1).*cos(q1).*cos(q2).*cos(q3)+sin(q1).*sin( ...
  q3)).*sin(q5)).*sin(q7)).*(cos(q7).*(cos(q6).*(cos(q5).*(cos(q4).*(cos( ...
  q1).*cos(q2).*cos(q3)+(-1).*sin(q1).*sin(q3))+cos(q1).*sin(q2).*sin(q4)) ...
  +((-1).*cos(q3).*sin(q1)+(-1).*cos(q1).*cos(q2).*sin(q3)).*sin(q5))+(( ...
  -1).*cos(q1).*cos(q4).*sin(q2)+(cos(q1).*cos(q2).*cos(q3)+(-1).*sin(q1) ...
  .*sin(q3)).*sin(q4)).*sin(q6))+(cos(q5).*((-1).*cos(q3).*sin(q1)+(-1).* ...
  cos(q1).*cos(q2).*sin(q3))+(-1).*(cos(q4).*(cos(q1).*cos(q2).*cos(q3)+( ...
  -1).*sin(q1).*sin(q3))+cos(q1).*sin(q2).*sin(q4)).*sin(q5)).*sin(q7)).^( ...
  -2).*(cos(q7).*(cos(q6).*(cos(q5).*(cos(q4).*(cos(q2).*cos(q3).*sin(q1)+ ...
  cos(q1).*sin(q3))+sin(q1).*sin(q2).*sin(q4))+(cos(q1).*cos(q3)+(-1).* ...
  cos(q2).*sin(q1).*sin(q3)).*sin(q5))+((-1).*cos(q4).*sin(q1).*sin(q2)+( ...
  cos(q2).*cos(q3).*sin(q1)+cos(q1).*sin(q3)).*sin(q4)).*sin(q6))+(cos(q5) ...
  .*(cos(q1).*cos(q3)+(-1).*cos(q2).*sin(q1).*sin(q3))+(-1).*(cos(q4).*( ...
  cos(q2).*cos(q3).*sin(q1)+cos(q1).*sin(q3))+sin(q1).*sin(q2).*sin(q4)).* ...
  sin(q5)).*sin(q7))).*(1+(cos(q7).*(cos(q6).*(cos(q5).*(cos(q4).*(cos(q1) ...
  .*cos(q2).*cos(q3)+(-1).*sin(q1).*sin(q3))+cos(q1).*sin(q2).*sin(q4))+(( ...
  -1).*cos(q3).*sin(q1)+(-1).*cos(q1).*cos(q2).*sin(q3)).*sin(q5))+((-1).* ...
  cos(q1).*cos(q4).*sin(q2)+(cos(q1).*cos(q2).*cos(q3)+(-1).*sin(q1).*sin( ...
  q3)).*sin(q4)).*sin(q6))+(cos(q5).*((-1).*cos(q3).*sin(q1)+(-1).*cos(q1) ...
  .*cos(q2).*sin(q3))+(-1).*(cos(q4).*(cos(q1).*cos(q2).*cos(q3)+(-1).* ...
  sin(q1).*sin(q3))+cos(q1).*sin(q2).*sin(q4)).*sin(q5)).*sin(q7)).^(-2).* ...
  (cos(q7).*(cos(q6).*(cos(q5).*(cos(q4).*(cos(q2).*cos(q3).*sin(q1)+cos( ...
  q1).*sin(q3))+sin(q1).*sin(q2).*sin(q4))+(cos(q1).*cos(q3)+(-1).*cos(q2) ...
  .*sin(q1).*sin(q3)).*sin(q5))+((-1).*cos(q4).*sin(q1).*sin(q2)+(cos(q2) ...
  .*cos(q3).*sin(q1)+cos(q1).*sin(q3)).*sin(q4)).*sin(q6))+(cos(q5).*(cos( ...
  q1).*cos(q3)+(-1).*cos(q2).*sin(q1).*sin(q3))+(-1).*(cos(q4).*(cos(q2).* ...
  cos(q3).*sin(q1)+cos(q1).*sin(q3))+sin(q1).*sin(q2).*sin(q4)).*sin(q5)) ...
  .*sin(q7)).^2).^(-1);

Jxe244 = (-1).*((cos(q7).*(cos(q5).*cos(q6).*(cos(q4).*sin( ...
  q1).*sin(q2)+(-1).*(cos(q2).*cos(q3).*sin(q1)+cos(q1).*sin(q3)).*sin(q4) ...
  )+(cos(q4).*(cos(q2).*cos(q3).*sin(q1)+cos(q1).*sin(q3))+sin(q1).*sin( ...
  q2).*sin(q4)).*sin(q6))+(-1).*(cos(q4).*sin(q1).*sin(q2)+(-1).*(cos(q2) ...
  .*cos(q3).*sin(q1)+cos(q1).*sin(q3)).*sin(q4)).*sin(q5).*sin(q7)).*(cos( ...
  q7).*(cos(q6).*(cos(q5).*(cos(q4).*(cos(q1).*cos(q2).*cos(q3)+(-1).*sin( ...
  q1).*sin(q3))+cos(q1).*sin(q2).*sin(q4))+((-1).*cos(q3).*sin(q1)+(-1).* ...
  cos(q1).*cos(q2).*sin(q3)).*sin(q5))+((-1).*cos(q1).*cos(q4).*sin(q2)+( ...
  cos(q1).*cos(q2).*cos(q3)+(-1).*sin(q1).*sin(q3)).*sin(q4)).*sin(q6))+( ...
  cos(q5).*((-1).*cos(q3).*sin(q1)+(-1).*cos(q1).*cos(q2).*sin(q3))+(-1).* ...
  (cos(q4).*(cos(q1).*cos(q2).*cos(q3)+(-1).*sin(q1).*sin(q3))+cos(q1).* ...
  sin(q2).*sin(q4)).*sin(q5)).*sin(q7)).^(-1)+(-1).*(cos(q7).*(cos(q5).* ...
  cos(q6).*(cos(q1).*cos(q4).*sin(q2)+(-1).*(cos(q1).*cos(q2).*cos(q3)+( ...
  -1).*sin(q1).*sin(q3)).*sin(q4))+(cos(q4).*(cos(q1).*cos(q2).*cos(q3)+( ...
  -1).*sin(q1).*sin(q3))+cos(q1).*sin(q2).*sin(q4)).*sin(q6))+(-1).*(cos( ...
  q1).*cos(q4).*sin(q2)+(-1).*(cos(q1).*cos(q2).*cos(q3)+(-1).*sin(q1).* ...
  sin(q3)).*sin(q4)).*sin(q5).*sin(q7)).*(cos(q7).*(cos(q6).*(cos(q5).*( ...
  cos(q4).*(cos(q1).*cos(q2).*cos(q3)+(-1).*sin(q1).*sin(q3))+cos(q1).* ...
  sin(q2).*sin(q4))+((-1).*cos(q3).*sin(q1)+(-1).*cos(q1).*cos(q2).*sin( ...
  q3)).*sin(q5))+((-1).*cos(q1).*cos(q4).*sin(q2)+(cos(q1).*cos(q2).*cos( ...
  q3)+(-1).*sin(q1).*sin(q3)).*sin(q4)).*sin(q6))+(cos(q5).*((-1).*cos(q3) ...
  .*sin(q1)+(-1).*cos(q1).*cos(q2).*sin(q3))+(-1).*(cos(q4).*(cos(q1).* ...
  cos(q2).*cos(q3)+(-1).*sin(q1).*sin(q3))+cos(q1).*sin(q2).*sin(q4)).* ...
  sin(q5)).*sin(q7)).^(-2).*(cos(q7).*(cos(q6).*(cos(q5).*(cos(q4).*(cos( ...
  q2).*cos(q3).*sin(q1)+cos(q1).*sin(q3))+sin(q1).*sin(q2).*sin(q4))+(cos( ...
  q1).*cos(q3)+(-1).*cos(q2).*sin(q1).*sin(q3)).*sin(q5))+((-1).*cos(q4).* ...
  sin(q1).*sin(q2)+(cos(q2).*cos(q3).*sin(q1)+cos(q1).*sin(q3)).*sin(q4)) ...
  .*sin(q6))+(cos(q5).*(cos(q1).*cos(q3)+(-1).*cos(q2).*sin(q1).*sin(q3))+ ...
  (-1).*(cos(q4).*(cos(q2).*cos(q3).*sin(q1)+cos(q1).*sin(q3))+sin(q1).* ...
  sin(q2).*sin(q4)).*sin(q5)).*sin(q7))).*(2.*(cos(q7).*(cos(q5).*cos(q6) ...
  .*(cos(q4).*sin(q1).*sin(q2)+(-1).*(cos(q2).*cos(q3).*sin(q1)+cos(q1).* ...
  sin(q3)).*sin(q4))+(cos(q4).*(cos(q2).*cos(q3).*sin(q1)+cos(q1).*sin(q3) ...
  )+sin(q1).*sin(q2).*sin(q4)).*sin(q6))+(-1).*(cos(q4).*sin(q1).*sin(q2)+ ...
  (-1).*(cos(q2).*cos(q3).*sin(q1)+cos(q1).*sin(q3)).*sin(q4)).*sin(q5).* ...
  sin(q7)).*(cos(q7).*(cos(q6).*(cos(q5).*(cos(q4).*(cos(q1).*cos(q2).* ...
  cos(q3)+(-1).*sin(q1).*sin(q3))+cos(q1).*sin(q2).*sin(q4))+((-1).*cos( ...
  q3).*sin(q1)+(-1).*cos(q1).*cos(q2).*sin(q3)).*sin(q5))+((-1).*cos(q1).* ...
  cos(q4).*sin(q2)+(cos(q1).*cos(q2).*cos(q3)+(-1).*sin(q1).*sin(q3)).* ...
  sin(q4)).*sin(q6))+(cos(q5).*((-1).*cos(q3).*sin(q1)+(-1).*cos(q1).*cos( ...
  q2).*sin(q3))+(-1).*(cos(q4).*(cos(q1).*cos(q2).*cos(q3)+(-1).*sin(q1).* ...
  sin(q3))+cos(q1).*sin(q2).*sin(q4)).*sin(q5)).*sin(q7)).^(-2).*(cos(q7) ...
  .*(cos(q6).*(cos(q5).*(cos(q4).*(cos(q2).*cos(q3).*sin(q1)+cos(q1).*sin( ...
  q3))+sin(q1).*sin(q2).*sin(q4))+(cos(q1).*cos(q3)+(-1).*cos(q2).*sin(q1) ...
  .*sin(q3)).*sin(q5))+((-1).*cos(q4).*sin(q1).*sin(q2)+(cos(q2).*cos(q3) ...
  .*sin(q1)+cos(q1).*sin(q3)).*sin(q4)).*sin(q6))+(cos(q5).*(cos(q1).*cos( ...
  q3)+(-1).*cos(q2).*sin(q1).*sin(q3))+(-1).*(cos(q4).*(cos(q2).*cos(q3).* ...
  sin(q1)+cos(q1).*sin(q3))+sin(q1).*sin(q2).*sin(q4)).*sin(q5)).*sin(q7)) ...
  +(-2).*(cos(q7).*(cos(q5).*cos(q6).*(cos(q1).*cos(q4).*sin(q2)+(-1).*( ...
  cos(q1).*cos(q2).*cos(q3)+(-1).*sin(q1).*sin(q3)).*sin(q4))+(cos(q4).*( ...
  cos(q1).*cos(q2).*cos(q3)+(-1).*sin(q1).*sin(q3))+cos(q1).*sin(q2).*sin( ...
  q4)).*sin(q6))+(-1).*(cos(q1).*cos(q4).*sin(q2)+(-1).*(cos(q1).*cos(q2) ...
  .*cos(q3)+(-1).*sin(q1).*sin(q3)).*sin(q4)).*sin(q5).*sin(q7)).*(cos(q7) ...
  .*(cos(q6).*(cos(q5).*(cos(q4).*(cos(q1).*cos(q2).*cos(q3)+(-1).*sin(q1) ...
  .*sin(q3))+cos(q1).*sin(q2).*sin(q4))+((-1).*cos(q3).*sin(q1)+(-1).*cos( ...
  q1).*cos(q2).*sin(q3)).*sin(q5))+((-1).*cos(q1).*cos(q4).*sin(q2)+(cos( ...
  q1).*cos(q2).*cos(q3)+(-1).*sin(q1).*sin(q3)).*sin(q4)).*sin(q6))+(cos( ...
  q5).*((-1).*cos(q3).*sin(q1)+(-1).*cos(q1).*cos(q2).*sin(q3))+(-1).*( ...
  cos(q4).*(cos(q1).*cos(q2).*cos(q3)+(-1).*sin(q1).*sin(q3))+cos(q1).* ...
  sin(q2).*sin(q4)).*sin(q5)).*sin(q7)).^(-3).*(cos(q7).*(cos(q6).*(cos( ...
  q5).*(cos(q4).*(cos(q2).*cos(q3).*sin(q1)+cos(q1).*sin(q3))+sin(q1).* ...
  sin(q2).*sin(q4))+(cos(q1).*cos(q3)+(-1).*cos(q2).*sin(q1).*sin(q3)).* ...
  sin(q5))+((-1).*cos(q4).*sin(q1).*sin(q2)+(cos(q2).*cos(q3).*sin(q1)+ ...
  cos(q1).*sin(q3)).*sin(q4)).*sin(q6))+(cos(q5).*(cos(q1).*cos(q3)+(-1).* ...
  cos(q2).*sin(q1).*sin(q3))+(-1).*(cos(q4).*(cos(q2).*cos(q3).*sin(q1)+ ...
  cos(q1).*sin(q3))+sin(q1).*sin(q2).*sin(q4)).*sin(q5)).*sin(q7)).^2).*( ...
  1+(cos(q7).*(cos(q6).*(cos(q5).*(cos(q4).*(cos(q1).*cos(q2).*cos(q3)+( ...
  -1).*sin(q1).*sin(q3))+cos(q1).*sin(q2).*sin(q4))+((-1).*cos(q3).*sin( ...
  q1)+(-1).*cos(q1).*cos(q2).*sin(q3)).*sin(q5))+((-1).*cos(q1).*cos(q4).* ...
  sin(q2)+(cos(q1).*cos(q2).*cos(q3)+(-1).*sin(q1).*sin(q3)).*sin(q4)).* ...
  sin(q6))+(cos(q5).*((-1).*cos(q3).*sin(q1)+(-1).*cos(q1).*cos(q2).*sin( ...
  q3))+(-1).*(cos(q4).*(cos(q1).*cos(q2).*cos(q3)+(-1).*sin(q1).*sin(q3))+ ...
  cos(q1).*sin(q2).*sin(q4)).*sin(q5)).*sin(q7)).^(-2).*(cos(q7).*(cos(q6) ...
  .*(cos(q5).*(cos(q4).*(cos(q2).*cos(q3).*sin(q1)+cos(q1).*sin(q3))+sin( ...
  q1).*sin(q2).*sin(q4))+(cos(q1).*cos(q3)+(-1).*cos(q2).*sin(q1).*sin(q3) ...
  ).*sin(q5))+((-1).*cos(q4).*sin(q1).*sin(q2)+(cos(q2).*cos(q3).*sin(q1)+ ...
  cos(q1).*sin(q3)).*sin(q4)).*sin(q6))+(cos(q5).*(cos(q1).*cos(q3)+(-1).* ...
  cos(q2).*sin(q1).*sin(q3))+(-1).*(cos(q4).*(cos(q2).*cos(q3).*sin(q1)+ ...
  cos(q1).*sin(q3))+sin(q1).*sin(q2).*sin(q4)).*sin(q5)).*sin(q7)).^2).^( ...
  -2)+((-2).*(cos(q7).*(cos(q5).*cos(q6).*(cos(q4).*sin(q1).*sin(q2)+(-1) ...
  .*(cos(q2).*cos(q3).*sin(q1)+cos(q1).*sin(q3)).*sin(q4))+(cos(q4).*(cos( ...
  q2).*cos(q3).*sin(q1)+cos(q1).*sin(q3))+sin(q1).*sin(q2).*sin(q4)).*sin( ...
  q6))+(-1).*(cos(q4).*sin(q1).*sin(q2)+(-1).*(cos(q2).*cos(q3).*sin(q1)+ ...
  cos(q1).*sin(q3)).*sin(q4)).*sin(q5).*sin(q7)).*(cos(q7).*(cos(q5).*cos( ...
  q6).*(cos(q1).*cos(q4).*sin(q2)+(-1).*(cos(q1).*cos(q2).*cos(q3)+(-1).* ...
  sin(q1).*sin(q3)).*sin(q4))+(cos(q4).*(cos(q1).*cos(q2).*cos(q3)+(-1).* ...
  sin(q1).*sin(q3))+cos(q1).*sin(q2).*sin(q4)).*sin(q6))+(-1).*(cos(q1).* ...
  cos(q4).*sin(q2)+(-1).*(cos(q1).*cos(q2).*cos(q3)+(-1).*sin(q1).*sin(q3) ...
  ).*sin(q4)).*sin(q5).*sin(q7)).*(cos(q7).*(cos(q6).*(cos(q5).*(cos(q4).* ...
  (cos(q1).*cos(q2).*cos(q3)+(-1).*sin(q1).*sin(q3))+cos(q1).*sin(q2).* ...
  sin(q4))+((-1).*cos(q3).*sin(q1)+(-1).*cos(q1).*cos(q2).*sin(q3)).*sin( ...
  q5))+((-1).*cos(q1).*cos(q4).*sin(q2)+(cos(q1).*cos(q2).*cos(q3)+(-1).* ...
  sin(q1).*sin(q3)).*sin(q4)).*sin(q6))+(cos(q5).*((-1).*cos(q3).*sin(q1)+ ...
  (-1).*cos(q1).*cos(q2).*sin(q3))+(-1).*(cos(q4).*(cos(q1).*cos(q2).*cos( ...
  q3)+(-1).*sin(q1).*sin(q3))+cos(q1).*sin(q2).*sin(q4)).*sin(q5)).*sin( ...
  q7)).^(-2)+(cos(q7).*(cos(q5).*cos(q6).*((-1).*cos(q4).*(cos(q2).*cos( ...
  q3).*sin(q1)+cos(q1).*sin(q3))+(-1).*sin(q1).*sin(q2).*sin(q4))+(cos(q4) ...
  .*sin(q1).*sin(q2)+(-1).*(cos(q2).*cos(q3).*sin(q1)+cos(q1).*sin(q3)).* ...
  sin(q4)).*sin(q6))+(-1).*((-1).*cos(q4).*(cos(q2).*cos(q3).*sin(q1)+cos( ...
  q1).*sin(q3))+(-1).*sin(q1).*sin(q2).*sin(q4)).*sin(q5).*sin(q7)).*(cos( ...
  q7).*(cos(q6).*(cos(q5).*(cos(q4).*(cos(q1).*cos(q2).*cos(q3)+(-1).*sin( ...
  q1).*sin(q3))+cos(q1).*sin(q2).*sin(q4))+((-1).*cos(q3).*sin(q1)+(-1).* ...
  cos(q1).*cos(q2).*sin(q3)).*sin(q5))+((-1).*cos(q1).*cos(q4).*sin(q2)+( ...
  cos(q1).*cos(q2).*cos(q3)+(-1).*sin(q1).*sin(q3)).*sin(q4)).*sin(q6))+( ...
  cos(q5).*((-1).*cos(q3).*sin(q1)+(-1).*cos(q1).*cos(q2).*sin(q3))+(-1).* ...
  (cos(q4).*(cos(q1).*cos(q2).*cos(q3)+(-1).*sin(q1).*sin(q3))+cos(q1).* ...
  sin(q2).*sin(q4)).*sin(q5)).*sin(q7)).^(-1)+2.*(cos(q7).*(cos(q5).*cos( ...
  q6).*(cos(q1).*cos(q4).*sin(q2)+(-1).*(cos(q1).*cos(q2).*cos(q3)+(-1).* ...
  sin(q1).*sin(q3)).*sin(q4))+(cos(q4).*(cos(q1).*cos(q2).*cos(q3)+(-1).* ...
  sin(q1).*sin(q3))+cos(q1).*sin(q2).*sin(q4)).*sin(q6))+(-1).*(cos(q1).* ...
  cos(q4).*sin(q2)+(-1).*(cos(q1).*cos(q2).*cos(q3)+(-1).*sin(q1).*sin(q3) ...
  ).*sin(q4)).*sin(q5).*sin(q7)).^2.*(cos(q7).*(cos(q6).*(cos(q5).*(cos( ...
  q4).*(cos(q1).*cos(q2).*cos(q3)+(-1).*sin(q1).*sin(q3))+cos(q1).*sin(q2) ...
  .*sin(q4))+((-1).*cos(q3).*sin(q1)+(-1).*cos(q1).*cos(q2).*sin(q3)).* ...
  sin(q5))+((-1).*cos(q1).*cos(q4).*sin(q2)+(cos(q1).*cos(q2).*cos(q3)+( ...
  -1).*sin(q1).*sin(q3)).*sin(q4)).*sin(q6))+(cos(q5).*((-1).*cos(q3).* ...
  sin(q1)+(-1).*cos(q1).*cos(q2).*sin(q3))+(-1).*(cos(q4).*(cos(q1).*cos( ...
  q2).*cos(q3)+(-1).*sin(q1).*sin(q3))+cos(q1).*sin(q2).*sin(q4)).*sin(q5) ...
  ).*sin(q7)).^(-3).*(cos(q7).*(cos(q6).*(cos(q5).*(cos(q4).*(cos(q2).* ...
  cos(q3).*sin(q1)+cos(q1).*sin(q3))+sin(q1).*sin(q2).*sin(q4))+(cos(q1).* ...
  cos(q3)+(-1).*cos(q2).*sin(q1).*sin(q3)).*sin(q5))+((-1).*cos(q4).*sin( ...
  q1).*sin(q2)+(cos(q2).*cos(q3).*sin(q1)+cos(q1).*sin(q3)).*sin(q4)).* ...
  sin(q6))+(cos(q5).*(cos(q1).*cos(q3)+(-1).*cos(q2).*sin(q1).*sin(q3))+( ...
  -1).*(cos(q4).*(cos(q2).*cos(q3).*sin(q1)+cos(q1).*sin(q3))+sin(q1).* ...
  sin(q2).*sin(q4)).*sin(q5)).*sin(q7))+(-1).*(cos(q7).*(cos(q5).*cos(q6) ...
  .*((-1).*cos(q4).*(cos(q1).*cos(q2).*cos(q3)+(-1).*sin(q1).*sin(q3))+( ...
  -1).*cos(q1).*sin(q2).*sin(q4))+(cos(q1).*cos(q4).*sin(q2)+(-1).*(cos( ...
  q1).*cos(q2).*cos(q3)+(-1).*sin(q1).*sin(q3)).*sin(q4)).*sin(q6))+(-1).* ...
  ((-1).*cos(q4).*(cos(q1).*cos(q2).*cos(q3)+(-1).*sin(q1).*sin(q3))+(-1) ...
  .*cos(q1).*sin(q2).*sin(q4)).*sin(q5).*sin(q7)).*(cos(q7).*(cos(q6).*( ...
  cos(q5).*(cos(q4).*(cos(q1).*cos(q2).*cos(q3)+(-1).*sin(q1).*sin(q3))+ ...
  cos(q1).*sin(q2).*sin(q4))+((-1).*cos(q3).*sin(q1)+(-1).*cos(q1).*cos( ...
  q2).*sin(q3)).*sin(q5))+((-1).*cos(q1).*cos(q4).*sin(q2)+(cos(q1).*cos( ...
  q2).*cos(q3)+(-1).*sin(q1).*sin(q3)).*sin(q4)).*sin(q6))+(cos(q5).*((-1) ...
  .*cos(q3).*sin(q1)+(-1).*cos(q1).*cos(q2).*sin(q3))+(-1).*(cos(q4).*( ...
  cos(q1).*cos(q2).*cos(q3)+(-1).*sin(q1).*sin(q3))+cos(q1).*sin(q2).*sin( ...
  q4)).*sin(q5)).*sin(q7)).^(-2).*(cos(q7).*(cos(q6).*(cos(q5).*(cos(q4).* ...
  (cos(q2).*cos(q3).*sin(q1)+cos(q1).*sin(q3))+sin(q1).*sin(q2).*sin(q4))+ ...
  (cos(q1).*cos(q3)+(-1).*cos(q2).*sin(q1).*sin(q3)).*sin(q5))+((-1).*cos( ...
  q4).*sin(q1).*sin(q2)+(cos(q2).*cos(q3).*sin(q1)+cos(q1).*sin(q3)).*sin( ...
  q4)).*sin(q6))+(cos(q5).*(cos(q1).*cos(q3)+(-1).*cos(q2).*sin(q1).*sin( ...
  q3))+(-1).*(cos(q4).*(cos(q2).*cos(q3).*sin(q1)+cos(q1).*sin(q3))+sin( ...
  q1).*sin(q2).*sin(q4)).*sin(q5)).*sin(q7))).*(1+(cos(q7).*(cos(q6).*( ...
  cos(q5).*(cos(q4).*(cos(q1).*cos(q2).*cos(q3)+(-1).*sin(q1).*sin(q3))+ ...
  cos(q1).*sin(q2).*sin(q4))+((-1).*cos(q3).*sin(q1)+(-1).*cos(q1).*cos( ...
  q2).*sin(q3)).*sin(q5))+((-1).*cos(q1).*cos(q4).*sin(q2)+(cos(q1).*cos( ...
  q2).*cos(q3)+(-1).*sin(q1).*sin(q3)).*sin(q4)).*sin(q6))+(cos(q5).*((-1) ...
  .*cos(q3).*sin(q1)+(-1).*cos(q1).*cos(q2).*sin(q3))+(-1).*(cos(q4).*( ...
  cos(q1).*cos(q2).*cos(q3)+(-1).*sin(q1).*sin(q3))+cos(q1).*sin(q2).*sin( ...
  q4)).*sin(q5)).*sin(q7)).^(-2).*(cos(q7).*(cos(q6).*(cos(q5).*(cos(q4).* ...
  (cos(q2).*cos(q3).*sin(q1)+cos(q1).*sin(q3))+sin(q1).*sin(q2).*sin(q4))+ ...
  (cos(q1).*cos(q3)+(-1).*cos(q2).*sin(q1).*sin(q3)).*sin(q5))+((-1).*cos( ...
  q4).*sin(q1).*sin(q2)+(cos(q2).*cos(q3).*sin(q1)+cos(q1).*sin(q3)).*sin( ...
  q4)).*sin(q6))+(cos(q5).*(cos(q1).*cos(q3)+(-1).*cos(q2).*sin(q1).*sin( ...
  q3))+(-1).*(cos(q4).*(cos(q2).*cos(q3).*sin(q1)+cos(q1).*sin(q3))+sin( ...
  q1).*sin(q2).*sin(q4)).*sin(q5)).*sin(q7)).^2).^(-1);

Jxe245 = (-1).*((cos(q6).* ...
  cos(q7).*(cos(q5).*(cos(q1).*cos(q3)+(-1).*cos(q2).*sin(q1).*sin(q3))+( ...
  -1).*(cos(q4).*(cos(q2).*cos(q3).*sin(q1)+cos(q1).*sin(q3))+sin(q1).* ...
  sin(q2).*sin(q4)).*sin(q5))+((-1).*cos(q5).*(cos(q4).*(cos(q2).*cos(q3) ...
  .*sin(q1)+cos(q1).*sin(q3))+sin(q1).*sin(q2).*sin(q4))+(-1).*(cos(q1).* ...
  cos(q3)+(-1).*cos(q2).*sin(q1).*sin(q3)).*sin(q5)).*sin(q7)).*(cos(q7).* ...
  (cos(q6).*(cos(q5).*(cos(q4).*(cos(q1).*cos(q2).*cos(q3)+(-1).*sin(q1).* ...
  sin(q3))+cos(q1).*sin(q2).*sin(q4))+((-1).*cos(q3).*sin(q1)+(-1).*cos( ...
  q1).*cos(q2).*sin(q3)).*sin(q5))+((-1).*cos(q1).*cos(q4).*sin(q2)+(cos( ...
  q1).*cos(q2).*cos(q3)+(-1).*sin(q1).*sin(q3)).*sin(q4)).*sin(q6))+(cos( ...
  q5).*((-1).*cos(q3).*sin(q1)+(-1).*cos(q1).*cos(q2).*sin(q3))+(-1).*( ...
  cos(q4).*(cos(q1).*cos(q2).*cos(q3)+(-1).*sin(q1).*sin(q3))+cos(q1).* ...
  sin(q2).*sin(q4)).*sin(q5)).*sin(q7)).^(-1)+(-1).*(cos(q6).*cos(q7).*( ...
  cos(q5).*((-1).*cos(q3).*sin(q1)+(-1).*cos(q1).*cos(q2).*sin(q3))+(-1).* ...
  (cos(q4).*(cos(q1).*cos(q2).*cos(q3)+(-1).*sin(q1).*sin(q3))+cos(q1).* ...
  sin(q2).*sin(q4)).*sin(q5))+((-1).*cos(q5).*(cos(q4).*(cos(q1).*cos(q2) ...
  .*cos(q3)+(-1).*sin(q1).*sin(q3))+cos(q1).*sin(q2).*sin(q4))+(-1).*((-1) ...
  .*cos(q3).*sin(q1)+(-1).*cos(q1).*cos(q2).*sin(q3)).*sin(q5)).*sin(q7)) ...
  .*(cos(q7).*(cos(q6).*(cos(q5).*(cos(q4).*(cos(q1).*cos(q2).*cos(q3)+( ...
  -1).*sin(q1).*sin(q3))+cos(q1).*sin(q2).*sin(q4))+((-1).*cos(q3).*sin( ...
  q1)+(-1).*cos(q1).*cos(q2).*sin(q3)).*sin(q5))+((-1).*cos(q1).*cos(q4).* ...
  sin(q2)+(cos(q1).*cos(q2).*cos(q3)+(-1).*sin(q1).*sin(q3)).*sin(q4)).* ...
  sin(q6))+(cos(q5).*((-1).*cos(q3).*sin(q1)+(-1).*cos(q1).*cos(q2).*sin( ...
  q3))+(-1).*(cos(q4).*(cos(q1).*cos(q2).*cos(q3)+(-1).*sin(q1).*sin(q3))+ ...
  cos(q1).*sin(q2).*sin(q4)).*sin(q5)).*sin(q7)).^(-2).*(cos(q7).*(cos(q6) ...
  .*(cos(q5).*(cos(q4).*(cos(q2).*cos(q3).*sin(q1)+cos(q1).*sin(q3))+sin( ...
  q1).*sin(q2).*sin(q4))+(cos(q1).*cos(q3)+(-1).*cos(q2).*sin(q1).*sin(q3) ...
  ).*sin(q5))+((-1).*cos(q4).*sin(q1).*sin(q2)+(cos(q2).*cos(q3).*sin(q1)+ ...
  cos(q1).*sin(q3)).*sin(q4)).*sin(q6))+(cos(q5).*(cos(q1).*cos(q3)+(-1).* ...
  cos(q2).*sin(q1).*sin(q3))+(-1).*(cos(q4).*(cos(q2).*cos(q3).*sin(q1)+ ...
  cos(q1).*sin(q3))+sin(q1).*sin(q2).*sin(q4)).*sin(q5)).*sin(q7))).*(2.*( ...
  cos(q6).*cos(q7).*(cos(q5).*(cos(q1).*cos(q3)+(-1).*cos(q2).*sin(q1).* ...
  sin(q3))+(-1).*(cos(q4).*(cos(q2).*cos(q3).*sin(q1)+cos(q1).*sin(q3))+ ...
  sin(q1).*sin(q2).*sin(q4)).*sin(q5))+((-1).*cos(q5).*(cos(q4).*(cos(q2) ...
  .*cos(q3).*sin(q1)+cos(q1).*sin(q3))+sin(q1).*sin(q2).*sin(q4))+(-1).*( ...
  cos(q1).*cos(q3)+(-1).*cos(q2).*sin(q1).*sin(q3)).*sin(q5)).*sin(q7)).*( ...
  cos(q7).*(cos(q6).*(cos(q5).*(cos(q4).*(cos(q1).*cos(q2).*cos(q3)+(-1).* ...
  sin(q1).*sin(q3))+cos(q1).*sin(q2).*sin(q4))+((-1).*cos(q3).*sin(q1)+( ...
  -1).*cos(q1).*cos(q2).*sin(q3)).*sin(q5))+((-1).*cos(q1).*cos(q4).*sin( ...
  q2)+(cos(q1).*cos(q2).*cos(q3)+(-1).*sin(q1).*sin(q3)).*sin(q4)).*sin( ...
  q6))+(cos(q5).*((-1).*cos(q3).*sin(q1)+(-1).*cos(q1).*cos(q2).*sin(q3))+ ...
  (-1).*(cos(q4).*(cos(q1).*cos(q2).*cos(q3)+(-1).*sin(q1).*sin(q3))+cos( ...
  q1).*sin(q2).*sin(q4)).*sin(q5)).*sin(q7)).^(-2).*(cos(q7).*(cos(q6).*( ...
  cos(q5).*(cos(q4).*(cos(q2).*cos(q3).*sin(q1)+cos(q1).*sin(q3))+sin(q1) ...
  .*sin(q2).*sin(q4))+(cos(q1).*cos(q3)+(-1).*cos(q2).*sin(q1).*sin(q3)).* ...
  sin(q5))+((-1).*cos(q4).*sin(q1).*sin(q2)+(cos(q2).*cos(q3).*sin(q1)+ ...
  cos(q1).*sin(q3)).*sin(q4)).*sin(q6))+(cos(q5).*(cos(q1).*cos(q3)+(-1).* ...
  cos(q2).*sin(q1).*sin(q3))+(-1).*(cos(q4).*(cos(q2).*cos(q3).*sin(q1)+ ...
  cos(q1).*sin(q3))+sin(q1).*sin(q2).*sin(q4)).*sin(q5)).*sin(q7))+(-2).*( ...
  cos(q6).*cos(q7).*(cos(q5).*((-1).*cos(q3).*sin(q1)+(-1).*cos(q1).*cos( ...
  q2).*sin(q3))+(-1).*(cos(q4).*(cos(q1).*cos(q2).*cos(q3)+(-1).*sin(q1).* ...
  sin(q3))+cos(q1).*sin(q2).*sin(q4)).*sin(q5))+((-1).*cos(q5).*(cos(q4).* ...
  (cos(q1).*cos(q2).*cos(q3)+(-1).*sin(q1).*sin(q3))+cos(q1).*sin(q2).* ...
  sin(q4))+(-1).*((-1).*cos(q3).*sin(q1)+(-1).*cos(q1).*cos(q2).*sin(q3)) ...
  .*sin(q5)).*sin(q7)).*(cos(q7).*(cos(q6).*(cos(q5).*(cos(q4).*(cos(q1).* ...
  cos(q2).*cos(q3)+(-1).*sin(q1).*sin(q3))+cos(q1).*sin(q2).*sin(q4))+(( ...
  -1).*cos(q3).*sin(q1)+(-1).*cos(q1).*cos(q2).*sin(q3)).*sin(q5))+((-1).* ...
  cos(q1).*cos(q4).*sin(q2)+(cos(q1).*cos(q2).*cos(q3)+(-1).*sin(q1).*sin( ...
  q3)).*sin(q4)).*sin(q6))+(cos(q5).*((-1).*cos(q3).*sin(q1)+(-1).*cos(q1) ...
  .*cos(q2).*sin(q3))+(-1).*(cos(q4).*(cos(q1).*cos(q2).*cos(q3)+(-1).* ...
  sin(q1).*sin(q3))+cos(q1).*sin(q2).*sin(q4)).*sin(q5)).*sin(q7)).^(-3).* ...
  (cos(q7).*(cos(q6).*(cos(q5).*(cos(q4).*(cos(q2).*cos(q3).*sin(q1)+cos( ...
  q1).*sin(q3))+sin(q1).*sin(q2).*sin(q4))+(cos(q1).*cos(q3)+(-1).*cos(q2) ...
  .*sin(q1).*sin(q3)).*sin(q5))+((-1).*cos(q4).*sin(q1).*sin(q2)+(cos(q2) ...
  .*cos(q3).*sin(q1)+cos(q1).*sin(q3)).*sin(q4)).*sin(q6))+(cos(q5).*(cos( ...
  q1).*cos(q3)+(-1).*cos(q2).*sin(q1).*sin(q3))+(-1).*(cos(q4).*(cos(q2).* ...
  cos(q3).*sin(q1)+cos(q1).*sin(q3))+sin(q1).*sin(q2).*sin(q4)).*sin(q5)) ...
  .*sin(q7)).^2).*(1+(cos(q7).*(cos(q6).*(cos(q5).*(cos(q4).*(cos(q1).* ...
  cos(q2).*cos(q3)+(-1).*sin(q1).*sin(q3))+cos(q1).*sin(q2).*sin(q4))+(( ...
  -1).*cos(q3).*sin(q1)+(-1).*cos(q1).*cos(q2).*sin(q3)).*sin(q5))+((-1).* ...
  cos(q1).*cos(q4).*sin(q2)+(cos(q1).*cos(q2).*cos(q3)+(-1).*sin(q1).*sin( ...
  q3)).*sin(q4)).*sin(q6))+(cos(q5).*((-1).*cos(q3).*sin(q1)+(-1).*cos(q1) ...
  .*cos(q2).*sin(q3))+(-1).*(cos(q4).*(cos(q1).*cos(q2).*cos(q3)+(-1).* ...
  sin(q1).*sin(q3))+cos(q1).*sin(q2).*sin(q4)).*sin(q5)).*sin(q7)).^(-2).* ...
  (cos(q7).*(cos(q6).*(cos(q5).*(cos(q4).*(cos(q2).*cos(q3).*sin(q1)+cos( ...
  q1).*sin(q3))+sin(q1).*sin(q2).*sin(q4))+(cos(q1).*cos(q3)+(-1).*cos(q2) ...
  .*sin(q1).*sin(q3)).*sin(q5))+((-1).*cos(q4).*sin(q1).*sin(q2)+(cos(q2) ...
  .*cos(q3).*sin(q1)+cos(q1).*sin(q3)).*sin(q4)).*sin(q6))+(cos(q5).*(cos( ...
  q1).*cos(q3)+(-1).*cos(q2).*sin(q1).*sin(q3))+(-1).*(cos(q4).*(cos(q2).* ...
  cos(q3).*sin(q1)+cos(q1).*sin(q3))+sin(q1).*sin(q2).*sin(q4)).*sin(q5)) ...
  .*sin(q7)).^2).^(-2)+(1+(cos(q7).*(cos(q6).*(cos(q5).*(cos(q4).*(cos(q1) ...
  .*cos(q2).*cos(q3)+(-1).*sin(q1).*sin(q3))+cos(q1).*sin(q2).*sin(q4))+(( ...
  -1).*cos(q3).*sin(q1)+(-1).*cos(q1).*cos(q2).*sin(q3)).*sin(q5))+((-1).* ...
  cos(q1).*cos(q4).*sin(q2)+(cos(q1).*cos(q2).*cos(q3)+(-1).*sin(q1).*sin( ...
  q3)).*sin(q4)).*sin(q6))+(cos(q5).*((-1).*cos(q3).*sin(q1)+(-1).*cos(q1) ...
  .*cos(q2).*sin(q3))+(-1).*(cos(q4).*(cos(q1).*cos(q2).*cos(q3)+(-1).* ...
  sin(q1).*sin(q3))+cos(q1).*sin(q2).*sin(q4)).*sin(q5)).*sin(q7)).^(-2).* ...
  (cos(q7).*(cos(q6).*(cos(q5).*(cos(q4).*(cos(q2).*cos(q3).*sin(q1)+cos( ...
  q1).*sin(q3))+sin(q1).*sin(q2).*sin(q4))+(cos(q1).*cos(q3)+(-1).*cos(q2) ...
  .*sin(q1).*sin(q3)).*sin(q5))+((-1).*cos(q4).*sin(q1).*sin(q2)+(cos(q2) ...
  .*cos(q3).*sin(q1)+cos(q1).*sin(q3)).*sin(q4)).*sin(q6))+(cos(q5).*(cos( ...
  q1).*cos(q3)+(-1).*cos(q2).*sin(q1).*sin(q3))+(-1).*(cos(q4).*(cos(q2).* ...
  cos(q3).*sin(q1)+cos(q1).*sin(q3))+sin(q1).*sin(q2).*sin(q4)).*sin(q5)) ...
  .*sin(q7)).^2).^(-1).*((-2).*(cos(q6).*cos(q7).*(cos(q5).*((-1).*cos(q3) ...
  .*sin(q1)+(-1).*cos(q1).*cos(q2).*sin(q3))+(-1).*(cos(q4).*(cos(q1).* ...
  cos(q2).*cos(q3)+(-1).*sin(q1).*sin(q3))+cos(q1).*sin(q2).*sin(q4)).* ...
  sin(q5))+((-1).*cos(q5).*(cos(q4).*(cos(q1).*cos(q2).*cos(q3)+(-1).*sin( ...
  q1).*sin(q3))+cos(q1).*sin(q2).*sin(q4))+(-1).*((-1).*cos(q3).*sin(q1)+( ...
  -1).*cos(q1).*cos(q2).*sin(q3)).*sin(q5)).*sin(q7)).*(cos(q6).*cos(q7).* ...
  (cos(q5).*(cos(q1).*cos(q3)+(-1).*cos(q2).*sin(q1).*sin(q3))+(-1).*(cos( ...
  q4).*(cos(q2).*cos(q3).*sin(q1)+cos(q1).*sin(q3))+sin(q1).*sin(q2).*sin( ...
  q4)).*sin(q5))+((-1).*cos(q5).*(cos(q4).*(cos(q2).*cos(q3).*sin(q1)+cos( ...
  q1).*sin(q3))+sin(q1).*sin(q2).*sin(q4))+(-1).*(cos(q1).*cos(q3)+(-1).* ...
  cos(q2).*sin(q1).*sin(q3)).*sin(q5)).*sin(q7)).*(cos(q7).*(cos(q6).*( ...
  cos(q5).*(cos(q4).*(cos(q1).*cos(q2).*cos(q3)+(-1).*sin(q1).*sin(q3))+ ...
  cos(q1).*sin(q2).*sin(q4))+((-1).*cos(q3).*sin(q1)+(-1).*cos(q1).*cos( ...
  q2).*sin(q3)).*sin(q5))+((-1).*cos(q1).*cos(q4).*sin(q2)+(cos(q1).*cos( ...
  q2).*cos(q3)+(-1).*sin(q1).*sin(q3)).*sin(q4)).*sin(q6))+(cos(q5).*((-1) ...
  .*cos(q3).*sin(q1)+(-1).*cos(q1).*cos(q2).*sin(q3))+(-1).*(cos(q4).*( ...
  cos(q1).*cos(q2).*cos(q3)+(-1).*sin(q1).*sin(q3))+cos(q1).*sin(q2).*sin( ...
  q4)).*sin(q5)).*sin(q7)).^(-2)+2.*(cos(q6).*cos(q7).*(cos(q5).*((-1).* ...
  cos(q3).*sin(q1)+(-1).*cos(q1).*cos(q2).*sin(q3))+(-1).*(cos(q4).*(cos( ...
  q1).*cos(q2).*cos(q3)+(-1).*sin(q1).*sin(q3))+cos(q1).*sin(q2).*sin(q4)) ...
  .*sin(q5))+((-1).*cos(q5).*(cos(q4).*(cos(q1).*cos(q2).*cos(q3)+(-1).* ...
  sin(q1).*sin(q3))+cos(q1).*sin(q2).*sin(q4))+(-1).*((-1).*cos(q3).*sin( ...
  q1)+(-1).*cos(q1).*cos(q2).*sin(q3)).*sin(q5)).*sin(q7)).^2.*(cos(q7).*( ...
  cos(q6).*(cos(q5).*(cos(q4).*(cos(q1).*cos(q2).*cos(q3)+(-1).*sin(q1).* ...
  sin(q3))+cos(q1).*sin(q2).*sin(q4))+((-1).*cos(q3).*sin(q1)+(-1).*cos( ...
  q1).*cos(q2).*sin(q3)).*sin(q5))+((-1).*cos(q1).*cos(q4).*sin(q2)+(cos( ...
  q1).*cos(q2).*cos(q3)+(-1).*sin(q1).*sin(q3)).*sin(q4)).*sin(q6))+(cos( ...
  q5).*((-1).*cos(q3).*sin(q1)+(-1).*cos(q1).*cos(q2).*sin(q3))+(-1).*( ...
  cos(q4).*(cos(q1).*cos(q2).*cos(q3)+(-1).*sin(q1).*sin(q3))+cos(q1).* ...
  sin(q2).*sin(q4)).*sin(q5)).*sin(q7)).^(-3).*(cos(q7).*(cos(q6).*(cos( ...
  q5).*(cos(q4).*(cos(q2).*cos(q3).*sin(q1)+cos(q1).*sin(q3))+sin(q1).* ...
  sin(q2).*sin(q4))+(cos(q1).*cos(q3)+(-1).*cos(q2).*sin(q1).*sin(q3)).* ...
  sin(q5))+((-1).*cos(q4).*sin(q1).*sin(q2)+(cos(q2).*cos(q3).*sin(q1)+ ...
  cos(q1).*sin(q3)).*sin(q4)).*sin(q6))+(cos(q5).*(cos(q1).*cos(q3)+(-1).* ...
  cos(q2).*sin(q1).*sin(q3))+(-1).*(cos(q4).*(cos(q2).*cos(q3).*sin(q1)+ ...
  cos(q1).*sin(q3))+sin(q1).*sin(q2).*sin(q4)).*sin(q5)).*sin(q7))+(-1).*( ...
  cos(q7).*(cos(q6).*(cos(q5).*(cos(q4).*(cos(q1).*cos(q2).*cos(q3)+(-1).* ...
  sin(q1).*sin(q3))+cos(q1).*sin(q2).*sin(q4))+((-1).*cos(q3).*sin(q1)+( ...
  -1).*cos(q1).*cos(q2).*sin(q3)).*sin(q5))+((-1).*cos(q1).*cos(q4).*sin( ...
  q2)+(cos(q1).*cos(q2).*cos(q3)+(-1).*sin(q1).*sin(q3)).*sin(q4)).*sin( ...
  q6))+(cos(q5).*((-1).*cos(q3).*sin(q1)+(-1).*cos(q1).*cos(q2).*sin(q3))+ ...
  (-1).*(cos(q4).*(cos(q1).*cos(q2).*cos(q3)+(-1).*sin(q1).*sin(q3))+cos( ...
  q1).*sin(q2).*sin(q4)).*sin(q5)).*sin(q7)).^(-2).*(cos(q6).*cos(q7).*(( ...
  -1).*cos(q5).*(cos(q4).*(cos(q1).*cos(q2).*cos(q3)+(-1).*sin(q1).*sin( ...
  q3))+cos(q1).*sin(q2).*sin(q4))+(-1).*((-1).*cos(q3).*sin(q1)+(-1).*cos( ...
  q1).*cos(q2).*sin(q3)).*sin(q5))+((-1).*cos(q5).*((-1).*cos(q3).*sin(q1) ...
  +(-1).*cos(q1).*cos(q2).*sin(q3))+(cos(q4).*(cos(q1).*cos(q2).*cos(q3)+( ...
  -1).*sin(q1).*sin(q3))+cos(q1).*sin(q2).*sin(q4)).*sin(q5)).*sin(q7)).*( ...
  cos(q7).*(cos(q6).*(cos(q5).*(cos(q4).*(cos(q2).*cos(q3).*sin(q1)+cos( ...
  q1).*sin(q3))+sin(q1).*sin(q2).*sin(q4))+(cos(q1).*cos(q3)+(-1).*cos(q2) ...
  .*sin(q1).*sin(q3)).*sin(q5))+((-1).*cos(q4).*sin(q1).*sin(q2)+(cos(q2) ...
  .*cos(q3).*sin(q1)+cos(q1).*sin(q3)).*sin(q4)).*sin(q6))+(cos(q5).*(cos( ...
  q1).*cos(q3)+(-1).*cos(q2).*sin(q1).*sin(q3))+(-1).*(cos(q4).*(cos(q2).* ...
  cos(q3).*sin(q1)+cos(q1).*sin(q3))+sin(q1).*sin(q2).*sin(q4)).*sin(q5)) ...
  .*sin(q7))+(cos(q7).*(cos(q6).*(cos(q5).*(cos(q4).*(cos(q1).*cos(q2).* ...
  cos(q3)+(-1).*sin(q1).*sin(q3))+cos(q1).*sin(q2).*sin(q4))+((-1).*cos( ...
  q3).*sin(q1)+(-1).*cos(q1).*cos(q2).*sin(q3)).*sin(q5))+((-1).*cos(q1).* ...
  cos(q4).*sin(q2)+(cos(q1).*cos(q2).*cos(q3)+(-1).*sin(q1).*sin(q3)).* ...
  sin(q4)).*sin(q6))+(cos(q5).*((-1).*cos(q3).*sin(q1)+(-1).*cos(q1).*cos( ...
  q2).*sin(q3))+(-1).*(cos(q4).*(cos(q1).*cos(q2).*cos(q3)+(-1).*sin(q1).* ...
  sin(q3))+cos(q1).*sin(q2).*sin(q4)).*sin(q5)).*sin(q7)).^(-1).*(cos(q6) ...
  .*cos(q7).*((-1).*cos(q5).*(cos(q4).*(cos(q2).*cos(q3).*sin(q1)+cos(q1) ...
  .*sin(q3))+sin(q1).*sin(q2).*sin(q4))+(-1).*(cos(q1).*cos(q3)+(-1).*cos( ...
  q2).*sin(q1).*sin(q3)).*sin(q5))+((-1).*cos(q5).*(cos(q1).*cos(q3)+(-1) ...
  .*cos(q2).*sin(q1).*sin(q3))+(cos(q4).*(cos(q2).*cos(q3).*sin(q1)+cos( ...
  q1).*sin(q3))+sin(q1).*sin(q2).*sin(q4)).*sin(q5)).*sin(q7)));

Jxe246 = (-1).*( ...
  cos(q7).*(cos(q6).*((-1).*cos(q4).*sin(q1).*sin(q2)+(cos(q2).*cos(q3).* ...
  sin(q1)+cos(q1).*sin(q3)).*sin(q4))+(-1).*(cos(q5).*(cos(q4).*(cos(q2).* ...
  cos(q3).*sin(q1)+cos(q1).*sin(q3))+sin(q1).*sin(q2).*sin(q4))+(cos(q1).* ...
  cos(q3)+(-1).*cos(q2).*sin(q1).*sin(q3)).*sin(q5)).*sin(q6)).*(cos(q7).* ...
  (cos(q6).*(cos(q5).*(cos(q4).*(cos(q1).*cos(q2).*cos(q3)+(-1).*sin(q1).* ...
  sin(q3))+cos(q1).*sin(q2).*sin(q4))+((-1).*cos(q3).*sin(q1)+(-1).*cos( ...
  q1).*cos(q2).*sin(q3)).*sin(q5))+((-1).*cos(q1).*cos(q4).*sin(q2)+(cos( ...
  q1).*cos(q2).*cos(q3)+(-1).*sin(q1).*sin(q3)).*sin(q4)).*sin(q6))+(cos( ...
  q5).*((-1).*cos(q3).*sin(q1)+(-1).*cos(q1).*cos(q2).*sin(q3))+(-1).*( ...
  cos(q4).*(cos(q1).*cos(q2).*cos(q3)+(-1).*sin(q1).*sin(q3))+cos(q1).* ...
  sin(q2).*sin(q4)).*sin(q5)).*sin(q7)).^(-1)+(-1).*cos(q7).*(cos(q6).*(( ...
  -1).*cos(q1).*cos(q4).*sin(q2)+(cos(q1).*cos(q2).*cos(q3)+(-1).*sin(q1) ...
  .*sin(q3)).*sin(q4))+(-1).*(cos(q5).*(cos(q4).*(cos(q1).*cos(q2).*cos( ...
  q3)+(-1).*sin(q1).*sin(q3))+cos(q1).*sin(q2).*sin(q4))+((-1).*cos(q3).* ...
  sin(q1)+(-1).*cos(q1).*cos(q2).*sin(q3)).*sin(q5)).*sin(q6)).*(cos(q7).* ...
  (cos(q6).*(cos(q5).*(cos(q4).*(cos(q1).*cos(q2).*cos(q3)+(-1).*sin(q1).* ...
  sin(q3))+cos(q1).*sin(q2).*sin(q4))+((-1).*cos(q3).*sin(q1)+(-1).*cos( ...
  q1).*cos(q2).*sin(q3)).*sin(q5))+((-1).*cos(q1).*cos(q4).*sin(q2)+(cos( ...
  q1).*cos(q2).*cos(q3)+(-1).*sin(q1).*sin(q3)).*sin(q4)).*sin(q6))+(cos( ...
  q5).*((-1).*cos(q3).*sin(q1)+(-1).*cos(q1).*cos(q2).*sin(q3))+(-1).*( ...
  cos(q4).*(cos(q1).*cos(q2).*cos(q3)+(-1).*sin(q1).*sin(q3))+cos(q1).* ...
  sin(q2).*sin(q4)).*sin(q5)).*sin(q7)).^(-2).*(cos(q7).*(cos(q6).*(cos( ...
  q5).*(cos(q4).*(cos(q2).*cos(q3).*sin(q1)+cos(q1).*sin(q3))+sin(q1).* ...
  sin(q2).*sin(q4))+(cos(q1).*cos(q3)+(-1).*cos(q2).*sin(q1).*sin(q3)).* ...
  sin(q5))+((-1).*cos(q4).*sin(q1).*sin(q2)+(cos(q2).*cos(q3).*sin(q1)+ ...
  cos(q1).*sin(q3)).*sin(q4)).*sin(q6))+(cos(q5).*(cos(q1).*cos(q3)+(-1).* ...
  cos(q2).*sin(q1).*sin(q3))+(-1).*(cos(q4).*(cos(q2).*cos(q3).*sin(q1)+ ...
  cos(q1).*sin(q3))+sin(q1).*sin(q2).*sin(q4)).*sin(q5)).*sin(q7))).*(2.* ...
  cos(q7).*(cos(q6).*((-1).*cos(q4).*sin(q1).*sin(q2)+(cos(q2).*cos(q3).* ...
  sin(q1)+cos(q1).*sin(q3)).*sin(q4))+(-1).*(cos(q5).*(cos(q4).*(cos(q2).* ...
  cos(q3).*sin(q1)+cos(q1).*sin(q3))+sin(q1).*sin(q2).*sin(q4))+(cos(q1).* ...
  cos(q3)+(-1).*cos(q2).*sin(q1).*sin(q3)).*sin(q5)).*sin(q6)).*(cos(q7).* ...
  (cos(q6).*(cos(q5).*(cos(q4).*(cos(q1).*cos(q2).*cos(q3)+(-1).*sin(q1).* ...
  sin(q3))+cos(q1).*sin(q2).*sin(q4))+((-1).*cos(q3).*sin(q1)+(-1).*cos( ...
  q1).*cos(q2).*sin(q3)).*sin(q5))+((-1).*cos(q1).*cos(q4).*sin(q2)+(cos( ...
  q1).*cos(q2).*cos(q3)+(-1).*sin(q1).*sin(q3)).*sin(q4)).*sin(q6))+(cos( ...
  q5).*((-1).*cos(q3).*sin(q1)+(-1).*cos(q1).*cos(q2).*sin(q3))+(-1).*( ...
  cos(q4).*(cos(q1).*cos(q2).*cos(q3)+(-1).*sin(q1).*sin(q3))+cos(q1).* ...
  sin(q2).*sin(q4)).*sin(q5)).*sin(q7)).^(-2).*(cos(q7).*(cos(q6).*(cos( ...
  q5).*(cos(q4).*(cos(q2).*cos(q3).*sin(q1)+cos(q1).*sin(q3))+sin(q1).* ...
  sin(q2).*sin(q4))+(cos(q1).*cos(q3)+(-1).*cos(q2).*sin(q1).*sin(q3)).* ...
  sin(q5))+((-1).*cos(q4).*sin(q1).*sin(q2)+(cos(q2).*cos(q3).*sin(q1)+ ...
  cos(q1).*sin(q3)).*sin(q4)).*sin(q6))+(cos(q5).*(cos(q1).*cos(q3)+(-1).* ...
  cos(q2).*sin(q1).*sin(q3))+(-1).*(cos(q4).*(cos(q2).*cos(q3).*sin(q1)+ ...
  cos(q1).*sin(q3))+sin(q1).*sin(q2).*sin(q4)).*sin(q5)).*sin(q7))+(-2).* ...
  cos(q7).*(cos(q6).*((-1).*cos(q1).*cos(q4).*sin(q2)+(cos(q1).*cos(q2).* ...
  cos(q3)+(-1).*sin(q1).*sin(q3)).*sin(q4))+(-1).*(cos(q5).*(cos(q4).*( ...
  cos(q1).*cos(q2).*cos(q3)+(-1).*sin(q1).*sin(q3))+cos(q1).*sin(q2).*sin( ...
  q4))+((-1).*cos(q3).*sin(q1)+(-1).*cos(q1).*cos(q2).*sin(q3)).*sin(q5)) ...
  .*sin(q6)).*(cos(q7).*(cos(q6).*(cos(q5).*(cos(q4).*(cos(q1).*cos(q2).* ...
  cos(q3)+(-1).*sin(q1).*sin(q3))+cos(q1).*sin(q2).*sin(q4))+((-1).*cos( ...
  q3).*sin(q1)+(-1).*cos(q1).*cos(q2).*sin(q3)).*sin(q5))+((-1).*cos(q1).* ...
  cos(q4).*sin(q2)+(cos(q1).*cos(q2).*cos(q3)+(-1).*sin(q1).*sin(q3)).* ...
  sin(q4)).*sin(q6))+(cos(q5).*((-1).*cos(q3).*sin(q1)+(-1).*cos(q1).*cos( ...
  q2).*sin(q3))+(-1).*(cos(q4).*(cos(q1).*cos(q2).*cos(q3)+(-1).*sin(q1).* ...
  sin(q3))+cos(q1).*sin(q2).*sin(q4)).*sin(q5)).*sin(q7)).^(-3).*(cos(q7) ...
  .*(cos(q6).*(cos(q5).*(cos(q4).*(cos(q2).*cos(q3).*sin(q1)+cos(q1).*sin( ...
  q3))+sin(q1).*sin(q2).*sin(q4))+(cos(q1).*cos(q3)+(-1).*cos(q2).*sin(q1) ...
  .*sin(q3)).*sin(q5))+((-1).*cos(q4).*sin(q1).*sin(q2)+(cos(q2).*cos(q3) ...
  .*sin(q1)+cos(q1).*sin(q3)).*sin(q4)).*sin(q6))+(cos(q5).*(cos(q1).*cos( ...
  q3)+(-1).*cos(q2).*sin(q1).*sin(q3))+(-1).*(cos(q4).*(cos(q2).*cos(q3).* ...
  sin(q1)+cos(q1).*sin(q3))+sin(q1).*sin(q2).*sin(q4)).*sin(q5)).*sin(q7)) ...
  .^2).*(1+(cos(q7).*(cos(q6).*(cos(q5).*(cos(q4).*(cos(q1).*cos(q2).*cos( ...
  q3)+(-1).*sin(q1).*sin(q3))+cos(q1).*sin(q2).*sin(q4))+((-1).*cos(q3).* ...
  sin(q1)+(-1).*cos(q1).*cos(q2).*sin(q3)).*sin(q5))+((-1).*cos(q1).*cos( ...
  q4).*sin(q2)+(cos(q1).*cos(q2).*cos(q3)+(-1).*sin(q1).*sin(q3)).*sin(q4) ...
  ).*sin(q6))+(cos(q5).*((-1).*cos(q3).*sin(q1)+(-1).*cos(q1).*cos(q2).* ...
  sin(q3))+(-1).*(cos(q4).*(cos(q1).*cos(q2).*cos(q3)+(-1).*sin(q1).*sin( ...
  q3))+cos(q1).*sin(q2).*sin(q4)).*sin(q5)).*sin(q7)).^(-2).*(cos(q7).*( ...
  cos(q6).*(cos(q5).*(cos(q4).*(cos(q2).*cos(q3).*sin(q1)+cos(q1).*sin(q3) ...
  )+sin(q1).*sin(q2).*sin(q4))+(cos(q1).*cos(q3)+(-1).*cos(q2).*sin(q1).* ...
  sin(q3)).*sin(q5))+((-1).*cos(q4).*sin(q1).*sin(q2)+(cos(q2).*cos(q3).* ...
  sin(q1)+cos(q1).*sin(q3)).*sin(q4)).*sin(q6))+(cos(q5).*(cos(q1).*cos( ...
  q3)+(-1).*cos(q2).*sin(q1).*sin(q3))+(-1).*(cos(q4).*(cos(q2).*cos(q3).* ...
  sin(q1)+cos(q1).*sin(q3))+sin(q1).*sin(q2).*sin(q4)).*sin(q5)).*sin(q7)) ...
  .^2).^(-2)+((-2).*cos(q7).^2.*(cos(q6).*((-1).*cos(q1).*cos(q4).*sin(q2) ...
  +(cos(q1).*cos(q2).*cos(q3)+(-1).*sin(q1).*sin(q3)).*sin(q4))+(-1).*( ...
  cos(q5).*(cos(q4).*(cos(q1).*cos(q2).*cos(q3)+(-1).*sin(q1).*sin(q3))+ ...
  cos(q1).*sin(q2).*sin(q4))+((-1).*cos(q3).*sin(q1)+(-1).*cos(q1).*cos( ...
  q2).*sin(q3)).*sin(q5)).*sin(q6)).*(cos(q6).*((-1).*cos(q4).*sin(q1).* ...
  sin(q2)+(cos(q2).*cos(q3).*sin(q1)+cos(q1).*sin(q3)).*sin(q4))+(-1).*( ...
  cos(q5).*(cos(q4).*(cos(q2).*cos(q3).*sin(q1)+cos(q1).*sin(q3))+sin(q1) ...
  .*sin(q2).*sin(q4))+(cos(q1).*cos(q3)+(-1).*cos(q2).*sin(q1).*sin(q3)).* ...
  sin(q5)).*sin(q6)).*(cos(q7).*(cos(q6).*(cos(q5).*(cos(q4).*(cos(q1).* ...
  cos(q2).*cos(q3)+(-1).*sin(q1).*sin(q3))+cos(q1).*sin(q2).*sin(q4))+(( ...
  -1).*cos(q3).*sin(q1)+(-1).*cos(q1).*cos(q2).*sin(q3)).*sin(q5))+((-1).* ...
  cos(q1).*cos(q4).*sin(q2)+(cos(q1).*cos(q2).*cos(q3)+(-1).*sin(q1).*sin( ...
  q3)).*sin(q4)).*sin(q6))+(cos(q5).*((-1).*cos(q3).*sin(q1)+(-1).*cos(q1) ...
  .*cos(q2).*sin(q3))+(-1).*(cos(q4).*(cos(q1).*cos(q2).*cos(q3)+(-1).* ...
  sin(q1).*sin(q3))+cos(q1).*sin(q2).*sin(q4)).*sin(q5)).*sin(q7)).^(-2)+ ...
  cos(q7).*((-1).*cos(q6).*(cos(q5).*(cos(q4).*(cos(q2).*cos(q3).*sin(q1)+ ...
  cos(q1).*sin(q3))+sin(q1).*sin(q2).*sin(q4))+(cos(q1).*cos(q3)+(-1).* ...
  cos(q2).*sin(q1).*sin(q3)).*sin(q5))+(-1).*((-1).*cos(q4).*sin(q1).*sin( ...
  q2)+(cos(q2).*cos(q3).*sin(q1)+cos(q1).*sin(q3)).*sin(q4)).*sin(q6)).*( ...
  cos(q7).*(cos(q6).*(cos(q5).*(cos(q4).*(cos(q1).*cos(q2).*cos(q3)+(-1).* ...
  sin(q1).*sin(q3))+cos(q1).*sin(q2).*sin(q4))+((-1).*cos(q3).*sin(q1)+( ...
  -1).*cos(q1).*cos(q2).*sin(q3)).*sin(q5))+((-1).*cos(q1).*cos(q4).*sin( ...
  q2)+(cos(q1).*cos(q2).*cos(q3)+(-1).*sin(q1).*sin(q3)).*sin(q4)).*sin( ...
  q6))+(cos(q5).*((-1).*cos(q3).*sin(q1)+(-1).*cos(q1).*cos(q2).*sin(q3))+ ...
  (-1).*(cos(q4).*(cos(q1).*cos(q2).*cos(q3)+(-1).*sin(q1).*sin(q3))+cos( ...
  q1).*sin(q2).*sin(q4)).*sin(q5)).*sin(q7)).^(-1)+2.*cos(q7).^2.*(cos(q6) ...
  .*((-1).*cos(q1).*cos(q4).*sin(q2)+(cos(q1).*cos(q2).*cos(q3)+(-1).*sin( ...
  q1).*sin(q3)).*sin(q4))+(-1).*(cos(q5).*(cos(q4).*(cos(q1).*cos(q2).* ...
  cos(q3)+(-1).*sin(q1).*sin(q3))+cos(q1).*sin(q2).*sin(q4))+((-1).*cos( ...
  q3).*sin(q1)+(-1).*cos(q1).*cos(q2).*sin(q3)).*sin(q5)).*sin(q6)).^2.*( ...
  cos(q7).*(cos(q6).*(cos(q5).*(cos(q4).*(cos(q1).*cos(q2).*cos(q3)+(-1).* ...
  sin(q1).*sin(q3))+cos(q1).*sin(q2).*sin(q4))+((-1).*cos(q3).*sin(q1)+( ...
  -1).*cos(q1).*cos(q2).*sin(q3)).*sin(q5))+((-1).*cos(q1).*cos(q4).*sin( ...
  q2)+(cos(q1).*cos(q2).*cos(q3)+(-1).*sin(q1).*sin(q3)).*sin(q4)).*sin( ...
  q6))+(cos(q5).*((-1).*cos(q3).*sin(q1)+(-1).*cos(q1).*cos(q2).*sin(q3))+ ...
  (-1).*(cos(q4).*(cos(q1).*cos(q2).*cos(q3)+(-1).*sin(q1).*sin(q3))+cos( ...
  q1).*sin(q2).*sin(q4)).*sin(q5)).*sin(q7)).^(-3).*(cos(q7).*(cos(q6).*( ...
  cos(q5).*(cos(q4).*(cos(q2).*cos(q3).*sin(q1)+cos(q1).*sin(q3))+sin(q1) ...
  .*sin(q2).*sin(q4))+(cos(q1).*cos(q3)+(-1).*cos(q2).*sin(q1).*sin(q3)).* ...
  sin(q5))+((-1).*cos(q4).*sin(q1).*sin(q2)+(cos(q2).*cos(q3).*sin(q1)+ ...
  cos(q1).*sin(q3)).*sin(q4)).*sin(q6))+(cos(q5).*(cos(q1).*cos(q3)+(-1).* ...
  cos(q2).*sin(q1).*sin(q3))+(-1).*(cos(q4).*(cos(q2).*cos(q3).*sin(q1)+ ...
  cos(q1).*sin(q3))+sin(q1).*sin(q2).*sin(q4)).*sin(q5)).*sin(q7))+(-1).* ...
  cos(q7).*((-1).*cos(q6).*(cos(q5).*(cos(q4).*(cos(q1).*cos(q2).*cos(q3)+ ...
  (-1).*sin(q1).*sin(q3))+cos(q1).*sin(q2).*sin(q4))+((-1).*cos(q3).*sin( ...
  q1)+(-1).*cos(q1).*cos(q2).*sin(q3)).*sin(q5))+(-1).*((-1).*cos(q1).* ...
  cos(q4).*sin(q2)+(cos(q1).*cos(q2).*cos(q3)+(-1).*sin(q1).*sin(q3)).* ...
  sin(q4)).*sin(q6)).*(cos(q7).*(cos(q6).*(cos(q5).*(cos(q4).*(cos(q1).* ...
  cos(q2).*cos(q3)+(-1).*sin(q1).*sin(q3))+cos(q1).*sin(q2).*sin(q4))+(( ...
  -1).*cos(q3).*sin(q1)+(-1).*cos(q1).*cos(q2).*sin(q3)).*sin(q5))+((-1).* ...
  cos(q1).*cos(q4).*sin(q2)+(cos(q1).*cos(q2).*cos(q3)+(-1).*sin(q1).*sin( ...
  q3)).*sin(q4)).*sin(q6))+(cos(q5).*((-1).*cos(q3).*sin(q1)+(-1).*cos(q1) ...
  .*cos(q2).*sin(q3))+(-1).*(cos(q4).*(cos(q1).*cos(q2).*cos(q3)+(-1).* ...
  sin(q1).*sin(q3))+cos(q1).*sin(q2).*sin(q4)).*sin(q5)).*sin(q7)).^(-2).* ...
  (cos(q7).*(cos(q6).*(cos(q5).*(cos(q4).*(cos(q2).*cos(q3).*sin(q1)+cos( ...
  q1).*sin(q3))+sin(q1).*sin(q2).*sin(q4))+(cos(q1).*cos(q3)+(-1).*cos(q2) ...
  .*sin(q1).*sin(q3)).*sin(q5))+((-1).*cos(q4).*sin(q1).*sin(q2)+(cos(q2) ...
  .*cos(q3).*sin(q1)+cos(q1).*sin(q3)).*sin(q4)).*sin(q6))+(cos(q5).*(cos( ...
  q1).*cos(q3)+(-1).*cos(q2).*sin(q1).*sin(q3))+(-1).*(cos(q4).*(cos(q2).* ...
  cos(q3).*sin(q1)+cos(q1).*sin(q3))+sin(q1).*sin(q2).*sin(q4)).*sin(q5)) ...
  .*sin(q7))).*(1+(cos(q7).*(cos(q6).*(cos(q5).*(cos(q4).*(cos(q1).*cos( ...
  q2).*cos(q3)+(-1).*sin(q1).*sin(q3))+cos(q1).*sin(q2).*sin(q4))+((-1).* ...
  cos(q3).*sin(q1)+(-1).*cos(q1).*cos(q2).*sin(q3)).*sin(q5))+((-1).*cos( ...
  q1).*cos(q4).*sin(q2)+(cos(q1).*cos(q2).*cos(q3)+(-1).*sin(q1).*sin(q3)) ...
  .*sin(q4)).*sin(q6))+(cos(q5).*((-1).*cos(q3).*sin(q1)+(-1).*cos(q1).* ...
  cos(q2).*sin(q3))+(-1).*(cos(q4).*(cos(q1).*cos(q2).*cos(q3)+(-1).*sin( ...
  q1).*sin(q3))+cos(q1).*sin(q2).*sin(q4)).*sin(q5)).*sin(q7)).^(-2).*( ...
  cos(q7).*(cos(q6).*(cos(q5).*(cos(q4).*(cos(q2).*cos(q3).*sin(q1)+cos( ...
  q1).*sin(q3))+sin(q1).*sin(q2).*sin(q4))+(cos(q1).*cos(q3)+(-1).*cos(q2) ...
  .*sin(q1).*sin(q3)).*sin(q5))+((-1).*cos(q4).*sin(q1).*sin(q2)+(cos(q2) ...
  .*cos(q3).*sin(q1)+cos(q1).*sin(q3)).*sin(q4)).*sin(q6))+(cos(q5).*(cos( ...
  q1).*cos(q3)+(-1).*cos(q2).*sin(q1).*sin(q3))+(-1).*(cos(q4).*(cos(q2).* ...
  cos(q3).*sin(q1)+cos(q1).*sin(q3))+sin(q1).*sin(q2).*sin(q4)).*sin(q5)) ...
  .*sin(q7)).^2).^(-1);

Jxe247 = (-1).*(1+(cos(q7).*(cos(q6).*(cos(q5).*(cos(q4).*( ...
  cos(q1).*cos(q2).*cos(q3)+(-1).*sin(q1).*sin(q3))+cos(q1).*sin(q2).*sin( ...
  q4))+((-1).*cos(q3).*sin(q1)+(-1).*cos(q1).*cos(q2).*sin(q3)).*sin(q5))+ ...
  ((-1).*cos(q1).*cos(q4).*sin(q2)+(cos(q1).*cos(q2).*cos(q3)+(-1).*sin( ...
  q1).*sin(q3)).*sin(q4)).*sin(q6))+(cos(q5).*((-1).*cos(q3).*sin(q1)+(-1) ...
  .*cos(q1).*cos(q2).*sin(q3))+(-1).*(cos(q4).*(cos(q1).*cos(q2).*cos(q3)+ ...
  (-1).*sin(q1).*sin(q3))+cos(q1).*sin(q2).*sin(q4)).*sin(q5)).*sin(q7)) ...
  .^(-2).*(cos(q7).*(cos(q6).*(cos(q5).*(cos(q4).*(cos(q2).*cos(q3).*sin( ...
  q1)+cos(q1).*sin(q3))+sin(q1).*sin(q2).*sin(q4))+(cos(q1).*cos(q3)+(-1) ...
  .*cos(q2).*sin(q1).*sin(q3)).*sin(q5))+((-1).*cos(q4).*sin(q1).*sin(q2)+ ...
  (cos(q2).*cos(q3).*sin(q1)+cos(q1).*sin(q3)).*sin(q4)).*sin(q6))+(cos( ...
  q5).*(cos(q1).*cos(q3)+(-1).*cos(q2).*sin(q1).*sin(q3))+(-1).*(cos(q4).* ...
  (cos(q2).*cos(q3).*sin(q1)+cos(q1).*sin(q3))+sin(q1).*sin(q2).*sin(q4)) ...
  .*sin(q5)).*sin(q7)).^2).^(-2).*((cos(q7).*(cos(q6).*(cos(q5).*(cos(q4) ...
  .*(cos(q1).*cos(q2).*cos(q3)+(-1).*sin(q1).*sin(q3))+cos(q1).*sin(q2).* ...
  sin(q4))+((-1).*cos(q3).*sin(q1)+(-1).*cos(q1).*cos(q2).*sin(q3)).*sin( ...
  q5))+((-1).*cos(q1).*cos(q4).*sin(q2)+(cos(q1).*cos(q2).*cos(q3)+(-1).* ...
  sin(q1).*sin(q3)).*sin(q4)).*sin(q6))+(cos(q5).*((-1).*cos(q3).*sin(q1)+ ...
  (-1).*cos(q1).*cos(q2).*sin(q3))+(-1).*(cos(q4).*(cos(q1).*cos(q2).*cos( ...
  q3)+(-1).*sin(q1).*sin(q3))+cos(q1).*sin(q2).*sin(q4)).*sin(q5)).*sin( ...
  q7)).^(-1).*(cos(q7).*(cos(q5).*(cos(q1).*cos(q3)+(-1).*cos(q2).*sin(q1) ...
  .*sin(q3))+(-1).*(cos(q4).*(cos(q2).*cos(q3).*sin(q1)+cos(q1).*sin(q3))+ ...
  sin(q1).*sin(q2).*sin(q4)).*sin(q5))+(-1).*(cos(q6).*(cos(q5).*(cos(q4) ...
  .*(cos(q2).*cos(q3).*sin(q1)+cos(q1).*sin(q3))+sin(q1).*sin(q2).*sin(q4) ...
  )+(cos(q1).*cos(q3)+(-1).*cos(q2).*sin(q1).*sin(q3)).*sin(q5))+((-1).* ...
  cos(q4).*sin(q1).*sin(q2)+(cos(q2).*cos(q3).*sin(q1)+cos(q1).*sin(q3)).* ...
  sin(q4)).*sin(q6)).*sin(q7))+(-1).*(cos(q7).*(cos(q6).*(cos(q5).*(cos( ...
  q4).*(cos(q1).*cos(q2).*cos(q3)+(-1).*sin(q1).*sin(q3))+cos(q1).*sin(q2) ...
  .*sin(q4))+((-1).*cos(q3).*sin(q1)+(-1).*cos(q1).*cos(q2).*sin(q3)).* ...
  sin(q5))+((-1).*cos(q1).*cos(q4).*sin(q2)+(cos(q1).*cos(q2).*cos(q3)+( ...
  -1).*sin(q1).*sin(q3)).*sin(q4)).*sin(q6))+(cos(q5).*((-1).*cos(q3).* ...
  sin(q1)+(-1).*cos(q1).*cos(q2).*sin(q3))+(-1).*(cos(q4).*(cos(q1).*cos( ...
  q2).*cos(q3)+(-1).*sin(q1).*sin(q3))+cos(q1).*sin(q2).*sin(q4)).*sin(q5) ...
  ).*sin(q7)).^(-2).*(cos(q7).*(cos(q6).*(cos(q5).*(cos(q4).*(cos(q2).* ...
  cos(q3).*sin(q1)+cos(q1).*sin(q3))+sin(q1).*sin(q2).*sin(q4))+(cos(q1).* ...
  cos(q3)+(-1).*cos(q2).*sin(q1).*sin(q3)).*sin(q5))+((-1).*cos(q4).*sin( ...
  q1).*sin(q2)+(cos(q2).*cos(q3).*sin(q1)+cos(q1).*sin(q3)).*sin(q4)).* ...
  sin(q6))+(cos(q5).*(cos(q1).*cos(q3)+(-1).*cos(q2).*sin(q1).*sin(q3))+( ...
  -1).*(cos(q4).*(cos(q2).*cos(q3).*sin(q1)+cos(q1).*sin(q3))+sin(q1).* ...
  sin(q2).*sin(q4)).*sin(q5)).*sin(q7)).*(cos(q7).*(cos(q5).*((-1).*cos( ...
  q3).*sin(q1)+(-1).*cos(q1).*cos(q2).*sin(q3))+(-1).*(cos(q4).*(cos(q1).* ...
  cos(q2).*cos(q3)+(-1).*sin(q1).*sin(q3))+cos(q1).*sin(q2).*sin(q4)).* ...
  sin(q5))+(-1).*(cos(q6).*(cos(q5).*(cos(q4).*(cos(q1).*cos(q2).*cos(q3)+ ...
  (-1).*sin(q1).*sin(q3))+cos(q1).*sin(q2).*sin(q4))+((-1).*cos(q3).*sin( ...
  q1)+(-1).*cos(q1).*cos(q2).*sin(q3)).*sin(q5))+((-1).*cos(q1).*cos(q4).* ...
  sin(q2)+(cos(q1).*cos(q2).*cos(q3)+(-1).*sin(q1).*sin(q3)).*sin(q4)).* ...
  sin(q6)).*sin(q7))).*(2.*(cos(q7).*(cos(q6).*(cos(q5).*(cos(q4).*(cos( ...
  q1).*cos(q2).*cos(q3)+(-1).*sin(q1).*sin(q3))+cos(q1).*sin(q2).*sin(q4)) ...
  +((-1).*cos(q3).*sin(q1)+(-1).*cos(q1).*cos(q2).*sin(q3)).*sin(q5))+(( ...
  -1).*cos(q1).*cos(q4).*sin(q2)+(cos(q1).*cos(q2).*cos(q3)+(-1).*sin(q1) ...
  .*sin(q3)).*sin(q4)).*sin(q6))+(cos(q5).*((-1).*cos(q3).*sin(q1)+(-1).* ...
  cos(q1).*cos(q2).*sin(q3))+(-1).*(cos(q4).*(cos(q1).*cos(q2).*cos(q3)+( ...
  -1).*sin(q1).*sin(q3))+cos(q1).*sin(q2).*sin(q4)).*sin(q5)).*sin(q7)).^( ...
  -2).*(cos(q7).*(cos(q6).*(cos(q5).*(cos(q4).*(cos(q2).*cos(q3).*sin(q1)+ ...
  cos(q1).*sin(q3))+sin(q1).*sin(q2).*sin(q4))+(cos(q1).*cos(q3)+(-1).* ...
  cos(q2).*sin(q1).*sin(q3)).*sin(q5))+((-1).*cos(q4).*sin(q1).*sin(q2)+( ...
  cos(q2).*cos(q3).*sin(q1)+cos(q1).*sin(q3)).*sin(q4)).*sin(q6))+(cos(q5) ...
  .*(cos(q1).*cos(q3)+(-1).*cos(q2).*sin(q1).*sin(q3))+(-1).*(cos(q4).*( ...
  cos(q2).*cos(q3).*sin(q1)+cos(q1).*sin(q3))+sin(q1).*sin(q2).*sin(q4)).* ...
  sin(q5)).*sin(q7)).*(cos(q7).*(cos(q5).*(cos(q1).*cos(q3)+(-1).*cos(q2) ...
  .*sin(q1).*sin(q3))+(-1).*(cos(q4).*(cos(q2).*cos(q3).*sin(q1)+cos(q1).* ...
  sin(q3))+sin(q1).*sin(q2).*sin(q4)).*sin(q5))+(-1).*(cos(q6).*(cos(q5).* ...
  (cos(q4).*(cos(q2).*cos(q3).*sin(q1)+cos(q1).*sin(q3))+sin(q1).*sin(q2) ...
  .*sin(q4))+(cos(q1).*cos(q3)+(-1).*cos(q2).*sin(q1).*sin(q3)).*sin(q5))+ ...
  ((-1).*cos(q4).*sin(q1).*sin(q2)+(cos(q2).*cos(q3).*sin(q1)+cos(q1).* ...
  sin(q3)).*sin(q4)).*sin(q6)).*sin(q7))+(-2).*(cos(q7).*(cos(q6).*(cos( ...
  q5).*(cos(q4).*(cos(q1).*cos(q2).*cos(q3)+(-1).*sin(q1).*sin(q3))+cos( ...
  q1).*sin(q2).*sin(q4))+((-1).*cos(q3).*sin(q1)+(-1).*cos(q1).*cos(q2).* ...
  sin(q3)).*sin(q5))+((-1).*cos(q1).*cos(q4).*sin(q2)+(cos(q1).*cos(q2).* ...
  cos(q3)+(-1).*sin(q1).*sin(q3)).*sin(q4)).*sin(q6))+(cos(q5).*((-1).* ...
  cos(q3).*sin(q1)+(-1).*cos(q1).*cos(q2).*sin(q3))+(-1).*(cos(q4).*(cos( ...
  q1).*cos(q2).*cos(q3)+(-1).*sin(q1).*sin(q3))+cos(q1).*sin(q2).*sin(q4)) ...
  .*sin(q5)).*sin(q7)).^(-3).*(cos(q7).*(cos(q6).*(cos(q5).*(cos(q4).*( ...
